simulink model "new_model"  (R2023a)
(part 2 of 4)

  RadarSensor:2.OBJ_S_Range_51 : Outport  Port=1335
  RadarSensor:2.OBJ_S_Range_52 : Outport  Port=1336
  RadarSensor:2.OBJ_S_Range_53 : Outport  Port=1337
  RadarSensor:2.OBJ_S_Range_54 : Outport  Port=1338
  RadarSensor:2.OBJ_S_Range_55 : Outport  Port=1339
  RadarSensor:2.OBJ_S_Range_56 : Outport  Port=1340
  RadarSensor:2.OBJ_S_Range_57 : Outport  Port=1341
  RadarSensor:2.OBJ_S_Range_58 : Outport  Port=1342
  RadarSensor:2.OBJ_S_Range_59 : Outport  Port=1343
  RadarSensor:2.OBJ_S_Range_60 : Outport  Port=1344
  RadarSensor:2.OBJ_S_Range_61 : Outport  Port=1345
  RadarSensor:2.OBJ_S_Range_62 : Outport  Port=1346
  RadarSensor:2.OBJ_S_Range_63 : Outport  Port=1347
  RadarSensor:2.OBJ_S_Range_64 : Outport  Port=1348
  RadarSensor:2.OBJ_RCS : Outport  Port=1349
  RadarSensor:2.OBJ_RCS_1 : Outport  Port=1350
  RadarSensor:2.OBJ_RCS_2 : Outport  Port=1351
  RadarSensor:2.OBJ_RCS_3 : Outport  Port=1352
  RadarSensor:2.OBJ_RCS_4 : Outport  Port=1353
  RadarSensor:2.OBJ_RCS_5 : Outport  Port=1354
  RadarSensor:2.OBJ_RCS_6 : Outport  Port=1355
  RadarSensor:2.OBJ_RCS_7 : Outport  Port=1356
  RadarSensor:2.OBJ_RCS_8 : Outport  Port=1357
  RadarSensor:2.OBJ_RCS_9 : Outport  Port=1358
  RadarSensor:2.OBJ_RCS_10 : Outport  Port=1359
  RadarSensor:2.OBJ_RCS_11 : Outport  Port=1360
  RadarSensor:2.OBJ_RCS_12 : Outport  Port=1361
  RadarSensor:2.OBJ_RCS_13 : Outport  Port=1362
  RadarSensor:2.OBJ_RCS_14 : Outport  Port=1363
  RadarSensor:2.OBJ_RCS_15 : Outport  Port=1364
  RadarSensor:2.OBJ_RCS_16 : Outport  Port=1365
  RadarSensor:2.OBJ_RCS_17 : Outport  Port=1366
  RadarSensor:2.OBJ_RCS_18 : Outport  Port=1367
  RadarSensor:2.OBJ_RCS_19 : Outport  Port=1368
  RadarSensor:2.OBJ_RCS_20 : Outport  Port=1369
  RadarSensor:2.OBJ_RCS_21 : Outport  Port=1370
  RadarSensor:2.OBJ_RCS_22 : Outport  Port=1371
  RadarSensor:2.OBJ_RCS_23 : Outport  Port=1372
  RadarSensor:2.OBJ_RCS_24 : Outport  Port=1373
  RadarSensor:2.OBJ_RCS_25 : Outport  Port=1374
  RadarSensor:2.OBJ_RCS_26 : Outport  Port=1375
  RadarSensor:2.OBJ_RCS_27 : Outport  Port=1376
  RadarSensor:2.OBJ_RCS_28 : Outport  Port=1377
  RadarSensor:2.OBJ_RCS_29 : Outport  Port=1378
  RadarSensor:2.OBJ_RCS_30 : Outport  Port=1379
  RadarSensor:2.OBJ_RCS_31 : Outport  Port=1380
  RadarSensor:2.OBJ_RCS_32 : Outport  Port=1381
  RadarSensor:2.OBJ_RCS_33 : Outport  Port=1382
  RadarSensor:2.OBJ_RCS_34 : Outport  Port=1383
  RadarSensor:2.OBJ_RCS_35 : Outport  Port=1384
  RadarSensor:2.OBJ_RCS_36 : Outport  Port=1385
  RadarSensor:2.OBJ_RCS_37 : Outport  Port=1386
  RadarSensor:2.OBJ_RCS_38 : Outport  Port=1387
  RadarSensor:2.OBJ_RCS_39 : Outport  Port=1388
  RadarSensor:2.OBJ_RCS_40 : Outport  Port=1389
  RadarSensor:2.OBJ_RCS_41 : Outport  Port=1390
  RadarSensor:2.OBJ_RCS_42 : Outport  Port=1391
  RadarSensor:2.OBJ_RCS_43 : Outport  Port=1392
  RadarSensor:2.OBJ_RCS_44 : Outport  Port=1393
  RadarSensor:2.OBJ_RCS_45 : Outport  Port=1394
  RadarSensor:2.OBJ_RCS_46 : Outport  Port=1395
  RadarSensor:2.OBJ_RCS_47 : Outport  Port=1396
  RadarSensor:2.OBJ_RCS_48 : Outport  Port=1397
  RadarSensor:2.OBJ_RCS_49 : Outport  Port=1398
  RadarSensor:2.OBJ_RCS_50 : Outport  Port=1399
  RadarSensor:2.OBJ_RCS_51 : Outport  Port=1400
  RadarSensor:2.OBJ_RCS_52 : Outport  Port=1401
  RadarSensor:2.OBJ_RCS_53 : Outport  Port=1402
  RadarSensor:2.OBJ_RCS_54 : Outport  Port=1403
  RadarSensor:2.OBJ_RCS_55 : Outport  Port=1404
  RadarSensor:2.OBJ_RCS_56 : Outport  Port=1405
  RadarSensor:2.OBJ_RCS_57 : Outport  Port=1406
  RadarSensor:2.OBJ_RCS_58 : Outport  Port=1407
  RadarSensor:2.OBJ_RCS_59 : Outport  Port=1408
  RadarSensor:2.OBJ_RCS_60 : Outport  Port=1409
  RadarSensor:2.OBJ_RCS_61 : Outport  Port=1410
  RadarSensor:2.OBJ_RCS_62 : Outport  Port=1411
  RadarSensor:2.OBJ_RCS_63 : Outport  Port=1412
  RadarSensor:2.OBJ_RCS_64 : Outport  Port=1413
  RadarSensor:3.time : Outport  Port=1414
  RadarSensor:3.width : Outport  Port=1415
  RadarSensor:3.OBJ_ID : Outport  Port=1416
  RadarSensor:3.OBJ_ID_1 : Outport  Port=1417
  RadarSensor:3.OBJ_ID_2 : Outport  Port=1418
  RadarSensor:3.OBJ_ID_3 : Outport  Port=1419
  RadarSensor:3.OBJ_ID_4 : Outport  Port=1420
  RadarSensor:3.OBJ_ID_5 : Outport  Port=1421
  RadarSensor:3.OBJ_ID_6 : Outport  Port=1422
  RadarSensor:3.OBJ_ID_7 : Outport  Port=1423
  RadarSensor:3.OBJ_ID_8 : Outport  Port=1424
  RadarSensor:3.OBJ_ID_9 : Outport  Port=1425
  RadarSensor:3.OBJ_ID_10 : Outport  Port=1426
  RadarSensor:3.OBJ_ID_11 : Outport  Port=1427
  RadarSensor:3.OBJ_ID_12 : Outport  Port=1428
  RadarSensor:3.OBJ_ID_13 : Outport  Port=1429
  RadarSensor:3.OBJ_ID_14 : Outport  Port=1430
  RadarSensor:3.OBJ_ID_15 : Outport  Port=1431
  RadarSensor:3.OBJ_ID_16 : Outport  Port=1432
  RadarSensor:3.OBJ_ID_17 : Outport  Port=1433
  RadarSensor:3.OBJ_ID_18 : Outport  Port=1434
  RadarSensor:3.OBJ_ID_19 : Outport  Port=1435
  RadarSensor:3.OBJ_ID_20 : Outport  Port=1436
  RadarSensor:3.OBJ_ID_21 : Outport  Port=1437
  RadarSensor:3.OBJ_ID_22 : Outport  Port=1438
  RadarSensor:3.OBJ_ID_23 : Outport  Port=1439
  RadarSensor:3.OBJ_ID_24 : Outport  Port=1440
  RadarSensor:3.OBJ_ID_25 : Outport  Port=1441
  RadarSensor:3.OBJ_ID_26 : Outport  Port=1442
  RadarSensor:3.OBJ_ID_27 : Outport  Port=1443
  RadarSensor:3.OBJ_ID_28 : Outport  Port=1444
  RadarSensor:3.OBJ_ID_29 : Outport  Port=1445
  RadarSensor:3.OBJ_ID_30 : Outport  Port=1446
  RadarSensor:3.OBJ_ID_31 : Outport  Port=1447
  RadarSensor:3.OBJ_ID_32 : Outport  Port=1448
  RadarSensor:3.OBJ_ID_33 : Outport  Port=1449
  RadarSensor:3.OBJ_ID_34 : Outport  Port=1450
  RadarSensor:3.OBJ_ID_35 : Outport  Port=1451
  RadarSensor:3.OBJ_ID_36 : Outport  Port=1452
  RadarSensor:3.OBJ_ID_37 : Outport  Port=1453
  RadarSensor:3.OBJ_ID_38 : Outport  Port=1454
  RadarSensor:3.OBJ_ID_39 : Outport  Port=1455
  RadarSensor:3.OBJ_ID_40 : Outport  Port=1456
  RadarSensor:3.OBJ_ID_41 : Outport  Port=1457
  RadarSensor:3.OBJ_ID_42 : Outport  Port=1458
  RadarSensor:3.OBJ_ID_43 : Outport  Port=1459
  RadarSensor:3.OBJ_ID_44 : Outport  Port=1460
  RadarSensor:3.OBJ_ID_45 : Outport  Port=1461
  RadarSensor:3.OBJ_ID_46 : Outport  Port=1462
  RadarSensor:3.OBJ_ID_47 : Outport  Port=1463
  RadarSensor:3.OBJ_ID_48 : Outport  Port=1464
  RadarSensor:3.OBJ_ID_49 : Outport  Port=1465
  RadarSensor:3.OBJ_ID_50 : Outport  Port=1466
  RadarSensor:3.OBJ_ID_51 : Outport  Port=1467
  RadarSensor:3.OBJ_ID_52 : Outport  Port=1468
  RadarSensor:3.OBJ_ID_53 : Outport  Port=1469
  RadarSensor:3.OBJ_ID_54 : Outport  Port=1470
  RadarSensor:3.OBJ_ID_55 : Outport  Port=1471
  RadarSensor:3.OBJ_ID_56 : Outport  Port=1472
  RadarSensor:3.OBJ_ID_57 : Outport  Port=1473
  RadarSensor:3.OBJ_ID_58 : Outport  Port=1474
  RadarSensor:3.OBJ_ID_59 : Outport  Port=1475
  RadarSensor:3.OBJ_ID_60 : Outport  Port=1476
  RadarSensor:3.OBJ_ID_61 : Outport  Port=1477
  RadarSensor:3.OBJ_ID_62 : Outport  Port=1478
  RadarSensor:3.OBJ_ID_63 : Outport  Port=1479
  RadarSensor:3.OBJ_ID_64 : Outport  Port=1480
  RadarSensor:3.OBJ_Class : Outport  Port=1481
  RadarSensor:3.OBJ_Class_1 : Outport  Port=1482
  RadarSensor:3.OBJ_Class_2 : Outport  Port=1483
  RadarSensor:3.OBJ_Class_3 : Outport  Port=1484
  RadarSensor:3.OBJ_Class_4 : Outport  Port=1485
  RadarSensor:3.OBJ_Class_5 : Outport  Port=1486
  RadarSensor:3.OBJ_Class_6 : Outport  Port=1487
  RadarSensor:3.OBJ_Class_7 : Outport  Port=1488
  RadarSensor:3.OBJ_Class_8 : Outport  Port=1489
  RadarSensor:3.OBJ_Class_9 : Outport  Port=1490
  RadarSensor:3.OBJ_Class_10 : Outport  Port=1491
  RadarSensor:3.OBJ_Class_11 : Outport  Port=1492
  RadarSensor:3.OBJ_Class_12 : Outport  Port=1493
  RadarSensor:3.OBJ_Class_13 : Outport  Port=1494
  RadarSensor:3.OBJ_Class_14 : Outport  Port=1495
  RadarSensor:3.OBJ_Class_15 : Outport  Port=1496
  RadarSensor:3.OBJ_Class_16 : Outport  Port=1497
  RadarSensor:3.OBJ_Class_17 : Outport  Port=1498
  RadarSensor:3.OBJ_Class_18 : Outport  Port=1499
  RadarSensor:3.OBJ_Class_19 : Outport  Port=1500
  RadarSensor:3.OBJ_Class_20 : Outport  Port=1501
  RadarSensor:3.OBJ_Class_21 : Outport  Port=1502
  RadarSensor:3.OBJ_Class_22 : Outport  Port=1503
  RadarSensor:3.OBJ_Class_23 : Outport  Port=1504
  RadarSensor:3.OBJ_Class_24 : Outport  Port=1505
  RadarSensor:3.OBJ_Class_25 : Outport  Port=1506
  RadarSensor:3.OBJ_Class_26 : Outport  Port=1507
  RadarSensor:3.OBJ_Class_27 : Outport  Port=1508
  RadarSensor:3.OBJ_Class_28 : Outport  Port=1509
  RadarSensor:3.OBJ_Class_29 : Outport  Port=1510
  RadarSensor:3.OBJ_Class_30 : Outport  Port=1511
  RadarSensor:3.OBJ_Class_31 : Outport  Port=1512
  RadarSensor:3.OBJ_Class_32 : Outport  Port=1513
  RadarSensor:3.OBJ_Class_33 : Outport  Port=1514
  RadarSensor:3.OBJ_Class_34 : Outport  Port=1515
  RadarSensor:3.OBJ_Class_35 : Outport  Port=1516
  RadarSensor:3.OBJ_Class_36 : Outport  Port=1517
  RadarSensor:3.OBJ_Class_37 : Outport  Port=1518
  RadarSensor:3.OBJ_Class_38 : Outport  Port=1519
  RadarSensor:3.OBJ_Class_39 : Outport  Port=1520
  RadarSensor:3.OBJ_Class_40 : Outport  Port=1521
  RadarSensor:3.OBJ_Class_41 : Outport  Port=1522
  RadarSensor:3.OBJ_Class_42 : Outport  Port=1523
  RadarSensor:3.OBJ_Class_43 : Outport  Port=1524
  RadarSensor:3.OBJ_Class_44 : Outport  Port=1525
  RadarSensor:3.OBJ_Class_45 : Outport  Port=1526
  RadarSensor:3.OBJ_Class_46 : Outport  Port=1527
  RadarSensor:3.OBJ_Class_47 : Outport  Port=1528
  RadarSensor:3.OBJ_Class_48 : Outport  Port=1529
  RadarSensor:3.OBJ_Class_49 : Outport  Port=1530
  RadarSensor:3.OBJ_Class_50 : Outport  Port=1531
  RadarSensor:3.OBJ_Class_51 : Outport  Port=1532
  RadarSensor:3.OBJ_Class_52 : Outport  Port=1533
  RadarSensor:3.OBJ_Class_53 : Outport  Port=1534
  RadarSensor:3.OBJ_Class_54 : Outport  Port=1535
  RadarSensor:3.OBJ_Class_55 : Outport  Port=1536
  RadarSensor:3.OBJ_Class_56 : Outport  Port=1537
  RadarSensor:3.OBJ_Class_57 : Outport  Port=1538
  RadarSensor:3.OBJ_Class_58 : Outport  Port=1539
  RadarSensor:3.OBJ_Class_59 : Outport  Port=1540
  RadarSensor:3.OBJ_Class_60 : Outport  Port=1541
  RadarSensor:3.OBJ_Class_61 : Outport  Port=1542
  RadarSensor:3.OBJ_Class_62 : Outport  Port=1543
  RadarSensor:3.OBJ_Class_63 : Outport  Port=1544
  RadarSensor:3.OBJ_Class_64 : Outport  Port=1545
  RadarSensor:3.OBJ_S_Azimuth : Outport  Port=1546
  RadarSensor:3.OBJ_S_Azimuth_1 : Outport  Port=1547
  RadarSensor:3.OBJ_S_Azimuth_2 : Outport  Port=1548
  RadarSensor:3.OBJ_S_Azimuth_3 : Outport  Port=1549
  RadarSensor:3.OBJ_S_Azimuth_4 : Outport  Port=1550
  RadarSensor:3.OBJ_S_Azimuth_5 : Outport  Port=1551
  RadarSensor:3.OBJ_S_Azimuth_6 : Outport  Port=1552
  RadarSensor:3.OBJ_S_Azimuth_7 : Outport  Port=1553
  RadarSensor:3.OBJ_S_Azimuth_8 : Outport  Port=1554
  RadarSensor:3.OBJ_S_Azimuth_9 : Outport  Port=1555
  RadarSensor:3.OBJ_S_Azimuth_10 : Outport  Port=1556
  RadarSensor:3.OBJ_S_Azimuth_11 : Outport  Port=1557
  RadarSensor:3.OBJ_S_Azimuth_12 : Outport  Port=1558
  RadarSensor:3.OBJ_S_Azimuth_13 : Outport  Port=1559
  RadarSensor:3.OBJ_S_Azimuth_14 : Outport  Port=1560
  RadarSensor:3.OBJ_S_Azimuth_15 : Outport  Port=1561
  RadarSensor:3.OBJ_S_Azimuth_16 : Outport  Port=1562
  RadarSensor:3.OBJ_S_Azimuth_17 : Outport  Port=1563
  RadarSensor:3.OBJ_S_Azimuth_18 : Outport  Port=1564
  RadarSensor:3.OBJ_S_Azimuth_19 : Outport  Port=1565
  RadarSensor:3.OBJ_S_Azimuth_20 : Outport  Port=1566
  RadarSensor:3.OBJ_S_Azimuth_21 : Outport  Port=1567
  RadarSensor:3.OBJ_S_Azimuth_22 : Outport  Port=1568
  RadarSensor:3.OBJ_S_Azimuth_23 : Outport  Port=1569
  RadarSensor:3.OBJ_S_Azimuth_24 : Outport  Port=1570
  RadarSensor:3.OBJ_S_Azimuth_25 : Outport  Port=1571
  RadarSensor:3.OBJ_S_Azimuth_26 : Outport  Port=1572
  RadarSensor:3.OBJ_S_Azimuth_27 : Outport  Port=1573
  RadarSensor:3.OBJ_S_Azimuth_28 : Outport  Port=1574
  RadarSensor:3.OBJ_S_Azimuth_29 : Outport  Port=1575
  RadarSensor:3.OBJ_S_Azimuth_30 : Outport  Port=1576
  RadarSensor:3.OBJ_S_Azimuth_31 : Outport  Port=1577
  RadarSensor:3.OBJ_S_Azimuth_32 : Outport  Port=1578
  RadarSensor:3.OBJ_S_Azimuth_33 : Outport  Port=1579
  RadarSensor:3.OBJ_S_Azimuth_34 : Outport  Port=1580
  RadarSensor:3.OBJ_S_Azimuth_35 : Outport  Port=1581
  RadarSensor:3.OBJ_S_Azimuth_36 : Outport  Port=1582
  RadarSensor:3.OBJ_S_Azimuth_37 : Outport  Port=1583
  RadarSensor:3.OBJ_S_Azimuth_38 : Outport  Port=1584
  RadarSensor:3.OBJ_S_Azimuth_39 : Outport  Port=1585
  RadarSensor:3.OBJ_S_Azimuth_40 : Outport  Port=1586
  RadarSensor:3.OBJ_S_Azimuth_41 : Outport  Port=1587
  RadarSensor:3.OBJ_S_Azimuth_42 : Outport  Port=1588
  RadarSensor:3.OBJ_S_Azimuth_43 : Outport  Port=1589
  RadarSensor:3.OBJ_S_Azimuth_44 : Outport  Port=1590
  RadarSensor:3.OBJ_S_Azimuth_45 : Outport  Port=1591
  RadarSensor:3.OBJ_S_Azimuth_46 : Outport  Port=1592
  RadarSensor:3.OBJ_S_Azimuth_47 : Outport  Port=1593
  RadarSensor:3.OBJ_S_Azimuth_48 : Outport  Port=1594
  RadarSensor:3.OBJ_S_Azimuth_49 : Outport  Port=1595
  RadarSensor:3.OBJ_S_Azimuth_50 : Outport  Port=1596
  RadarSensor:3.OBJ_S_Azimuth_51 : Outport  Port=1597
  RadarSensor:3.OBJ_S_Azimuth_52 : Outport  Port=1598
  RadarSensor:3.OBJ_S_Azimuth_53 : Outport  Port=1599
  RadarSensor:3.OBJ_S_Azimuth_54 : Outport  Port=1600
  RadarSensor:3.OBJ_S_Azimuth_55 : Outport  Port=1601
  RadarSensor:3.OBJ_S_Azimuth_56 : Outport  Port=1602
  RadarSensor:3.OBJ_S_Azimuth_57 : Outport  Port=1603
  RadarSensor:3.OBJ_S_Azimuth_58 : Outport  Port=1604
  RadarSensor:3.OBJ_S_Azimuth_59 : Outport  Port=1605
  RadarSensor:3.OBJ_S_Azimuth_60 : Outport  Port=1606
  RadarSensor:3.OBJ_S_Azimuth_61 : Outport  Port=1607
  RadarSensor:3.OBJ_S_Azimuth_62 : Outport  Port=1608
  RadarSensor:3.OBJ_S_Azimuth_63 : Outport  Port=1609
  RadarSensor:3.OBJ_S_Azimuth_64 : Outport  Port=1610
  RadarSensor:3.OBJ_S_Elevation : Outport  Port=1611
  RadarSensor:3.OBJ_S_Elevation_1 : Outport  Port=1612
  RadarSensor:3.OBJ_S_Elevation_2 : Outport  Port=1613
  RadarSensor:3.OBJ_S_Elevation_3 : Outport  Port=1614
  RadarSensor:3.OBJ_S_Elevation_4 : Outport  Port=1615
  RadarSensor:3.OBJ_S_Elevation_5 : Outport  Port=1616
  RadarSensor:3.OBJ_S_Elevation_6 : Outport  Port=1617
  RadarSensor:3.OBJ_S_Elevation_7 : Outport  Port=1618
  RadarSensor:3.OBJ_S_Elevation_8 : Outport  Port=1619
  RadarSensor:3.OBJ_S_Elevation_9 : Outport  Port=1620
  RadarSensor:3.OBJ_S_Elevation_10 : Outport  Port=1621
  RadarSensor:3.OBJ_S_Elevation_11 : Outport  Port=1622
  RadarSensor:3.OBJ_S_Elevation_12 : Outport  Port=1623
  RadarSensor:3.OBJ_S_Elevation_13 : Outport  Port=1624
  RadarSensor:3.OBJ_S_Elevation_14 : Outport  Port=1625
  RadarSensor:3.OBJ_S_Elevation_15 : Outport  Port=1626
  RadarSensor:3.OBJ_S_Elevation_16 : Outport  Port=1627
  RadarSensor:3.OBJ_S_Elevation_17 : Outport  Port=1628
  RadarSensor:3.OBJ_S_Elevation_18 : Outport  Port=1629
  RadarSensor:3.OBJ_S_Elevation_19 : Outport  Port=1630
  RadarSensor:3.OBJ_S_Elevation_20 : Outport  Port=1631
  RadarSensor:3.OBJ_S_Elevation_21 : Outport  Port=1632
  RadarSensor:3.OBJ_S_Elevation_22 : Outport  Port=1633
  RadarSensor:3.OBJ_S_Elevation_23 : Outport  Port=1634
  RadarSensor:3.OBJ_S_Elevation_24 : Outport  Port=1635
  RadarSensor:3.OBJ_S_Elevation_25 : Outport  Port=1636
  RadarSensor:3.OBJ_S_Elevation_26 : Outport  Port=1637
  RadarSensor:3.OBJ_S_Elevation_27 : Outport  Port=1638
  RadarSensor:3.OBJ_S_Elevation_28 : Outport  Port=1639
  RadarSensor:3.OBJ_S_Elevation_29 : Outport  Port=1640
  RadarSensor:3.OBJ_S_Elevation_30 : Outport  Port=1641
  RadarSensor:3.OBJ_S_Elevation_31 : Outport  Port=1642
  RadarSensor:3.OBJ_S_Elevation_32 : Outport  Port=1643
  RadarSensor:3.OBJ_S_Elevation_33 : Outport  Port=1644
  RadarSensor:3.OBJ_S_Elevation_34 : Outport  Port=1645
  RadarSensor:3.OBJ_S_Elevation_35 : Outport  Port=1646
  RadarSensor:3.OBJ_S_Elevation_36 : Outport  Port=1647
  RadarSensor:3.OBJ_S_Elevation_37 : Outport  Port=1648
  RadarSensor:3.OBJ_S_Elevation_38 : Outport  Port=1649
  RadarSensor:3.OBJ_S_Elevation_39 : Outport  Port=1650
  RadarSensor:3.OBJ_S_Elevation_40 : Outport  Port=1651
  RadarSensor:3.OBJ_S_Elevation_41 : Outport  Port=1652
  RadarSensor:3.OBJ_S_Elevation_42 : Outport  Port=1653
  RadarSensor:3.OBJ_S_Elevation_43 : Outport  Port=1654
  RadarSensor:3.OBJ_S_Elevation_44 : Outport  Port=1655
  RadarSensor:3.OBJ_S_Elevation_45 : Outport  Port=1656
  RadarSensor:3.OBJ_S_Elevation_46 : Outport  Port=1657
  RadarSensor:3.OBJ_S_Elevation_47 : Outport  Port=1658
  RadarSensor:3.OBJ_S_Elevation_48 : Outport  Port=1659
  RadarSensor:3.OBJ_S_Elevation_49 : Outport  Port=1660
  RadarSensor:3.OBJ_S_Elevation_50 : Outport  Port=1661
  RadarSensor:3.OBJ_S_Elevation_51 : Outport  Port=1662
  RadarSensor:3.OBJ_S_Elevation_52 : Outport  Port=1663
  RadarSensor:3.OBJ_S_Elevation_53 : Outport  Port=1664
  RadarSensor:3.OBJ_S_Elevation_54 : Outport  Port=1665
  RadarSensor:3.OBJ_S_Elevation_55 : Outport  Port=1666
  RadarSensor:3.OBJ_S_Elevation_56 : Outport  Port=1667
  RadarSensor:3.OBJ_S_Elevation_57 : Outport  Port=1668
  RadarSensor:3.OBJ_S_Elevation_58 : Outport  Port=1669
  RadarSensor:3.OBJ_S_Elevation_59 : Outport  Port=1670
  RadarSensor:3.OBJ_S_Elevation_60 : Outport  Port=1671
  RadarSensor:3.OBJ_S_Elevation_61 : Outport  Port=1672
  RadarSensor:3.OBJ_S_Elevation_62 : Outport  Port=1673
  RadarSensor:3.OBJ_S_Elevation_63 : Outport  Port=1674
  RadarSensor:3.OBJ_S_Elevation_64 : Outport  Port=1675
  RadarSensor:3.OBJ_S_Velocity : Outport  Port=1676
  RadarSensor:3.OBJ_S_Velocity_1 : Outport  Port=1677
  RadarSensor:3.OBJ_S_Velocity_2 : Outport  Port=1678
  RadarSensor:3.OBJ_S_Velocity_3 : Outport  Port=1679
  RadarSensor:3.OBJ_S_Velocity_4 : Outport  Port=1680
  RadarSensor:3.OBJ_S_Velocity_5 : Outport  Port=1681
  RadarSensor:3.OBJ_S_Velocity_6 : Outport  Port=1682
  RadarSensor:3.OBJ_S_Velocity_7 : Outport  Port=1683
  RadarSensor:3.OBJ_S_Velocity_8 : Outport  Port=1684
  RadarSensor:3.OBJ_S_Velocity_9 : Outport  Port=1685
  RadarSensor:3.OBJ_S_Velocity_10 : Outport  Port=1686
  RadarSensor:3.OBJ_S_Velocity_11 : Outport  Port=1687
  RadarSensor:3.OBJ_S_Velocity_12 : Outport  Port=1688
  RadarSensor:3.OBJ_S_Velocity_13 : Outport  Port=1689
  RadarSensor:3.OBJ_S_Velocity_14 : Outport  Port=1690
  RadarSensor:3.OBJ_S_Velocity_15 : Outport  Port=1691
  RadarSensor:3.OBJ_S_Velocity_16 : Outport  Port=1692
  RadarSensor:3.OBJ_S_Velocity_17 : Outport  Port=1693
  RadarSensor:3.OBJ_S_Velocity_18 : Outport  Port=1694
  RadarSensor:3.OBJ_S_Velocity_19 : Outport  Port=1695
  RadarSensor:3.OBJ_S_Velocity_20 : Outport  Port=1696
  RadarSensor:3.OBJ_S_Velocity_21 : Outport  Port=1697
  RadarSensor:3.OBJ_S_Velocity_22 : Outport  Port=1698
  RadarSensor:3.OBJ_S_Velocity_23 : Outport  Port=1699
  RadarSensor:3.OBJ_S_Velocity_24 : Outport  Port=1700
  RadarSensor:3.OBJ_S_Velocity_25 : Outport  Port=1701
  RadarSensor:3.OBJ_S_Velocity_26 : Outport  Port=1702
  RadarSensor:3.OBJ_S_Velocity_27 : Outport  Port=1703
  RadarSensor:3.OBJ_S_Velocity_28 : Outport  Port=1704
  RadarSensor:3.OBJ_S_Velocity_29 : Outport  Port=1705
  RadarSensor:3.OBJ_S_Velocity_30 : Outport  Port=1706
  RadarSensor:3.OBJ_S_Velocity_31 : Outport  Port=1707
  RadarSensor:3.OBJ_S_Velocity_32 : Outport  Port=1708
  RadarSensor:3.OBJ_S_Velocity_33 : Outport  Port=1709
  RadarSensor:3.OBJ_S_Velocity_34 : Outport  Port=1710
  RadarSensor:3.OBJ_S_Velocity_35 : Outport  Port=1711
  RadarSensor:3.OBJ_S_Velocity_36 : Outport  Port=1712
  RadarSensor:3.OBJ_S_Velocity_37 : Outport  Port=1713
  RadarSensor:3.OBJ_S_Velocity_38 : Outport  Port=1714
  RadarSensor:3.OBJ_S_Velocity_39 : Outport  Port=1715
  RadarSensor:3.OBJ_S_Velocity_40 : Outport  Port=1716
  RadarSensor:3.OBJ_S_Velocity_41 : Outport  Port=1717
  RadarSensor:3.OBJ_S_Velocity_42 : Outport  Port=1718
  RadarSensor:3.OBJ_S_Velocity_43 : Outport  Port=1719
  RadarSensor:3.OBJ_S_Velocity_44 : Outport  Port=1720
  RadarSensor:3.OBJ_S_Velocity_45 : Outport  Port=1721
  RadarSensor:3.OBJ_S_Velocity_46 : Outport  Port=1722
  RadarSensor:3.OBJ_S_Velocity_47 : Outport  Port=1723
  RadarSensor:3.OBJ_S_Velocity_48 : Outport  Port=1724
  RadarSensor:3.OBJ_S_Velocity_49 : Outport  Port=1725
  RadarSensor:3.OBJ_S_Velocity_50 : Outport  Port=1726
  RadarSensor:3.OBJ_S_Velocity_51 : Outport  Port=1727
  RadarSensor:3.OBJ_S_Velocity_52 : Outport  Port=1728
  RadarSensor:3.OBJ_S_Velocity_53 : Outport  Port=1729
  RadarSensor:3.OBJ_S_Velocity_54 : Outport  Port=1730
  RadarSensor:3.OBJ_S_Velocity_55 : Outport  Port=1731
  RadarSensor:3.OBJ_S_Velocity_56 : Outport  Port=1732
  RadarSensor:3.OBJ_S_Velocity_57 : Outport  Port=1733
  RadarSensor:3.OBJ_S_Velocity_58 : Outport  Port=1734
  RadarSensor:3.OBJ_S_Velocity_59 : Outport  Port=1735
  RadarSensor:3.OBJ_S_Velocity_60 : Outport  Port=1736
  RadarSensor:3.OBJ_S_Velocity_61 : Outport  Port=1737
  RadarSensor:3.OBJ_S_Velocity_62 : Outport  Port=1738
  RadarSensor:3.OBJ_S_Velocity_63 : Outport  Port=1739
  RadarSensor:3.OBJ_S_Velocity_64 : Outport  Port=1740
  RadarSensor:3.OBJ_S_Range : Outport  Port=1741
  RadarSensor:3.OBJ_S_Range_1 : Outport  Port=1742
  RadarSensor:3.OBJ_S_Range_2 : Outport  Port=1743
  RadarSensor:3.OBJ_S_Range_3 : Outport  Port=1744
  RadarSensor:3.OBJ_S_Range_4 : Outport  Port=1745
  RadarSensor:3.OBJ_S_Range_5 : Outport  Port=1746
  RadarSensor:3.OBJ_S_Range_6 : Outport  Port=1747
  RadarSensor:3.OBJ_S_Range_7 : Outport  Port=1748
  RadarSensor:3.OBJ_S_Range_8 : Outport  Port=1749
  RadarSensor:3.OBJ_S_Range_9 : Outport  Port=1750
  RadarSensor:3.OBJ_S_Range_10 : Outport  Port=1751
  RadarSensor:3.OBJ_S_Range_11 : Outport  Port=1752
  RadarSensor:3.OBJ_S_Range_12 : Outport  Port=1753
  RadarSensor:3.OBJ_S_Range_13 : Outport  Port=1754
  RadarSensor:3.OBJ_S_Range_14 : Outport  Port=1755
  RadarSensor:3.OBJ_S_Range_15 : Outport  Port=1756
  RadarSensor:3.OBJ_S_Range_16 : Outport  Port=1757
  RadarSensor:3.OBJ_S_Range_17 : Outport  Port=1758
  RadarSensor:3.OBJ_S_Range_18 : Outport  Port=1759
  RadarSensor:3.OBJ_S_Range_19 : Outport  Port=1760
  RadarSensor:3.OBJ_S_Range_20 : Outport  Port=1761
  RadarSensor:3.OBJ_S_Range_21 : Outport  Port=1762
  RadarSensor:3.OBJ_S_Range_22 : Outport  Port=1763
  RadarSensor:3.OBJ_S_Range_23 : Outport  Port=1764
  RadarSensor:3.OBJ_S_Range_24 : Outport  Port=1765
  RadarSensor:3.OBJ_S_Range_25 : Outport  Port=1766
  RadarSensor:3.OBJ_S_Range_26 : Outport  Port=1767
  RadarSensor:3.OBJ_S_Range_27 : Outport  Port=1768
  RadarSensor:3.OBJ_S_Range_28 : Outport  Port=1769
  RadarSensor:3.OBJ_S_Range_29 : Outport  Port=1770
  RadarSensor:3.OBJ_S_Range_30 : Outport  Port=1771
  RadarSensor:3.OBJ_S_Range_31 : Outport  Port=1772
  RadarSensor:3.OBJ_S_Range_32 : Outport  Port=1773
  RadarSensor:3.OBJ_S_Range_33 : Outport  Port=1774
  RadarSensor:3.OBJ_S_Range_34 : Outport  Port=1775
  RadarSensor:3.OBJ_S_Range_35 : Outport  Port=1776
  RadarSensor:3.OBJ_S_Range_36 : Outport  Port=1777
  RadarSensor:3.OBJ_S_Range_37 : Outport  Port=1778
  RadarSensor:3.OBJ_S_Range_38 : Outport  Port=1779
  RadarSensor:3.OBJ_S_Range_39 : Outport  Port=1780
  RadarSensor:3.OBJ_S_Range_40 : Outport  Port=1781
  RadarSensor:3.OBJ_S_Range_41 : Outport  Port=1782
  RadarSensor:3.OBJ_S_Range_42 : Outport  Port=1783
  RadarSensor:3.OBJ_S_Range_43 : Outport  Port=1784
  RadarSensor:3.OBJ_S_Range_44 : Outport  Port=1785
  RadarSensor:3.OBJ_S_Range_45 : Outport  Port=1786
  RadarSensor:3.OBJ_S_Range_46 : Outport  Port=1787
  RadarSensor:3.OBJ_S_Range_47 : Outport  Port=1788
  RadarSensor:3.OBJ_S_Range_48 : Outport  Port=1789
  RadarSensor:3.OBJ_S_Range_49 : Outport  Port=1790
  RadarSensor:3.OBJ_S_Range_50 : Outport  Port=1791
  RadarSensor:3.OBJ_S_Range_51 : Outport  Port=1792
  RadarSensor:3.OBJ_S_Range_52 : Outport  Port=1793
  RadarSensor:3.OBJ_S_Range_53 : Outport  Port=1794
  RadarSensor:3.OBJ_S_Range_54 : Outport  Port=1795
  RadarSensor:3.OBJ_S_Range_55 : Outport  Port=1796
  RadarSensor:3.OBJ_S_Range_56 : Outport  Port=1797
  RadarSensor:3.OBJ_S_Range_57 : Outport  Port=1798
  RadarSensor:3.OBJ_S_Range_58 : Outport  Port=1799
  RadarSensor:3.OBJ_S_Range_59 : Outport  Port=1800
  RadarSensor:3.OBJ_S_Range_60 : Outport  Port=1801
  RadarSensor:3.OBJ_S_Range_61 : Outport  Port=1802
  RadarSensor:3.OBJ_S_Range_62 : Outport  Port=1803
  RadarSensor:3.OBJ_S_Range_63 : Outport  Port=1804
  RadarSensor:3.OBJ_S_Range_64 : Outport  Port=1805
  RadarSensor:3.OBJ_RCS : Outport  Port=1806
  RadarSensor:3.OBJ_RCS_1 : Outport  Port=1807
  RadarSensor:3.OBJ_RCS_2 : Outport  Port=1808
  RadarSensor:3.OBJ_RCS_3 : Outport  Port=1809
  RadarSensor:3.OBJ_RCS_4 : Outport  Port=1810
  RadarSensor:3.OBJ_RCS_5 : Outport  Port=1811
  RadarSensor:3.OBJ_RCS_6 : Outport  Port=1812
  RadarSensor:3.OBJ_RCS_7 : Outport  Port=1813
  RadarSensor:3.OBJ_RCS_8 : Outport  Port=1814
  RadarSensor:3.OBJ_RCS_9 : Outport  Port=1815
  RadarSensor:3.OBJ_RCS_10 : Outport  Port=1816
  RadarSensor:3.OBJ_RCS_11 : Outport  Port=1817
  RadarSensor:3.OBJ_RCS_12 : Outport  Port=1818
  RadarSensor:3.OBJ_RCS_13 : Outport  Port=1819
  RadarSensor:3.OBJ_RCS_14 : Outport  Port=1820
  RadarSensor:3.OBJ_RCS_15 : Outport  Port=1821
  RadarSensor:3.OBJ_RCS_16 : Outport  Port=1822
  RadarSensor:3.OBJ_RCS_17 : Outport  Port=1823
  RadarSensor:3.OBJ_RCS_18 : Outport  Port=1824
  RadarSensor:3.OBJ_RCS_19 : Outport  Port=1825
  RadarSensor:3.OBJ_RCS_20 : Outport  Port=1826
  RadarSensor:3.OBJ_RCS_21 : Outport  Port=1827
  RadarSensor:3.OBJ_RCS_22 : Outport  Port=1828
  RadarSensor:3.OBJ_RCS_23 : Outport  Port=1829
  RadarSensor:3.OBJ_RCS_24 : Outport  Port=1830
  RadarSensor:3.OBJ_RCS_25 : Outport  Port=1831
  RadarSensor:3.OBJ_RCS_26 : Outport  Port=1832
  RadarSensor:3.OBJ_RCS_27 : Outport  Port=1833
  RadarSensor:3.OBJ_RCS_28 : Outport  Port=1834
  RadarSensor:3.OBJ_RCS_29 : Outport  Port=1835
  RadarSensor:3.OBJ_RCS_30 : Outport  Port=1836
  RadarSensor:3.OBJ_RCS_31 : Outport  Port=1837
  RadarSensor:3.OBJ_RCS_32 : Outport  Port=1838
  RadarSensor:3.OBJ_RCS_33 : Outport  Port=1839
  RadarSensor:3.OBJ_RCS_34 : Outport  Port=1840
  RadarSensor:3.OBJ_RCS_35 : Outport  Port=1841
  RadarSensor:3.OBJ_RCS_36 : Outport  Port=1842
  RadarSensor:3.OBJ_RCS_37 : Outport  Port=1843
  RadarSensor:3.OBJ_RCS_38 : Outport  Port=1844
  RadarSensor:3.OBJ_RCS_39 : Outport  Port=1845
  RadarSensor:3.OBJ_RCS_40 : Outport  Port=1846
  RadarSensor:3.OBJ_RCS_41 : Outport  Port=1847
  RadarSensor:3.OBJ_RCS_42 : Outport  Port=1848
  RadarSensor:3.OBJ_RCS_43 : Outport  Port=1849
  RadarSensor:3.OBJ_RCS_44 : Outport  Port=1850
  RadarSensor:3.OBJ_RCS_45 : Outport  Port=1851
  RadarSensor:3.OBJ_RCS_46 : Outport  Port=1852
  RadarSensor:3.OBJ_RCS_47 : Outport  Port=1853
  RadarSensor:3.OBJ_RCS_48 : Outport  Port=1854
  RadarSensor:3.OBJ_RCS_49 : Outport  Port=1855
  RadarSensor:3.OBJ_RCS_50 : Outport  Port=1856
  RadarSensor:3.OBJ_RCS_51 : Outport  Port=1857
  RadarSensor:3.OBJ_RCS_52 : Outport  Port=1858
  RadarSensor:3.OBJ_RCS_53 : Outport  Port=1859
  RadarSensor:3.OBJ_RCS_54 : Outport  Port=1860
  RadarSensor:3.OBJ_RCS_55 : Outport  Port=1861
  RadarSensor:3.OBJ_RCS_56 : Outport  Port=1862
  RadarSensor:3.OBJ_RCS_57 : Outport  Port=1863
  RadarSensor:3.OBJ_RCS_58 : Outport  Port=1864
  RadarSensor:3.OBJ_RCS_59 : Outport  Port=1865
  RadarSensor:3.OBJ_RCS_60 : Outport  Port=1866
  RadarSensor:3.OBJ_RCS_61 : Outport  Port=1867
  RadarSensor:3.OBJ_RCS_62 : Outport  Port=1868
  RadarSensor:3.OBJ_RCS_63 : Outport  Port=1869
  RadarSensor:3.OBJ_RCS_64 : Outport  Port=1870
  RadarSensor:4.time : Outport  Port=1871
  RadarSensor:4.width : Outport  Port=1872
  RadarSensor:4.OBJ_ID : Outport  Port=1873
  RadarSensor:4.OBJ_ID_1 : Outport  Port=1874
  RadarSensor:4.OBJ_ID_2 : Outport  Port=1875
  RadarSensor:4.OBJ_ID_3 : Outport  Port=1876
  RadarSensor:4.OBJ_ID_4 : Outport  Port=1877
  RadarSensor:4.OBJ_ID_5 : Outport  Port=1878
  RadarSensor:4.OBJ_ID_6 : Outport  Port=1879
  RadarSensor:4.OBJ_ID_7 : Outport  Port=1880
  RadarSensor:4.OBJ_ID_8 : Outport  Port=1881
  RadarSensor:4.OBJ_ID_9 : Outport  Port=1882
  RadarSensor:4.OBJ_ID_10 : Outport  Port=1883
  RadarSensor:4.OBJ_ID_11 : Outport  Port=1884
  RadarSensor:4.OBJ_ID_12 : Outport  Port=1885
  RadarSensor:4.OBJ_ID_13 : Outport  Port=1886
  RadarSensor:4.OBJ_ID_14 : Outport  Port=1887
  RadarSensor:4.OBJ_ID_15 : Outport  Port=1888
  RadarSensor:4.OBJ_ID_16 : Outport  Port=1889
  RadarSensor:4.OBJ_ID_17 : Outport  Port=1890
  RadarSensor:4.OBJ_ID_18 : Outport  Port=1891
  RadarSensor:4.OBJ_ID_19 : Outport  Port=1892
  RadarSensor:4.OBJ_ID_20 : Outport  Port=1893
  RadarSensor:4.OBJ_ID_21 : Outport  Port=1894
  RadarSensor:4.OBJ_ID_22 : Outport  Port=1895
  RadarSensor:4.OBJ_ID_23 : Outport  Port=1896
  RadarSensor:4.OBJ_ID_24 : Outport  Port=1897
  RadarSensor:4.OBJ_ID_25 : Outport  Port=1898
  RadarSensor:4.OBJ_ID_26 : Outport  Port=1899
  RadarSensor:4.OBJ_ID_27 : Outport  Port=1900
  RadarSensor:4.OBJ_ID_28 : Outport  Port=1901
  RadarSensor:4.OBJ_ID_29 : Outport  Port=1902
  RadarSensor:4.OBJ_ID_30 : Outport  Port=1903
  RadarSensor:4.OBJ_ID_31 : Outport  Port=1904
  RadarSensor:4.OBJ_ID_32 : Outport  Port=1905
  RadarSensor:4.OBJ_ID_33 : Outport  Port=1906
  RadarSensor:4.OBJ_ID_34 : Outport  Port=1907
  RadarSensor:4.OBJ_ID_35 : Outport  Port=1908
  RadarSensor:4.OBJ_ID_36 : Outport  Port=1909
  RadarSensor:4.OBJ_ID_37 : Outport  Port=1910
  RadarSensor:4.OBJ_ID_38 : Outport  Port=1911
  RadarSensor:4.OBJ_ID_39 : Outport  Port=1912
  RadarSensor:4.OBJ_ID_40 : Outport  Port=1913
  RadarSensor:4.OBJ_ID_41 : Outport  Port=1914
  RadarSensor:4.OBJ_ID_42 : Outport  Port=1915
  RadarSensor:4.OBJ_ID_43 : Outport  Port=1916
  RadarSensor:4.OBJ_ID_44 : Outport  Port=1917
  RadarSensor:4.OBJ_ID_45 : Outport  Port=1918
  RadarSensor:4.OBJ_ID_46 : Outport  Port=1919
  RadarSensor:4.OBJ_ID_47 : Outport  Port=1920
  RadarSensor:4.OBJ_ID_48 : Outport  Port=1921
  RadarSensor:4.OBJ_ID_49 : Outport  Port=1922
  RadarSensor:4.OBJ_ID_50 : Outport  Port=1923
  RadarSensor:4.OBJ_ID_51 : Outport  Port=1924
  RadarSensor:4.OBJ_ID_52 : Outport  Port=1925
  RadarSensor:4.OBJ_ID_53 : Outport  Port=1926
  RadarSensor:4.OBJ_ID_54 : Outport  Port=1927
  RadarSensor:4.OBJ_ID_55 : Outport  Port=1928
  RadarSensor:4.OBJ_ID_56 : Outport  Port=1929
  RadarSensor:4.OBJ_ID_57 : Outport  Port=1930
  RadarSensor:4.OBJ_ID_58 : Outport  Port=1931
  RadarSensor:4.OBJ_ID_59 : Outport  Port=1932
  RadarSensor:4.OBJ_ID_60 : Outport  Port=1933
  RadarSensor:4.OBJ_ID_61 : Outport  Port=1934
  RadarSensor:4.OBJ_ID_62 : Outport  Port=1935
  RadarSensor:4.OBJ_ID_63 : Outport  Port=1936
  RadarSensor:4.OBJ_ID_64 : Outport  Port=1937
  RadarSensor:4.OBJ_Class : Outport  Port=1938
  RadarSensor:4.OBJ_Class_1 : Outport  Port=1939
  RadarSensor:4.OBJ_Class_2 : Outport  Port=1940
  RadarSensor:4.OBJ_Class_3 : Outport  Port=1941
  RadarSensor:4.OBJ_Class_4 : Outport  Port=1942
  RadarSensor:4.OBJ_Class_5 : Outport  Port=1943
  RadarSensor:4.OBJ_Class_6 : Outport  Port=1944
  RadarSensor:4.OBJ_Class_7 : Outport  Port=1945
  RadarSensor:4.OBJ_Class_8 : Outport  Port=1946
  RadarSensor:4.OBJ_Class_9 : Outport  Port=1947
  RadarSensor:4.OBJ_Class_10 : Outport  Port=1948
  RadarSensor:4.OBJ_Class_11 : Outport  Port=1949
  RadarSensor:4.OBJ_Class_12 : Outport  Port=1950
  RadarSensor:4.OBJ_Class_13 : Outport  Port=1951
  RadarSensor:4.OBJ_Class_14 : Outport  Port=1952
  RadarSensor:4.OBJ_Class_15 : Outport  Port=1953
  RadarSensor:4.OBJ_Class_16 : Outport  Port=1954
  RadarSensor:4.OBJ_Class_17 : Outport  Port=1955
  RadarSensor:4.OBJ_Class_18 : Outport  Port=1956
  RadarSensor:4.OBJ_Class_19 : Outport  Port=1957
  RadarSensor:4.OBJ_Class_20 : Outport  Port=1958
  RadarSensor:4.OBJ_Class_21 : Outport  Port=1959
  RadarSensor:4.OBJ_Class_22 : Outport  Port=1960
  RadarSensor:4.OBJ_Class_23 : Outport  Port=1961
  RadarSensor:4.OBJ_Class_24 : Outport  Port=1962
  RadarSensor:4.OBJ_Class_25 : Outport  Port=1963
  RadarSensor:4.OBJ_Class_26 : Outport  Port=1964
  RadarSensor:4.OBJ_Class_27 : Outport  Port=1965
  RadarSensor:4.OBJ_Class_28 : Outport  Port=1966
  RadarSensor:4.OBJ_Class_29 : Outport  Port=1967
  RadarSensor:4.OBJ_Class_30 : Outport  Port=1968
  RadarSensor:4.OBJ_Class_31 : Outport  Port=1969
  RadarSensor:4.OBJ_Class_32 : Outport  Port=1970
  RadarSensor:4.OBJ_Class_33 : Outport  Port=1971
  RadarSensor:4.OBJ_Class_34 : Outport  Port=1972
  RadarSensor:4.OBJ_Class_35 : Outport  Port=1973
  RadarSensor:4.OBJ_Class_36 : Outport  Port=1974
  RadarSensor:4.OBJ_Class_37 : Outport  Port=1975
  RadarSensor:4.OBJ_Class_38 : Outport  Port=1976
  RadarSensor:4.OBJ_Class_39 : Outport  Port=1977
  RadarSensor:4.OBJ_Class_40 : Outport  Port=1978
  RadarSensor:4.OBJ_Class_41 : Outport  Port=1979
  RadarSensor:4.OBJ_Class_42 : Outport  Port=1980
  RadarSensor:4.OBJ_Class_43 : Outport  Port=1981
  RadarSensor:4.OBJ_Class_44 : Outport  Port=1982
  RadarSensor:4.OBJ_Class_45 : Outport  Port=1983
  RadarSensor:4.OBJ_Class_46 : Outport  Port=1984
  RadarSensor:4.OBJ_Class_47 : Outport  Port=1985
  RadarSensor:4.OBJ_Class_48 : Outport  Port=1986
  RadarSensor:4.OBJ_Class_49 : Outport  Port=1987
  RadarSensor:4.OBJ_Class_50 : Outport  Port=1988
  RadarSensor:4.OBJ_Class_51 : Outport  Port=1989
  RadarSensor:4.OBJ_Class_52 : Outport  Port=1990
  RadarSensor:4.OBJ_Class_53 : Outport  Port=1991
  RadarSensor:4.OBJ_Class_54 : Outport  Port=1992
  RadarSensor:4.OBJ_Class_55 : Outport  Port=1993
  RadarSensor:4.OBJ_Class_56 : Outport  Port=1994
  RadarSensor:4.OBJ_Class_57 : Outport  Port=1995
  RadarSensor:4.OBJ_Class_58 : Outport  Port=1996
  RadarSensor:4.OBJ_Class_59 : Outport  Port=1997
  RadarSensor:4.OBJ_Class_60 : Outport  Port=1998
  RadarSensor:4.OBJ_Class_61 : Outport  Port=1999
  RadarSensor:4.OBJ_Class_62 : Outport  Port=2000
  RadarSensor:4.OBJ_Class_63 : Outport  Port=2001
  RadarSensor:4.OBJ_Class_64 : Outport  Port=2002
  RadarSensor:4.OBJ_S_Azimuth : Outport  Port=2003
  RadarSensor:4.OBJ_S_Azimuth_1 : Outport  Port=2004
  RadarSensor:4.OBJ_S_Azimuth_2 : Outport  Port=2005
  RadarSensor:4.OBJ_S_Azimuth_3 : Outport  Port=2006
  RadarSensor:4.OBJ_S_Azimuth_4 : Outport  Port=2007
  RadarSensor:4.OBJ_S_Azimuth_5 : Outport  Port=2008
  RadarSensor:4.OBJ_S_Azimuth_6 : Outport  Port=2009
  RadarSensor:4.OBJ_S_Azimuth_7 : Outport  Port=2010
  RadarSensor:4.OBJ_S_Azimuth_8 : Outport  Port=2011
  RadarSensor:4.OBJ_S_Azimuth_9 : Outport  Port=2012
  RadarSensor:4.OBJ_S_Azimuth_10 : Outport  Port=2013
  RadarSensor:4.OBJ_S_Azimuth_11 : Outport  Port=2014
  RadarSensor:4.OBJ_S_Azimuth_12 : Outport  Port=2015
  RadarSensor:4.OBJ_S_Azimuth_13 : Outport  Port=2016
  RadarSensor:4.OBJ_S_Azimuth_14 : Outport  Port=2017
  RadarSensor:4.OBJ_S_Azimuth_15 : Outport  Port=2018
  RadarSensor:4.OBJ_S_Azimuth_16 : Outport  Port=2019
  RadarSensor:4.OBJ_S_Azimuth_17 : Outport  Port=2020
  RadarSensor:4.OBJ_S_Azimuth_18 : Outport  Port=2021
  RadarSensor:4.OBJ_S_Azimuth_19 : Outport  Port=2022
  RadarSensor:4.OBJ_S_Azimuth_20 : Outport  Port=2023
  RadarSensor:4.OBJ_S_Azimuth_21 : Outport  Port=2024
  RadarSensor:4.OBJ_S_Azimuth_22 : Outport  Port=2025
  RadarSensor:4.OBJ_S_Azimuth_23 : Outport  Port=2026
  RadarSensor:4.OBJ_S_Azimuth_24 : Outport  Port=2027
  RadarSensor:4.OBJ_S_Azimuth_25 : Outport  Port=2028
  RadarSensor:4.OBJ_S_Azimuth_26 : Outport  Port=2029
  RadarSensor:4.OBJ_S_Azimuth_27 : Outport  Port=2030
  RadarSensor:4.OBJ_S_Azimuth_28 : Outport  Port=2031
  RadarSensor:4.OBJ_S_Azimuth_29 : Outport  Port=2032
  RadarSensor:4.OBJ_S_Azimuth_30 : Outport  Port=2033
  RadarSensor:4.OBJ_S_Azimuth_31 : Outport  Port=2034
  RadarSensor:4.OBJ_S_Azimuth_32 : Outport  Port=2035
  RadarSensor:4.OBJ_S_Azimuth_33 : Outport  Port=2036
  RadarSensor:4.OBJ_S_Azimuth_34 : Outport  Port=2037
  RadarSensor:4.OBJ_S_Azimuth_35 : Outport  Port=2038
  RadarSensor:4.OBJ_S_Azimuth_36 : Outport  Port=2039
  RadarSensor:4.OBJ_S_Azimuth_37 : Outport  Port=2040
  RadarSensor:4.OBJ_S_Azimuth_38 : Outport  Port=2041
  RadarSensor:4.OBJ_S_Azimuth_39 : Outport  Port=2042
  RadarSensor:4.OBJ_S_Azimuth_40 : Outport  Port=2043
  RadarSensor:4.OBJ_S_Azimuth_41 : Outport  Port=2044
  RadarSensor:4.OBJ_S_Azimuth_42 : Outport  Port=2045
  RadarSensor:4.OBJ_S_Azimuth_43 : Outport  Port=2046
  RadarSensor:4.OBJ_S_Azimuth_44 : Outport  Port=2047
  RadarSensor:4.OBJ_S_Azimuth_45 : Outport  Port=2048
  RadarSensor:4.OBJ_S_Azimuth_46 : Outport  Port=2049
  RadarSensor:4.OBJ_S_Azimuth_47 : Outport  Port=2050
  RadarSensor:4.OBJ_S_Azimuth_48 : Outport  Port=2051
  RadarSensor:4.OBJ_S_Azimuth_49 : Outport  Port=2052
  RadarSensor:4.OBJ_S_Azimuth_50 : Outport  Port=2053
  RadarSensor:4.OBJ_S_Azimuth_51 : Outport  Port=2054
  RadarSensor:4.OBJ_S_Azimuth_52 : Outport  Port=2055
  RadarSensor:4.OBJ_S_Azimuth_53 : Outport  Port=2056
  RadarSensor:4.OBJ_S_Azimuth_54 : Outport  Port=2057
  RadarSensor:4.OBJ_S_Azimuth_55 : Outport  Port=2058
  RadarSensor:4.OBJ_S_Azimuth_56 : Outport  Port=2059
  RadarSensor:4.OBJ_S_Azimuth_57 : Outport  Port=2060
  RadarSensor:4.OBJ_S_Azimuth_58 : Outport  Port=2061
  RadarSensor:4.OBJ_S_Azimuth_59 : Outport  Port=2062
  RadarSensor:4.OBJ_S_Azimuth_60 : Outport  Port=2063
  RadarSensor:4.OBJ_S_Azimuth_61 : Outport  Port=2064
  RadarSensor:4.OBJ_S_Azimuth_62 : Outport  Port=2065
  RadarSensor:4.OBJ_S_Azimuth_63 : Outport  Port=2066
  RadarSensor:4.OBJ_S_Azimuth_64 : Outport  Port=2067
  RadarSensor:4.OBJ_S_Elevation : Outport  Port=2068
  RadarSensor:4.OBJ_S_Elevation_1 : Outport  Port=2069
  RadarSensor:4.OBJ_S_Elevation_2 : Outport  Port=2070
  RadarSensor:4.OBJ_S_Elevation_3 : Outport  Port=2071
  RadarSensor:4.OBJ_S_Elevation_4 : Outport  Port=2072
  RadarSensor:4.OBJ_S_Elevation_5 : Outport  Port=2073
  RadarSensor:4.OBJ_S_Elevation_6 : Outport  Port=2074
  RadarSensor:4.OBJ_S_Elevation_7 : Outport  Port=2075
  RadarSensor:4.OBJ_S_Elevation_8 : Outport  Port=2076
  RadarSensor:4.OBJ_S_Elevation_9 : Outport  Port=2077
  RadarSensor:4.OBJ_S_Elevation_10 : Outport  Port=2078
  RadarSensor:4.OBJ_S_Elevation_11 : Outport  Port=2079
  RadarSensor:4.OBJ_S_Elevation_12 : Outport  Port=2080
  RadarSensor:4.OBJ_S_Elevation_13 : Outport  Port=2081
  RadarSensor:4.OBJ_S_Elevation_14 : Outport  Port=2082
  RadarSensor:4.OBJ_S_Elevation_15 : Outport  Port=2083
  RadarSensor:4.OBJ_S_Elevation_16 : Outport  Port=2084
  RadarSensor:4.OBJ_S_Elevation_17 : Outport  Port=2085
  RadarSensor:4.OBJ_S_Elevation_18 : Outport  Port=2086
  RadarSensor:4.OBJ_S_Elevation_19 : Outport  Port=2087
  RadarSensor:4.OBJ_S_Elevation_20 : Outport  Port=2088
  RadarSensor:4.OBJ_S_Elevation_21 : Outport  Port=2089
  RadarSensor:4.OBJ_S_Elevation_22 : Outport  Port=2090
  RadarSensor:4.OBJ_S_Elevation_23 : Outport  Port=2091
  RadarSensor:4.OBJ_S_Elevation_24 : Outport  Port=2092
  RadarSensor:4.OBJ_S_Elevation_25 : Outport  Port=2093
  RadarSensor:4.OBJ_S_Elevation_26 : Outport  Port=2094
  RadarSensor:4.OBJ_S_Elevation_27 : Outport  Port=2095
  RadarSensor:4.OBJ_S_Elevation_28 : Outport  Port=2096
  RadarSensor:4.OBJ_S_Elevation_29 : Outport  Port=2097
  RadarSensor:4.OBJ_S_Elevation_30 : Outport  Port=2098
  RadarSensor:4.OBJ_S_Elevation_31 : Outport  Port=2099
  RadarSensor:4.OBJ_S_Elevation_32 : Outport  Port=2100
  RadarSensor:4.OBJ_S_Elevation_33 : Outport  Port=2101
  RadarSensor:4.OBJ_S_Elevation_34 : Outport  Port=2102
  RadarSensor:4.OBJ_S_Elevation_35 : Outport  Port=2103
  RadarSensor:4.OBJ_S_Elevation_36 : Outport  Port=2104
  RadarSensor:4.OBJ_S_Elevation_37 : Outport  Port=2105
  RadarSensor:4.OBJ_S_Elevation_38 : Outport  Port=2106
  RadarSensor:4.OBJ_S_Elevation_39 : Outport  Port=2107
  RadarSensor:4.OBJ_S_Elevation_40 : Outport  Port=2108
  RadarSensor:4.OBJ_S_Elevation_41 : Outport  Port=2109
  RadarSensor:4.OBJ_S_Elevation_42 : Outport  Port=2110
  RadarSensor:4.OBJ_S_Elevation_43 : Outport  Port=2111
  RadarSensor:4.OBJ_S_Elevation_44 : Outport  Port=2112
  RadarSensor:4.OBJ_S_Elevation_45 : Outport  Port=2113
  RadarSensor:4.OBJ_S_Elevation_46 : Outport  Port=2114
  RadarSensor:4.OBJ_S_Elevation_47 : Outport  Port=2115
  RadarSensor:4.OBJ_S_Elevation_48 : Outport  Port=2116
  RadarSensor:4.OBJ_S_Elevation_49 : Outport  Port=2117
  RadarSensor:4.OBJ_S_Elevation_50 : Outport  Port=2118
  RadarSensor:4.OBJ_S_Elevation_51 : Outport  Port=2119
  RadarSensor:4.OBJ_S_Elevation_52 : Outport  Port=2120
  RadarSensor:4.OBJ_S_Elevation_53 : Outport  Port=2121
  RadarSensor:4.OBJ_S_Elevation_54 : Outport  Port=2122
  RadarSensor:4.OBJ_S_Elevation_55 : Outport  Port=2123
  RadarSensor:4.OBJ_S_Elevation_56 : Outport  Port=2124
  RadarSensor:4.OBJ_S_Elevation_57 : Outport  Port=2125
  RadarSensor:4.OBJ_S_Elevation_58 : Outport  Port=2126
  RadarSensor:4.OBJ_S_Elevation_59 : Outport  Port=2127
  RadarSensor:4.OBJ_S_Elevation_60 : Outport  Port=2128
  RadarSensor:4.OBJ_S_Elevation_61 : Outport  Port=2129
  RadarSensor:4.OBJ_S_Elevation_62 : Outport  Port=2130
  RadarSensor:4.OBJ_S_Elevation_63 : Outport  Port=2131
  RadarSensor:4.OBJ_S_Elevation_64 : Outport  Port=2132
  RadarSensor:4.OBJ_S_Velocity : Outport  Port=2133
  RadarSensor:4.OBJ_S_Velocity_1 : Outport  Port=2134
  RadarSensor:4.OBJ_S_Velocity_2 : Outport  Port=2135
  RadarSensor:4.OBJ_S_Velocity_3 : Outport  Port=2136
  RadarSensor:4.OBJ_S_Velocity_4 : Outport  Port=2137
  RadarSensor:4.OBJ_S_Velocity_5 : Outport  Port=2138
  RadarSensor:4.OBJ_S_Velocity_6 : Outport  Port=2139
  RadarSensor:4.OBJ_S_Velocity_7 : Outport  Port=2140
  RadarSensor:4.OBJ_S_Velocity_8 : Outport  Port=2141
  RadarSensor:4.OBJ_S_Velocity_9 : Outport  Port=2142
  RadarSensor:4.OBJ_S_Velocity_10 : Outport  Port=2143
  RadarSensor:4.OBJ_S_Velocity_11 : Outport  Port=2144
  RadarSensor:4.OBJ_S_Velocity_12 : Outport  Port=2145
  RadarSensor:4.OBJ_S_Velocity_13 : Outport  Port=2146
  RadarSensor:4.OBJ_S_Velocity_14 : Outport  Port=2147
  RadarSensor:4.OBJ_S_Velocity_15 : Outport  Port=2148
  RadarSensor:4.OBJ_S_Velocity_16 : Outport  Port=2149
  RadarSensor:4.OBJ_S_Velocity_17 : Outport  Port=2150
  RadarSensor:4.OBJ_S_Velocity_18 : Outport  Port=2151
  RadarSensor:4.OBJ_S_Velocity_19 : Outport  Port=2152
  RadarSensor:4.OBJ_S_Velocity_20 : Outport  Port=2153
  RadarSensor:4.OBJ_S_Velocity_21 : Outport  Port=2154
  RadarSensor:4.OBJ_S_Velocity_22 : Outport  Port=2155
  RadarSensor:4.OBJ_S_Velocity_23 : Outport  Port=2156
  RadarSensor:4.OBJ_S_Velocity_24 : Outport  Port=2157
  RadarSensor:4.OBJ_S_Velocity_25 : Outport  Port=2158
  RadarSensor:4.OBJ_S_Velocity_26 : Outport  Port=2159
  RadarSensor:4.OBJ_S_Velocity_27 : Outport  Port=2160
  RadarSensor:4.OBJ_S_Velocity_28 : Outport  Port=2161
  RadarSensor:4.OBJ_S_Velocity_29 : Outport  Port=2162
  RadarSensor:4.OBJ_S_Velocity_30 : Outport  Port=2163
  RadarSensor:4.OBJ_S_Velocity_31 : Outport  Port=2164
  RadarSensor:4.OBJ_S_Velocity_32 : Outport  Port=2165
  RadarSensor:4.OBJ_S_Velocity_33 : Outport  Port=2166
  RadarSensor:4.OBJ_S_Velocity_34 : Outport  Port=2167
  RadarSensor:4.OBJ_S_Velocity_35 : Outport  Port=2168
  RadarSensor:4.OBJ_S_Velocity_36 : Outport  Port=2169
  RadarSensor:4.OBJ_S_Velocity_37 : Outport  Port=2170
  RadarSensor:4.OBJ_S_Velocity_38 : Outport  Port=2171
  RadarSensor:4.OBJ_S_Velocity_39 : Outport  Port=2172
  RadarSensor:4.OBJ_S_Velocity_40 : Outport  Port=2173
  RadarSensor:4.OBJ_S_Velocity_41 : Outport  Port=2174
  RadarSensor:4.OBJ_S_Velocity_42 : Outport  Port=2175
  RadarSensor:4.OBJ_S_Velocity_43 : Outport  Port=2176
  RadarSensor:4.OBJ_S_Velocity_44 : Outport  Port=2177
  RadarSensor:4.OBJ_S_Velocity_45 : Outport  Port=2178
  RadarSensor:4.OBJ_S_Velocity_46 : Outport  Port=2179
  RadarSensor:4.OBJ_S_Velocity_47 : Outport  Port=2180
  RadarSensor:4.OBJ_S_Velocity_48 : Outport  Port=2181
  RadarSensor:4.OBJ_S_Velocity_49 : Outport  Port=2182
  RadarSensor:4.OBJ_S_Velocity_50 : Outport  Port=2183
  RadarSensor:4.OBJ_S_Velocity_51 : Outport  Port=2184
  RadarSensor:4.OBJ_S_Velocity_52 : Outport  Port=2185
  RadarSensor:4.OBJ_S_Velocity_53 : Outport  Port=2186
  RadarSensor:4.OBJ_S_Velocity_54 : Outport  Port=2187
  RadarSensor:4.OBJ_S_Velocity_55 : Outport  Port=2188
  RadarSensor:4.OBJ_S_Velocity_56 : Outport  Port=2189
  RadarSensor:4.OBJ_S_Velocity_57 : Outport  Port=2190
  RadarSensor:4.OBJ_S_Velocity_58 : Outport  Port=2191
  RadarSensor:4.OBJ_S_Velocity_59 : Outport  Port=2192
  RadarSensor:4.OBJ_S_Velocity_60 : Outport  Port=2193
  RadarSensor:4.OBJ_S_Velocity_61 : Outport  Port=2194
  RadarSensor:4.OBJ_S_Velocity_62 : Outport  Port=2195
  RadarSensor:4.OBJ_S_Velocity_63 : Outport  Port=2196
  RadarSensor:4.OBJ_S_Velocity_64 : Outport  Port=2197
  RadarSensor:4.OBJ_S_Range : Outport  Port=2198
  RadarSensor:4.OBJ_S_Range_1 : Outport  Port=2199
  RadarSensor:4.OBJ_S_Range_2 : Outport  Port=2200
  RadarSensor:4.OBJ_S_Range_3 : Outport  Port=2201
  RadarSensor:4.OBJ_S_Range_4 : Outport  Port=2202
  RadarSensor:4.OBJ_S_Range_5 : Outport  Port=2203
  RadarSensor:4.OBJ_S_Range_6 : Outport  Port=2204
  RadarSensor:4.OBJ_S_Range_7 : Outport  Port=2205
  RadarSensor:4.OBJ_S_Range_8 : Outport  Port=2206
  RadarSensor:4.OBJ_S_Range_9 : Outport  Port=2207
  RadarSensor:4.OBJ_S_Range_10 : Outport  Port=2208
  RadarSensor:4.OBJ_S_Range_11 : Outport  Port=2209
  RadarSensor:4.OBJ_S_Range_12 : Outport  Port=2210
  RadarSensor:4.OBJ_S_Range_13 : Outport  Port=2211
  RadarSensor:4.OBJ_S_Range_14 : Outport  Port=2212
  RadarSensor:4.OBJ_S_Range_15 : Outport  Port=2213
  RadarSensor:4.OBJ_S_Range_16 : Outport  Port=2214
  RadarSensor:4.OBJ_S_Range_17 : Outport  Port=2215
  RadarSensor:4.OBJ_S_Range_18 : Outport  Port=2216
  RadarSensor:4.OBJ_S_Range_19 : Outport  Port=2217
  RadarSensor:4.OBJ_S_Range_20 : Outport  Port=2218
  RadarSensor:4.OBJ_S_Range_21 : Outport  Port=2219
  RadarSensor:4.OBJ_S_Range_22 : Outport  Port=2220
  RadarSensor:4.OBJ_S_Range_23 : Outport  Port=2221
  RadarSensor:4.OBJ_S_Range_24 : Outport  Port=2222
  RadarSensor:4.OBJ_S_Range_25 : Outport  Port=2223
  RadarSensor:4.OBJ_S_Range_26 : Outport  Port=2224
  RadarSensor:4.OBJ_S_Range_27 : Outport  Port=2225
  RadarSensor:4.OBJ_S_Range_28 : Outport  Port=2226
  RadarSensor:4.OBJ_S_Range_29 : Outport  Port=2227
  RadarSensor:4.OBJ_S_Range_30 : Outport  Port=2228
  RadarSensor:4.OBJ_S_Range_31 : Outport  Port=2229
  RadarSensor:4.OBJ_S_Range_32 : Outport  Port=2230
  RadarSensor:4.OBJ_S_Range_33 : Outport  Port=2231
  RadarSensor:4.OBJ_S_Range_34 : Outport  Port=2232
  RadarSensor:4.OBJ_S_Range_35 : Outport  Port=2233
  RadarSensor:4.OBJ_S_Range_36 : Outport  Port=2234
  RadarSensor:4.OBJ_S_Range_37 : Outport  Port=2235
  RadarSensor:4.OBJ_S_Range_38 : Outport  Port=2236
  RadarSensor:4.OBJ_S_Range_39 : Outport  Port=2237
  RadarSensor:4.OBJ_S_Range_40 : Outport  Port=2238
  RadarSensor:4.OBJ_S_Range_41 : Outport  Port=2239
  RadarSensor:4.OBJ_S_Range_42 : Outport  Port=2240
  RadarSensor:4.OBJ_S_Range_43 : Outport  Port=2241
  RadarSensor:4.OBJ_S_Range_44 : Outport  Port=2242
  RadarSensor:4.OBJ_S_Range_45 : Outport  Port=2243
  RadarSensor:4.OBJ_S_Range_46 : Outport  Port=2244
  RadarSensor:4.OBJ_S_Range_47 : Outport  Port=2245
  RadarSensor:4.OBJ_S_Range_48 : Outport  Port=2246
  RadarSensor:4.OBJ_S_Range_49 : Outport  Port=2247
  RadarSensor:4.OBJ_S_Range_50 : Outport  Port=2248
  RadarSensor:4.OBJ_S_Range_51 : Outport  Port=2249
  RadarSensor:4.OBJ_S_Range_52 : Outport  Port=2250
  RadarSensor:4.OBJ_S_Range_53 : Outport  Port=2251
  RadarSensor:4.OBJ_S_Range_54 : Outport  Port=2252
  RadarSensor:4.OBJ_S_Range_55 : Outport  Port=2253
  RadarSensor:4.OBJ_S_Range_56 : Outport  Port=2254
  RadarSensor:4.OBJ_S_Range_57 : Outport  Port=2255
  RadarSensor:4.OBJ_S_Range_58 : Outport  Port=2256
  RadarSensor:4.OBJ_S_Range_59 : Outport  Port=2257
  RadarSensor:4.OBJ_S_Range_60 : Outport  Port=2258
  RadarSensor:4.OBJ_S_Range_61 : Outport  Port=2259
  RadarSensor:4.OBJ_S_Range_62 : Outport  Port=2260
  RadarSensor:4.OBJ_S_Range_63 : Outport  Port=2261
  RadarSensor:4.OBJ_S_Range_64 : Outport  Port=2262
  RadarSensor:4.OBJ_RCS : Outport  Port=2263
  RadarSensor:4.OBJ_RCS_1 : Outport  Port=2264
  RadarSensor:4.OBJ_RCS_2 : Outport  Port=2265
  RadarSensor:4.OBJ_RCS_3 : Outport  Port=2266
  RadarSensor:4.OBJ_RCS_4 : Outport  Port=2267
  RadarSensor:4.OBJ_RCS_5 : Outport  Port=2268
  RadarSensor:4.OBJ_RCS_6 : Outport  Port=2269
  RadarSensor:4.OBJ_RCS_7 : Outport  Port=2270
  RadarSensor:4.OBJ_RCS_8 : Outport  Port=2271
  RadarSensor:4.OBJ_RCS_9 : Outport  Port=2272
  RadarSensor:4.OBJ_RCS_10 : Outport  Port=2273
  RadarSensor:4.OBJ_RCS_11 : Outport  Port=2274
  RadarSensor:4.OBJ_RCS_12 : Outport  Port=2275
  RadarSensor:4.OBJ_RCS_13 : Outport  Port=2276
  RadarSensor:4.OBJ_RCS_14 : Outport  Port=2277
  RadarSensor:4.OBJ_RCS_15 : Outport  Port=2278
  RadarSensor:4.OBJ_RCS_16 : Outport  Port=2279
  RadarSensor:4.OBJ_RCS_17 : Outport  Port=2280
  RadarSensor:4.OBJ_RCS_18 : Outport  Port=2281
  RadarSensor:4.OBJ_RCS_19 : Outport  Port=2282
  RadarSensor:4.OBJ_RCS_20 : Outport  Port=2283
  RadarSensor:4.OBJ_RCS_21 : Outport  Port=2284
  RadarSensor:4.OBJ_RCS_22 : Outport  Port=2285
  RadarSensor:4.OBJ_RCS_23 : Outport  Port=2286
  RadarSensor:4.OBJ_RCS_24 : Outport  Port=2287
  RadarSensor:4.OBJ_RCS_25 : Outport  Port=2288
  RadarSensor:4.OBJ_RCS_26 : Outport  Port=2289
  RadarSensor:4.OBJ_RCS_27 : Outport  Port=2290
  RadarSensor:4.OBJ_RCS_28 : Outport  Port=2291
  RadarSensor:4.OBJ_RCS_29 : Outport  Port=2292
  RadarSensor:4.OBJ_RCS_30 : Outport  Port=2293
  RadarSensor:4.OBJ_RCS_31 : Outport  Port=2294
  RadarSensor:4.OBJ_RCS_32 : Outport  Port=2295
  RadarSensor:4.OBJ_RCS_33 : Outport  Port=2296
  RadarSensor:4.OBJ_RCS_34 : Outport  Port=2297
  RadarSensor:4.OBJ_RCS_35 : Outport  Port=2298
  RadarSensor:4.OBJ_RCS_36 : Outport  Port=2299
  RadarSensor:4.OBJ_RCS_37 : Outport  Port=2300
  RadarSensor:4.OBJ_RCS_38 : Outport  Port=2301
  RadarSensor:4.OBJ_RCS_39 : Outport  Port=2302
  RadarSensor:4.OBJ_RCS_40 : Outport  Port=2303
  RadarSensor:4.OBJ_RCS_41 : Outport  Port=2304
  RadarSensor:4.OBJ_RCS_42 : Outport  Port=2305
  RadarSensor:4.OBJ_RCS_43 : Outport  Port=2306
  RadarSensor:4.OBJ_RCS_44 : Outport  Port=2307
  RadarSensor:4.OBJ_RCS_45 : Outport  Port=2308
  RadarSensor:4.OBJ_RCS_46 : Outport  Port=2309
  RadarSensor:4.OBJ_RCS_47 : Outport  Port=2310
  RadarSensor:4.OBJ_RCS_48 : Outport  Port=2311
  RadarSensor:4.OBJ_RCS_49 : Outport  Port=2312
  RadarSensor:4.OBJ_RCS_50 : Outport  Port=2313
  RadarSensor:4.OBJ_RCS_51 : Outport  Port=2314
  RadarSensor:4.OBJ_RCS_52 : Outport  Port=2315
  RadarSensor:4.OBJ_RCS_53 : Outport  Port=2316
  RadarSensor:4.OBJ_RCS_54 : Outport  Port=2317
  RadarSensor:4.OBJ_RCS_55 : Outport  Port=2318
  RadarSensor:4.OBJ_RCS_56 : Outport  Port=2319
  RadarSensor:4.OBJ_RCS_57 : Outport  Port=2320
  RadarSensor:4.OBJ_RCS_58 : Outport  Port=2321
  RadarSensor:4.OBJ_RCS_59 : Outport  Port=2322
  RadarSensor:4.OBJ_RCS_60 : Outport  Port=2323
  RadarSensor:4.OBJ_RCS_61 : Outport  Port=2324
  RadarSensor:4.OBJ_RCS_62 : Outport  Port=2325
  RadarSensor:4.OBJ_RCS_63 : Outport  Port=2326
  RadarSensor:4.OBJ_RCS_64 : Outport  Port=2327
  UltrasonicSensor:0.time : Outport  Port=2328
  UltrasonicSensor:0.width : Outport  Port=2329
  UltrasonicSensor:0.distance : Outport  Port=2330
  UltrasonicSensor:1.time : Outport  Port=2331
  UltrasonicSensor:1.width : Outport  Port=2332
  UltrasonicSensor:1.distance : Outport  Port=2333
  UltrasonicSensor:2.time : Outport  Port=2334
  UltrasonicSensor:2.width : Outport  Port=2335
  UltrasonicSensor:2.distance : Outport  Port=2336
  UltrasonicSensor:3.time : Outport  Port=2337
  UltrasonicSensor:3.width : Outport  Port=2338
  UltrasonicSensor:3.distance : Outport  Port=2339
  UltrasonicSensor:4.time : Outport  Port=2340
  UltrasonicSensor:4.width : Outport  Port=2341
  UltrasonicSensor:4.distance : Outport  Port=2342
  UltrasonicSensor:5.time : Outport  Port=2343
  UltrasonicSensor:5.width : Outport  Port=2344
  UltrasonicSensor:5.distance : Outport  Port=2345
  UltrasonicSensor:6.time : Outport  Port=2346
  UltrasonicSensor:6.width : Outport  Port=2347
  UltrasonicSensor:6.distance : Outport  Port=2348
  UltrasonicSensor:7.time : Outport  Port=2349
  UltrasonicSensor:7.width : Outport  Port=2350
  UltrasonicSensor:7.distance : Outport  Port=2351
  UltrasonicSensor:8.time : Outport  Port=2352
  UltrasonicSensor:8.width : Outport  Port=2353
  UltrasonicSensor:8.distance : Outport  Port=2354
  UltrasonicSensor:9.time : Outport  Port=2355
  UltrasonicSensor:9.width : Outport  Port=2356
  UltrasonicSensor:9.distance : Outport  Port=2357
  UltrasonicSensor:10.time : Outport  Port=2358
  UltrasonicSensor:10.width : Outport  Port=2359
  UltrasonicSensor:10.distance : Outport  Port=2360
  UltrasonicSensor:11.time : Outport  Port=2361
  UltrasonicSensor:11.width : Outport  Port=2362
  UltrasonicSensor:11.distance : Outport  Port=2363
  GNSS:0.Timestamp : Outport  Port=2364
  GNSS:0.Longitude : Outport  Port=2365
  GNSS:0.Latitude : Outport  Port=2366
  GNSS:0.Altitude : Outport  Port=2367
  GNSS:0.Heading : Outport  Port=2368
  GNSS:0.Velocity : Outport  Port=2369
  IMU:0.Timestamp : Outport  Port=2370
  IMU:0.ACC_X : Outport  Port=2371
  IMU:0.ACC_Y : Outport  Port=2372
  IMU:0.ACC_Z : Outport  Port=2373
  IMU:0.Gyro_X : Outport  Port=2374
  IMU:0.Gyro_Y : Outport  Port=2375
  IMU:0.Gyro_Z : Outport  Port=2376
  IMU:0.Yaw : Outport  Port=2377
  IMU:0.Pitch : Outport  Port=2378
  IMU:0.Roll : Outport  Port=2379
  wires:
  SensorsInput/1 -> Bus Selector:FreeSpacePerception:0/1, Bus Selector:GNSS:0/1, Bus Selector:LaneInfoPerception:0/1, Bus Selector:ObjectPerception:0/1, Bus Selector:ParkingLotsPerception:0/1, Bus Selector:TrafficLightPerception:0/1, Bus Selector:RadarSensor:0/1, Bus Selector:RadarSensor:1/1, Bus Selector:RadarSensor:2/1, Bus Selector:RadarSensor:3/1, Bus Selector:RadarSensor:4/1, Bus Selector:UltrasonicSensor:0/1, Bus Selector:UltrasonicSensor:1/1, Bus Selector:UltrasonicSensor:2/1, Bus Selector:UltrasonicSensor:3/1, Bus Selector:UltrasonicSensor:4/1, Bus Selector:UltrasonicSensor:5/1, Bus Selector:UltrasonicSensor:6/1, Bus Selector:UltrasonicSensor:7/1, Bus Selector:UltrasonicSensor:8/1, Bus Selector:UltrasonicSensor:9/1, Bus Selector:UltrasonicSensor:10/1, Bus Selector:UltrasonicSensor:11/1, Bus Selector:IMU:0/1
  Bus Selector:FreeSpacePerception:0/1 -> FreeSpacePerception:0.time/1  "<time>"
  Bus Selector:FreeSpacePerception:0/2 -> FreeSpacePerception:0.width/1  "<width>"
  Bus Selector:FreeSpacePerception:0/3 -> FreeSpacePerception:0.x/1  "<x>"
  Bus Selector:FreeSpacePerception:0/4 -> FreeSpacePerception:0.y/1  "<y>"
  Bus Selector:LaneInfoPerception:0/1 -> LaneInfoPerception:0.Timestamp/1  "<Timestamp>"
  Bus Selector:LaneInfoPerception:0/2 -> LaneInfoPerception:0.width/1  "<width>"
  Bus Selector:LaneInfoPerception:0/3 -> LaneInfoPerception:0.Lane_ID/1  "<Lane_ID>"
  Bus Selector:LaneInfoPerception:0/4 -> LaneInfoPerception:0.Lane_Distance/1  "<Lane_Distance>"
  Bus Selector:LaneInfoPerception:0/5 -> LaneInfoPerception:0.Lane_Car_Distance_Left/1  "<Lane_Car_Distance_Left>"
  Bus Selector:LaneInfoPerception:0/6 -> LaneInfoPerception:0.Lane_Car_Distance_Right/1  "<Lane_Car_Distance_Right>"
  Bus Selector:LaneInfoPerception:0/7 -> LaneInfoPerception:0.Lane_Curvature/1  "<Lane_Curvature>"
  Bus Selector:LaneInfoPerception:0/8 -> LaneInfoPerception:0.Lane_Coefficient_C0/1  "<Lane_Coefficient_C0>"
  Bus Selector:LaneInfoPerception:0/9 -> LaneInfoPerception:0.Lane_Coefficient_C1/1  "<Lane_Coefficient_C1>"
  Bus Selector:LaneInfoPerception:0/10 -> LaneInfoPerception:0.Lane_Coefficient_C2/1  "<Lane_Coefficient_C2>"
  Bus Selector:LaneInfoPerception:0/11 -> LaneInfoPerception:0.Lane_Coefficient_C3/1  "<Lane_Coefficient_C3>"
  Bus Selector:LaneInfoPerception:0/12 -> LaneInfoPerception:0.Lane_Class/1  "<Lane_Class>"
  Bus Selector:ObjectPerception:0/1 -> ObjectPerception:0.Timestamp/1  "<Timestamp>"
  Bus Selector:ObjectPerception:0/2 -> ObjectPerception:0.width/1  "<width>"
  Bus Selector:ObjectPerception:0/3 -> ObjectPerception:0.OBJ_ID/1  "<OBJ_ID>"
  Bus Selector:ObjectPerception:0/4 -> ObjectPerception:0.OBJ_Class/1  "<OBJ_Class>"
  Bus Selector:ObjectPerception:0/5 -> ObjectPerception:0.OBJ_X/1  "<OBJ_X>"
  Bus Selector:ObjectPerception:0/6 -> ObjectPerception:0.OBJ_Y/1  "<OBJ_Y>"
  Bus Selector:ObjectPerception:0/7 -> ObjectPerception:0.OBJ_Z/1  "<OBJ_Z>"
  Bus Selector:ObjectPerception:0/8 -> ObjectPerception:0.OBJ_Velocity/1  "<OBJ_Velocity>"
  Bus Selector:ObjectPerception:0/9 -> ObjectPerception:0.OBJ_Length/1  "<OBJ_Length>"
  Bus Selector:ObjectPerception:0/10 -> ObjectPerception:0.OBJ_Width/1  "<OBJ_Width>"
  Bus Selector:ObjectPerception:0/11 -> ObjectPerception:0.OBJ_Height/1  "<OBJ_Height>"
  Bus Selector:ParkingLotsPerception:0/1 -> ParkingLotsPerception:0.time/1  "<time>"
  Bus Selector:ParkingLotsPerception:0/2 -> ParkingLotsPerception:0.width/1  "<width>"
  Bus Selector:ParkingLotsPerception:0/3 -> ParkingLotsPerception:0.x1/1  "<x1>"
  Bus Selector:ParkingLotsPerception:0/4 -> ParkingLotsPerception:0.y1/1  "<y1>"
  Bus Selector:ParkingLotsPerception:0/5 -> ParkingLotsPerception:0.x2/1  "<x2>"
  Bus Selector:ParkingLotsPerception:0/6 -> ParkingLotsPerception:0.y2/1  "<y2>"
  Bus Selector:ParkingLotsPerception:0/7 -> ParkingLotsPerception:0.x3/1  "<x3>"
  Bus Selector:ParkingLotsPerception:0/8 -> ParkingLotsPerception:0.y3/1  "<y3>"
  Bus Selector:ParkingLotsPerception:0/9 -> ParkingLotsPerception:0.x4/1  "<x4>"
  Bus Selector:ParkingLotsPerception:0/10 -> ParkingLotsPerception:0.y4/1  "<y4>"
  Bus Selector:TrafficLightPerception:0/1 -> TrafficLightPerception:0.Timestamp/1  "<Timestamp>"
  Bus Selector:TrafficLightPerception:0/2 -> TrafficLightPerception:0.width/1  "<width>"
  Bus Selector:TrafficLightPerception:0/3 -> TrafficLightPerception:0.TrafficLight_Direction/1  "<TrafficLight_Direction>"
  Bus Selector:TrafficLightPerception:0/4 -> TrafficLightPerception:0.TrafficLight_State/1  "<TrafficLight_State>"
  Bus Selector:TrafficLightPerception:0/5 -> TrafficLightPerception:0.TrafficLight_Timer/1  "<TrafficLight_Timer>"
  Bus Selector:RadarSensor:0_OBJ_ID_BS/1 -> RadarSensor:0.OBJ_ID_1/1  "<OBJ_ID_1>"
  Bus Selector:RadarSensor:0_OBJ_ID_BS/2 -> RadarSensor:0.OBJ_ID_2/1  "<OBJ_ID_2>"
  Bus Selector:RadarSensor:0_OBJ_ID_BS/3 -> RadarSensor:0.OBJ_ID_3/1  "<OBJ_ID_3>"
  Bus Selector:RadarSensor:0_OBJ_ID_BS/4 -> RadarSensor:0.OBJ_ID_4/1  "<OBJ_ID_4>"
  Bus Selector:RadarSensor:0_OBJ_ID_BS/5 -> RadarSensor:0.OBJ_ID_5/1  "<OBJ_ID_5>"
  Bus Selector:RadarSensor:0_OBJ_ID_BS/6 -> RadarSensor:0.OBJ_ID_6/1  "<OBJ_ID_6>"
  Bus Selector:RadarSensor:0_OBJ_ID_BS/7 -> RadarSensor:0.OBJ_ID_7/1  "<OBJ_ID_7>"
  Bus Selector:RadarSensor:0_OBJ_ID_BS/8 -> RadarSensor:0.OBJ_ID_8/1  "<OBJ_ID_8>"
  Bus Selector:RadarSensor:0_OBJ_ID_BS/9 -> RadarSensor:0.OBJ_ID_9/1  "<OBJ_ID_9>"
  Bus Selector:RadarSensor:0_OBJ_ID_BS/10 -> RadarSensor:0.OBJ_ID_10/1  "<OBJ_ID_10>"
  Bus Selector:RadarSensor:0_OBJ_ID_BS/11 -> RadarSensor:0.OBJ_ID_11/1  "<OBJ_ID_11>"
  Bus Selector:RadarSensor:0_OBJ_ID_BS/12 -> RadarSensor:0.OBJ_ID_12/1  "<OBJ_ID_12>"
  Bus Selector:RadarSensor:0_OBJ_ID_BS/13 -> RadarSensor:0.OBJ_ID_13/1  "<OBJ_ID_13>"
  Bus Selector:RadarSensor:0_OBJ_ID_BS/14 -> RadarSensor:0.OBJ_ID_14/1  "<OBJ_ID_14>"
  Bus Selector:RadarSensor:0_OBJ_ID_BS/15 -> RadarSensor:0.OBJ_ID_15/1  "<OBJ_ID_15>"
  Bus Selector:RadarSensor:0_OBJ_ID_BS/16 -> RadarSensor:0.OBJ_ID_16/1  "<OBJ_ID_16>"
  Bus Selector:RadarSensor:0_OBJ_ID_BS/17 -> RadarSensor:0.OBJ_ID_17/1  "<OBJ_ID_17>"
  Bus Selector:RadarSensor:0_OBJ_ID_BS/18 -> RadarSensor:0.OBJ_ID_18/1  "<OBJ_ID_18>"
  Bus Selector:RadarSensor:0_OBJ_ID_BS/19 -> RadarSensor:0.OBJ_ID_19/1  "<OBJ_ID_19>"
  Bus Selector:RadarSensor:0_OBJ_ID_BS/20 -> RadarSensor:0.OBJ_ID_20/1  "<OBJ_ID_20>"
  Bus Selector:RadarSensor:0_OBJ_ID_BS/21 -> RadarSensor:0.OBJ_ID_21/1  "<OBJ_ID_21>"
  Bus Selector:RadarSensor:0_OBJ_ID_BS/22 -> RadarSensor:0.OBJ_ID_22/1  "<OBJ_ID_22>"
  Bus Selector:RadarSensor:0_OBJ_ID_BS/23 -> RadarSensor:0.OBJ_ID_23/1  "<OBJ_ID_23>"
  Bus Selector:RadarSensor:0_OBJ_ID_BS/24 -> RadarSensor:0.OBJ_ID_24/1  "<OBJ_ID_24>"
  Bus Selector:RadarSensor:0_OBJ_ID_BS/25 -> RadarSensor:0.OBJ_ID_25/1  "<OBJ_ID_25>"
  Bus Selector:RadarSensor:0_OBJ_ID_BS/26 -> RadarSensor:0.OBJ_ID_26/1  "<OBJ_ID_26>"
  Bus Selector:RadarSensor:0_OBJ_ID_BS/27 -> RadarSensor:0.OBJ_ID_27/1  "<OBJ_ID_27>"
  Bus Selector:RadarSensor:0_OBJ_ID_BS/28 -> RadarSensor:0.OBJ_ID_28/1  "<OBJ_ID_28>"
  Bus Selector:RadarSensor:0_OBJ_ID_BS/29 -> RadarSensor:0.OBJ_ID_29/1  "<OBJ_ID_29>"
  Bus Selector:RadarSensor:0_OBJ_ID_BS/30 -> RadarSensor:0.OBJ_ID_30/1  "<OBJ_ID_30>"
  Bus Selector:RadarSensor:0_OBJ_ID_BS/31 -> RadarSensor:0.OBJ_ID_31/1  "<OBJ_ID_31>"
  Bus Selector:RadarSensor:0_OBJ_ID_BS/32 -> RadarSensor:0.OBJ_ID_32/1  "<OBJ_ID_32>"
  Bus Selector:RadarSensor:0_OBJ_ID_BS/33 -> RadarSensor:0.OBJ_ID_33/1  "<OBJ_ID_33>"
  Bus Selector:RadarSensor:0_OBJ_ID_BS/34 -> RadarSensor:0.OBJ_ID_34/1  "<OBJ_ID_34>"
  Bus Selector:RadarSensor:0_OBJ_ID_BS/35 -> RadarSensor:0.OBJ_ID_35/1  "<OBJ_ID_35>"
  Bus Selector:RadarSensor:0_OBJ_ID_BS/36 -> RadarSensor:0.OBJ_ID_36/1  "<OBJ_ID_36>"
  Bus Selector:RadarSensor:0_OBJ_ID_BS/37 -> RadarSensor:0.OBJ_ID_37/1  "<OBJ_ID_37>"
  Bus Selector:RadarSensor:0_OBJ_ID_BS/38 -> RadarSensor:0.OBJ_ID_38/1  "<OBJ_ID_38>"
  Bus Selector:RadarSensor:0_OBJ_ID_BS/39 -> RadarSensor:0.OBJ_ID_39/1  "<OBJ_ID_39>"
  Bus Selector:RadarSensor:0_OBJ_ID_BS/40 -> RadarSensor:0.OBJ_ID_40/1  "<OBJ_ID_40>"
  Bus Selector:RadarSensor:0_OBJ_ID_BS/41 -> RadarSensor:0.OBJ_ID_41/1  "<OBJ_ID_41>"
  Bus Selector:RadarSensor:0_OBJ_ID_BS/42 -> RadarSensor:0.OBJ_ID_42/1  "<OBJ_ID_42>"
  Bus Selector:RadarSensor:0_OBJ_ID_BS/43 -> RadarSensor:0.OBJ_ID_43/1  "<OBJ_ID_43>"
  Bus Selector:RadarSensor:0_OBJ_ID_BS/44 -> RadarSensor:0.OBJ_ID_44/1  "<OBJ_ID_44>"
  Bus Selector:RadarSensor:0_OBJ_ID_BS/45 -> RadarSensor:0.OBJ_ID_45/1  "<OBJ_ID_45>"
  Bus Selector:RadarSensor:0_OBJ_ID_BS/46 -> RadarSensor:0.OBJ_ID_46/1  "<OBJ_ID_46>"
  Bus Selector:RadarSensor:0_OBJ_ID_BS/47 -> RadarSensor:0.OBJ_ID_47/1  "<OBJ_ID_47>"
  Bus Selector:RadarSensor:0_OBJ_ID_BS/48 -> RadarSensor:0.OBJ_ID_48/1  "<OBJ_ID_48>"
  Bus Selector:RadarSensor:0_OBJ_ID_BS/49 -> RadarSensor:0.OBJ_ID_49/1  "<OBJ_ID_49>"
  Bus Selector:RadarSensor:0_OBJ_ID_BS/50 -> RadarSensor:0.OBJ_ID_50/1  "<OBJ_ID_50>"
  Bus Selector:RadarSensor:0_OBJ_ID_BS/51 -> RadarSensor:0.OBJ_ID_51/1  "<OBJ_ID_51>"
  Bus Selector:RadarSensor:0_OBJ_ID_BS/52 -> RadarSensor:0.OBJ_ID_52/1  "<OBJ_ID_52>"
  Bus Selector:RadarSensor:0_OBJ_ID_BS/53 -> RadarSensor:0.OBJ_ID_53/1  "<OBJ_ID_53>"
  Bus Selector:RadarSensor:0_OBJ_ID_BS/54 -> RadarSensor:0.OBJ_ID_54/1  "<OBJ_ID_54>"
  Bus Selector:RadarSensor:0_OBJ_ID_BS/55 -> RadarSensor:0.OBJ_ID_55/1  "<OBJ_ID_55>"
  Bus Selector:RadarSensor:0_OBJ_ID_BS/56 -> RadarSensor:0.OBJ_ID_56/1  "<OBJ_ID_56>"
  Bus Selector:RadarSensor:0_OBJ_ID_BS/57 -> RadarSensor:0.OBJ_ID_57/1  "<OBJ_ID_57>"
  Bus Selector:RadarSensor:0_OBJ_ID_BS/58 -> RadarSensor:0.OBJ_ID_58/1  "<OBJ_ID_58>"
  Bus Selector:RadarSensor:0_OBJ_ID_BS/59 -> RadarSensor:0.OBJ_ID_59/1  "<OBJ_ID_59>"
  Bus Selector:RadarSensor:0_OBJ_ID_BS/60 -> RadarSensor:0.OBJ_ID_60/1  "<OBJ_ID_60>"
  Bus Selector:RadarSensor:0_OBJ_ID_BS/61 -> RadarSensor:0.OBJ_ID_61/1  "<OBJ_ID_61>"
  Bus Selector:RadarSensor:0_OBJ_ID_BS/62 -> RadarSensor:0.OBJ_ID_62/1  "<OBJ_ID_62>"
  Bus Selector:RadarSensor:0_OBJ_ID_BS/63 -> RadarSensor:0.OBJ_ID_63/1  "<OBJ_ID_63>"
  Bus Selector:RadarSensor:0_OBJ_ID_BS/64 -> RadarSensor:0.OBJ_ID_64/1  "<OBJ_ID_64>"
  Bus Selector:RadarSensor:0_OBJ_Class_BS/1 -> RadarSensor:0.OBJ_Class_1/1  "<OBJ_Class_1>"
  Bus Selector:RadarSensor:0_OBJ_Class_BS/2 -> RadarSensor:0.OBJ_Class_2/1  "<OBJ_Class_2>"
  Bus Selector:RadarSensor:0_OBJ_Class_BS/3 -> RadarSensor:0.OBJ_Class_3/1  "<OBJ_Class_3>"
  Bus Selector:RadarSensor:0_OBJ_Class_BS/4 -> RadarSensor:0.OBJ_Class_4/1  "<OBJ_Class_4>"
  Bus Selector:RadarSensor:0_OBJ_Class_BS/5 -> RadarSensor:0.OBJ_Class_5/1  "<OBJ_Class_5>"
  Bus Selector:RadarSensor:0_OBJ_Class_BS/6 -> RadarSensor:0.OBJ_Class_6/1  "<OBJ_Class_6>"
  Bus Selector:RadarSensor:0_OBJ_Class_BS/7 -> RadarSensor:0.OBJ_Class_7/1  "<OBJ_Class_7>"
  Bus Selector:RadarSensor:0_OBJ_Class_BS/8 -> RadarSensor:0.OBJ_Class_8/1  "<OBJ_Class_8>"
  Bus Selector:RadarSensor:0_OBJ_Class_BS/9 -> RadarSensor:0.OBJ_Class_9/1  "<OBJ_Class_9>"
  Bus Selector:RadarSensor:0_OBJ_Class_BS/10 -> RadarSensor:0.OBJ_Class_10/1  "<OBJ_Class_10>"
  Bus Selector:RadarSensor:0_OBJ_Class_BS/11 -> RadarSensor:0.OBJ_Class_11/1  "<OBJ_Class_11>"
  Bus Selector:RadarSensor:0_OBJ_Class_BS/12 -> RadarSensor:0.OBJ_Class_12/1  "<OBJ_Class_12>"
  Bus Selector:RadarSensor:0_OBJ_Class_BS/13 -> RadarSensor:0.OBJ_Class_13/1  "<OBJ_Class_13>"
  Bus Selector:RadarSensor:0_OBJ_Class_BS/14 -> RadarSensor:0.OBJ_Class_14/1  "<OBJ_Class_14>"
  Bus Selector:RadarSensor:0_OBJ_Class_BS/15 -> RadarSensor:0.OBJ_Class_15/1  "<OBJ_Class_15>"
  Bus Selector:RadarSensor:0_OBJ_Class_BS/16 -> RadarSensor:0.OBJ_Class_16/1  "<OBJ_Class_16>"
  Bus Selector:RadarSensor:0_OBJ_Class_BS/17 -> RadarSensor:0.OBJ_Class_17/1  "<OBJ_Class_17>"
  Bus Selector:RadarSensor:0_OBJ_Class_BS/18 -> RadarSensor:0.OBJ_Class_18/1  "<OBJ_Class_18>"
  Bus Selector:RadarSensor:0_OBJ_Class_BS/19 -> RadarSensor:0.OBJ_Class_19/1  "<OBJ_Class_19>"
  Bus Selector:RadarSensor:0_OBJ_Class_BS/20 -> RadarSensor:0.OBJ_Class_20/1  "<OBJ_Class_20>"
  Bus Selector:RadarSensor:0_OBJ_Class_BS/21 -> RadarSensor:0.OBJ_Class_21/1  "<OBJ_Class_21>"
  Bus Selector:RadarSensor:0_OBJ_Class_BS/22 -> RadarSensor:0.OBJ_Class_22/1  "<OBJ_Class_22>"
  Bus Selector:RadarSensor:0_OBJ_Class_BS/23 -> RadarSensor:0.OBJ_Class_23/1  "<OBJ_Class_23>"
  Bus Selector:RadarSensor:0_OBJ_Class_BS/24 -> RadarSensor:0.OBJ_Class_24/1  "<OBJ_Class_24>"
  Bus Selector:RadarSensor:0_OBJ_Class_BS/25 -> RadarSensor:0.OBJ_Class_25/1  "<OBJ_Class_25>"
  Bus Selector:RadarSensor:0_OBJ_Class_BS/26 -> RadarSensor:0.OBJ_Class_26/1  "<OBJ_Class_26>"
  Bus Selector:RadarSensor:0_OBJ_Class_BS/27 -> RadarSensor:0.OBJ_Class_27/1  "<OBJ_Class_27>"
  Bus Selector:RadarSensor:0_OBJ_Class_BS/28 -> RadarSensor:0.OBJ_Class_28/1  "<OBJ_Class_28>"
  Bus Selector:RadarSensor:0_OBJ_Class_BS/29 -> RadarSensor:0.OBJ_Class_29/1  "<OBJ_Class_29>"
  Bus Selector:RadarSensor:0_OBJ_Class_BS/30 -> RadarSensor:0.OBJ_Class_30/1  "<OBJ_Class_30>"
  Bus Selector:RadarSensor:0_OBJ_Class_BS/31 -> RadarSensor:0.OBJ_Class_31/1  "<OBJ_Class_31>"
  Bus Selector:RadarSensor:0_OBJ_Class_BS/32 -> RadarSensor:0.OBJ_Class_32/1  "<OBJ_Class_32>"
  Bus Selector:RadarSensor:0_OBJ_Class_BS/33 -> RadarSensor:0.OBJ_Class_33/1  "<OBJ_Class_33>"
  Bus Selector:RadarSensor:0_OBJ_Class_BS/34 -> RadarSensor:0.OBJ_Class_34/1  "<OBJ_Class_34>"
  Bus Selector:RadarSensor:0_OBJ_Class_BS/35 -> RadarSensor:0.OBJ_Class_35/1  "<OBJ_Class_35>"
  Bus Selector:RadarSensor:0_OBJ_Class_BS/36 -> RadarSensor:0.OBJ_Class_36/1  "<OBJ_Class_36>"
  Bus Selector:RadarSensor:0_OBJ_Class_BS/37 -> RadarSensor:0.OBJ_Class_37/1  "<OBJ_Class_37>"
  Bus Selector:RadarSensor:0_OBJ_Class_BS/38 -> RadarSensor:0.OBJ_Class_38/1  "<OBJ_Class_38>"
  Bus Selector:RadarSensor:0_OBJ_Class_BS/39 -> RadarSensor:0.OBJ_Class_39/1  "<OBJ_Class_39>"
  Bus Selector:RadarSensor:0_OBJ_Class_BS/40 -> RadarSensor:0.OBJ_Class_40/1  "<OBJ_Class_40>"
  Bus Selector:RadarSensor:0_OBJ_Class_BS/41 -> RadarSensor:0.OBJ_Class_41/1  "<OBJ_Class_41>"
  Bus Selector:RadarSensor:0_OBJ_Class_BS/42 -> RadarSensor:0.OBJ_Class_42/1  "<OBJ_Class_42>"
  Bus Selector:RadarSensor:0_OBJ_Class_BS/43 -> RadarSensor:0.OBJ_Class_43/1  "<OBJ_Class_43>"
  Bus Selector:RadarSensor:0_OBJ_Class_BS/44 -> RadarSensor:0.OBJ_Class_44/1  "<OBJ_Class_44>"
  Bus Selector:RadarSensor:0_OBJ_Class_BS/45 -> RadarSensor:0.OBJ_Class_45/1  "<OBJ_Class_45>"
  Bus Selector:RadarSensor:0_OBJ_Class_BS/46 -> RadarSensor:0.OBJ_Class_46/1  "<OBJ_Class_46>"
  Bus Selector:RadarSensor:0_OBJ_Class_BS/47 -> RadarSensor:0.OBJ_Class_47/1  "<OBJ_Class_47>"
  Bus Selector:RadarSensor:0_OBJ_Class_BS/48 -> RadarSensor:0.OBJ_Class_48/1  "<OBJ_Class_48>"
  Bus Selector:RadarSensor:0_OBJ_Class_BS/49 -> RadarSensor:0.OBJ_Class_49/1  "<OBJ_Class_49>"
  Bus Selector:RadarSensor:0_OBJ_Class_BS/50 -> RadarSensor:0.OBJ_Class_50/1  "<OBJ_Class_50>"
  Bus Selector:RadarSensor:0_OBJ_Class_BS/51 -> RadarSensor:0.OBJ_Class_51/1  "<OBJ_Class_51>"
  Bus Selector:RadarSensor:0_OBJ_Class_BS/52 -> RadarSensor:0.OBJ_Class_52/1  "<OBJ_Class_52>"
  Bus Selector:RadarSensor:0_OBJ_Class_BS/53 -> RadarSensor:0.OBJ_Class_53/1  "<OBJ_Class_53>"
  Bus Selector:RadarSensor:0_OBJ_Class_BS/54 -> RadarSensor:0.OBJ_Class_54/1  "<OBJ_Class_54>"
  Bus Selector:RadarSensor:0_OBJ_Class_BS/55 -> RadarSensor:0.OBJ_Class_55/1  "<OBJ_Class_55>"
  Bus Selector:RadarSensor:0_OBJ_Class_BS/56 -> RadarSensor:0.OBJ_Class_56/1  "<OBJ_Class_56>"
  Bus Selector:RadarSensor:0_OBJ_Class_BS/57 -> RadarSensor:0.OBJ_Class_57/1  "<OBJ_Class_57>"
  Bus Selector:RadarSensor:0_OBJ_Class_BS/58 -> RadarSensor:0.OBJ_Class_58/1  "<OBJ_Class_58>"
  Bus Selector:RadarSensor:0_OBJ_Class_BS/59 -> RadarSensor:0.OBJ_Class_59/1  "<OBJ_Class_59>"
  Bus Selector:RadarSensor:0_OBJ_Class_BS/60 -> RadarSensor:0.OBJ_Class_60/1  "<OBJ_Class_60>"
  Bus Selector:RadarSensor:0_OBJ_Class_BS/61 -> RadarSensor:0.OBJ_Class_61/1  "<OBJ_Class_61>"
  Bus Selector:RadarSensor:0_OBJ_Class_BS/62 -> RadarSensor:0.OBJ_Class_62/1  "<OBJ_Class_62>"
  Bus Selector:RadarSensor:0_OBJ_Class_BS/63 -> RadarSensor:0.OBJ_Class_63/1  "<OBJ_Class_63>"
  Bus Selector:RadarSensor:0_OBJ_Class_BS/64 -> RadarSensor:0.OBJ_Class_64/1  "<OBJ_Class_64>"
  Bus Selector:RadarSensor:0_OBJ_S_Azimuth_BS/1 -> RadarSensor:0.OBJ_S_Azimuth_1/1  "<OBJ_S_Azimuth_1>"
  Bus Selector:RadarSensor:0_OBJ_S_Azimuth_BS/2 -> RadarSensor:0.OBJ_S_Azimuth_2/1  "<OBJ_S_Azimuth_2>"
  Bus Selector:RadarSensor:0_OBJ_S_Azimuth_BS/3 -> RadarSensor:0.OBJ_S_Azimuth_3/1  "<OBJ_S_Azimuth_3>"
  Bus Selector:RadarSensor:0_OBJ_S_Azimuth_BS/4 -> RadarSensor:0.OBJ_S_Azimuth_4/1  "<OBJ_S_Azimuth_4>"
  Bus Selector:RadarSensor:0_OBJ_S_Azimuth_BS/5 -> RadarSensor:0.OBJ_S_Azimuth_5/1  "<OBJ_S_Azimuth_5>"
  Bus Selector:RadarSensor:0_OBJ_S_Azimuth_BS/6 -> RadarSensor:0.OBJ_S_Azimuth_6/1  "<OBJ_S_Azimuth_6>"
  Bus Selector:RadarSensor:0_OBJ_S_Azimuth_BS/7 -> RadarSensor:0.OBJ_S_Azimuth_7/1  "<OBJ_S_Azimuth_7>"
  Bus Selector:RadarSensor:0_OBJ_S_Azimuth_BS/8 -> RadarSensor:0.OBJ_S_Azimuth_8/1  "<OBJ_S_Azimuth_8>"
  Bus Selector:RadarSensor:0_OBJ_S_Azimuth_BS/9 -> RadarSensor:0.OBJ_S_Azimuth_9/1  "<OBJ_S_Azimuth_9>"
  Bus Selector:RadarSensor:0_OBJ_S_Azimuth_BS/10 -> RadarSensor:0.OBJ_S_Azimuth_10/1  "<OBJ_S_Azimuth_10>"
  Bus Selector:RadarSensor:0_OBJ_S_Azimuth_BS/11 -> RadarSensor:0.OBJ_S_Azimuth_11/1  "<OBJ_S_Azimuth_11>"
  Bus Selector:RadarSensor:0_OBJ_S_Azimuth_BS/12 -> RadarSensor:0.OBJ_S_Azimuth_12/1  "<OBJ_S_Azimuth_12>"
  Bus Selector:RadarSensor:0_OBJ_S_Azimuth_BS/13 -> RadarSensor:0.OBJ_S_Azimuth_13/1  "<OBJ_S_Azimuth_13>"
  Bus Selector:RadarSensor:0_OBJ_S_Azimuth_BS/14 -> RadarSensor:0.OBJ_S_Azimuth_14/1  "<OBJ_S_Azimuth_14>"
  Bus Selector:RadarSensor:0_OBJ_S_Azimuth_BS/15 -> RadarSensor:0.OBJ_S_Azimuth_15/1  "<OBJ_S_Azimuth_15>"
  Bus Selector:RadarSensor:0_OBJ_S_Azimuth_BS/16 -> RadarSensor:0.OBJ_S_Azimuth_16/1  "<OBJ_S_Azimuth_16>"
  Bus Selector:RadarSensor:0_OBJ_S_Azimuth_BS/17 -> RadarSensor:0.OBJ_S_Azimuth_17/1  "<OBJ_S_Azimuth_17>"
  Bus Selector:RadarSensor:0_OBJ_S_Azimuth_BS/18 -> RadarSensor:0.OBJ_S_Azimuth_18/1  "<OBJ_S_Azimuth_18>"
  Bus Selector:RadarSensor:0_OBJ_S_Azimuth_BS/19 -> RadarSensor:0.OBJ_S_Azimuth_19/1  "<OBJ_S_Azimuth_19>"
  Bus Selector:RadarSensor:0_OBJ_S_Azimuth_BS/20 -> RadarSensor:0.OBJ_S_Azimuth_20/1  "<OBJ_S_Azimuth_20>"
  Bus Selector:RadarSensor:0_OBJ_S_Azimuth_BS/21 -> RadarSensor:0.OBJ_S_Azimuth_21/1  "<OBJ_S_Azimuth_21>"
  Bus Selector:RadarSensor:0_OBJ_S_Azimuth_BS/22 -> RadarSensor:0.OBJ_S_Azimuth_22/1  "<OBJ_S_Azimuth_22>"
  Bus Selector:RadarSensor:0_OBJ_S_Azimuth_BS/23 -> RadarSensor:0.OBJ_S_Azimuth_23/1  "<OBJ_S_Azimuth_23>"
  Bus Selector:RadarSensor:0_OBJ_S_Azimuth_BS/24 -> RadarSensor:0.OBJ_S_Azimuth_24/1  "<OBJ_S_Azimuth_24>"
  Bus Selector:RadarSensor:0_OBJ_S_Azimuth_BS/25 -> RadarSensor:0.OBJ_S_Azimuth_25/1  "<OBJ_S_Azimuth_25>"
  Bus Selector:RadarSensor:0_OBJ_S_Azimuth_BS/26 -> RadarSensor:0.OBJ_S_Azimuth_26/1  "<OBJ_S_Azimuth_26>"
  Bus Selector:RadarSensor:0_OBJ_S_Azimuth_BS/27 -> RadarSensor:0.OBJ_S_Azimuth_27/1  "<OBJ_S_Azimuth_27>"
  Bus Selector:RadarSensor:0_OBJ_S_Azimuth_BS/28 -> RadarSensor:0.OBJ_S_Azimuth_28/1  "<OBJ_S_Azimuth_28>"
  Bus Selector:RadarSensor:0_OBJ_S_Azimuth_BS/29 -> RadarSensor:0.OBJ_S_Azimuth_29/1  "<OBJ_S_Azimuth_29>"
  Bus Selector:RadarSensor:0_OBJ_S_Azimuth_BS/30 -> RadarSensor:0.OBJ_S_Azimuth_30/1  "<OBJ_S_Azimuth_30>"
  Bus Selector:RadarSensor:0_OBJ_S_Azimuth_BS/31 -> RadarSensor:0.OBJ_S_Azimuth_31/1  "<OBJ_S_Azimuth_31>"
  Bus Selector:RadarSensor:0_OBJ_S_Azimuth_BS/32 -> RadarSensor:0.OBJ_S_Azimuth_32/1  "<OBJ_S_Azimuth_32>"
  Bus Selector:RadarSensor:0_OBJ_S_Azimuth_BS/33 -> RadarSensor:0.OBJ_S_Azimuth_33/1  "<OBJ_S_Azimuth_33>"
  Bus Selector:RadarSensor:0_OBJ_S_Azimuth_BS/34 -> RadarSensor:0.OBJ_S_Azimuth_34/1  "<OBJ_S_Azimuth_34>"
  Bus Selector:RadarSensor:0_OBJ_S_Azimuth_BS/35 -> RadarSensor:0.OBJ_S_Azimuth_35/1  "<OBJ_S_Azimuth_35>"
  Bus Selector:RadarSensor:0_OBJ_S_Azimuth_BS/36 -> RadarSensor:0.OBJ_S_Azimuth_36/1  "<OBJ_S_Azimuth_36>"
  Bus Selector:RadarSensor:0_OBJ_S_Azimuth_BS/37 -> RadarSensor:0.OBJ_S_Azimuth_37/1  "<OBJ_S_Azimuth_37>"
  Bus Selector:RadarSensor:0_OBJ_S_Azimuth_BS/38 -> RadarSensor:0.OBJ_S_Azimuth_38/1  "<OBJ_S_Azimuth_38>"
  Bus Selector:RadarSensor:0_OBJ_S_Azimuth_BS/39 -> RadarSensor:0.OBJ_S_Azimuth_39/1  "<OBJ_S_Azimuth_39>"
  Bus Selector:RadarSensor:0_OBJ_S_Azimuth_BS/40 -> RadarSensor:0.OBJ_S_Azimuth_40/1  "<OBJ_S_Azimuth_40>"
  Bus Selector:RadarSensor:0_OBJ_S_Azimuth_BS/41 -> RadarSensor:0.OBJ_S_Azimuth_41/1  "<OBJ_S_Azimuth_41>"
  Bus Selector:RadarSensor:0_OBJ_S_Azimuth_BS/42 -> RadarSensor:0.OBJ_S_Azimuth_42/1  "<OBJ_S_Azimuth_42>"
  Bus Selector:RadarSensor:0_OBJ_S_Azimuth_BS/43 -> RadarSensor:0.OBJ_S_Azimuth_43/1  "<OBJ_S_Azimuth_43>"
  Bus Selector:RadarSensor:0_OBJ_S_Azimuth_BS/44 -> RadarSensor:0.OBJ_S_Azimuth_44/1  "<OBJ_S_Azimuth_44>"
  Bus Selector:RadarSensor:0_OBJ_S_Azimuth_BS/45 -> RadarSensor:0.OBJ_S_Azimuth_45/1  "<OBJ_S_Azimuth_45>"
  Bus Selector:RadarSensor:0_OBJ_S_Azimuth_BS/46 -> RadarSensor:0.OBJ_S_Azimuth_46/1  "<OBJ_S_Azimuth_46>"
  Bus Selector:RadarSensor:0_OBJ_S_Azimuth_BS/47 -> RadarSensor:0.OBJ_S_Azimuth_47/1  "<OBJ_S_Azimuth_47>"
  Bus Selector:RadarSensor:0_OBJ_S_Azimuth_BS/48 -> RadarSensor:0.OBJ_S_Azimuth_48/1  "<OBJ_S_Azimuth_48>"
  Bus Selector:RadarSensor:0_OBJ_S_Azimuth_BS/49 -> RadarSensor:0.OBJ_S_Azimuth_49/1  "<OBJ_S_Azimuth_49>"
  Bus Selector:RadarSensor:0_OBJ_S_Azimuth_BS/50 -> RadarSensor:0.OBJ_S_Azimuth_50/1  "<OBJ_S_Azimuth_50>"
  Bus Selector:RadarSensor:0_OBJ_S_Azimuth_BS/51 -> RadarSensor:0.OBJ_S_Azimuth_51/1  "<OBJ_S_Azimuth_51>"
  Bus Selector:RadarSensor:0_OBJ_S_Azimuth_BS/52 -> RadarSensor:0.OBJ_S_Azimuth_52/1  "<OBJ_S_Azimuth_52>"
  Bus Selector:RadarSensor:0_OBJ_S_Azimuth_BS/53 -> RadarSensor:0.OBJ_S_Azimuth_53/1  "<OBJ_S_Azimuth_53>"
  Bus Selector:RadarSensor:0_OBJ_S_Azimuth_BS/54 -> RadarSensor:0.OBJ_S_Azimuth_54/1  "<OBJ_S_Azimuth_54>"
  Bus Selector:RadarSensor:0_OBJ_S_Azimuth_BS/55 -> RadarSensor:0.OBJ_S_Azimuth_55/1  "<OBJ_S_Azimuth_55>"
  Bus Selector:RadarSensor:0_OBJ_S_Azimuth_BS/56 -> RadarSensor:0.OBJ_S_Azimuth_56/1  "<OBJ_S_Azimuth_56>"
  Bus Selector:RadarSensor:0_OBJ_S_Azimuth_BS/57 -> RadarSensor:0.OBJ_S_Azimuth_57/1  "<OBJ_S_Azimuth_57>"
  Bus Selector:RadarSensor:0_OBJ_S_Azimuth_BS/58 -> RadarSensor:0.OBJ_S_Azimuth_58/1  "<OBJ_S_Azimuth_58>"
  Bus Selector:RadarSensor:0_OBJ_S_Azimuth_BS/59 -> RadarSensor:0.OBJ_S_Azimuth_59/1  "<OBJ_S_Azimuth_59>"
  Bus Selector:RadarSensor:0_OBJ_S_Azimuth_BS/60 -> RadarSensor:0.OBJ_S_Azimuth_60/1  "<OBJ_S_Azimuth_60>"
  Bus Selector:RadarSensor:0_OBJ_S_Azimuth_BS/61 -> RadarSensor:0.OBJ_S_Azimuth_61/1  "<OBJ_S_Azimuth_61>"
  Bus Selector:RadarSensor:0_OBJ_S_Azimuth_BS/62 -> RadarSensor:0.OBJ_S_Azimuth_62/1  "<OBJ_S_Azimuth_62>"
  Bus Selector:RadarSensor:0_OBJ_S_Azimuth_BS/63 -> RadarSensor:0.OBJ_S_Azimuth_63/1  "<OBJ_S_Azimuth_63>"
  Bus Selector:RadarSensor:0_OBJ_S_Azimuth_BS/64 -> RadarSensor:0.OBJ_S_Azimuth_64/1  "<OBJ_S_Azimuth_64>"
  Bus Selector:RadarSensor:0_OBJ_S_Elevation_BS/1 -> RadarSensor:0.OBJ_S_Elevation_1/1  "<OBJ_S_Elevation_1>"
  Bus Selector:RadarSensor:0_OBJ_S_Elevation_BS/2 -> RadarSensor:0.OBJ_S_Elevation_2/1  "<OBJ_S_Elevation_2>"
  Bus Selector:RadarSensor:0_OBJ_S_Elevation_BS/3 -> RadarSensor:0.OBJ_S_Elevation_3/1  "<OBJ_S_Elevation_3>"
  Bus Selector:RadarSensor:0_OBJ_S_Elevation_BS/4 -> RadarSensor:0.OBJ_S_Elevation_4/1  "<OBJ_S_Elevation_4>"
  Bus Selector:RadarSensor:0_OBJ_S_Elevation_BS/5 -> RadarSensor:0.OBJ_S_Elevation_5/1  "<OBJ_S_Elevation_5>"
  Bus Selector:RadarSensor:0_OBJ_S_Elevation_BS/6 -> RadarSensor:0.OBJ_S_Elevation_6/1  "<OBJ_S_Elevation_6>"
  Bus Selector:RadarSensor:0_OBJ_S_Elevation_BS/7 -> RadarSensor:0.OBJ_S_Elevation_7/1  "<OBJ_S_Elevation_7>"
  Bus Selector:RadarSensor:0_OBJ_S_Elevation_BS/8 -> RadarSensor:0.OBJ_S_Elevation_8/1  "<OBJ_S_Elevation_8>"
  Bus Selector:RadarSensor:0_OBJ_S_Elevation_BS/9 -> RadarSensor:0.OBJ_S_Elevation_9/1  "<OBJ_S_Elevation_9>"
  Bus Selector:RadarSensor:0_OBJ_S_Elevation_BS/10 -> RadarSensor:0.OBJ_S_Elevation_10/1  "<OBJ_S_Elevation_10>"
  Bus Selector:RadarSensor:0_OBJ_S_Elevation_BS/11 -> RadarSensor:0.OBJ_S_Elevation_11/1  "<OBJ_S_Elevation_11>"
  Bus Selector:RadarSensor:0_OBJ_S_Elevation_BS/12 -> RadarSensor:0.OBJ_S_Elevation_12/1  "<OBJ_S_Elevation_12>"
  Bus Selector:RadarSensor:0_OBJ_S_Elevation_BS/13 -> RadarSensor:0.OBJ_S_Elevation_13/1  "<OBJ_S_Elevation_13>"
  Bus Selector:RadarSensor:0_OBJ_S_Elevation_BS/14 -> RadarSensor:0.OBJ_S_Elevation_14/1  "<OBJ_S_Elevation_14>"
  Bus Selector:RadarSensor:0_OBJ_S_Elevation_BS/15 -> RadarSensor:0.OBJ_S_Elevation_15/1  "<OBJ_S_Elevation_15>"
  Bus Selector:RadarSensor:0_OBJ_S_Elevation_BS/16 -> RadarSensor:0.OBJ_S_Elevation_16/1  "<OBJ_S_Elevation_16>"
  Bus Selector:RadarSensor:0_OBJ_S_Elevation_BS/17 -> RadarSensor:0.OBJ_S_Elevation_17/1  "<OBJ_S_Elevation_17>"
  Bus Selector:RadarSensor:0_OBJ_S_Elevation_BS/18 -> RadarSensor:0.OBJ_S_Elevation_18/1  "<OBJ_S_Elevation_18>"
  Bus Selector:RadarSensor:0_OBJ_S_Elevation_BS/19 -> RadarSensor:0.OBJ_S_Elevation_19/1  "<OBJ_S_Elevation_19>"
  Bus Selector:RadarSensor:0_OBJ_S_Elevation_BS/20 -> RadarSensor:0.OBJ_S_Elevation_20/1  "<OBJ_S_Elevation_20>"
  Bus Selector:RadarSensor:0_OBJ_S_Elevation_BS/21 -> RadarSensor:0.OBJ_S_Elevation_21/1  "<OBJ_S_Elevation_21>"
  Bus Selector:RadarSensor:0_OBJ_S_Elevation_BS/22 -> RadarSensor:0.OBJ_S_Elevation_22/1  "<OBJ_S_Elevation_22>"
  Bus Selector:RadarSensor:0_OBJ_S_Elevation_BS/23 -> RadarSensor:0.OBJ_S_Elevation_23/1  "<OBJ_S_Elevation_23>"
  Bus Selector:RadarSensor:0_OBJ_S_Elevation_BS/24 -> RadarSensor:0.OBJ_S_Elevation_24/1  "<OBJ_S_Elevation_24>"
  Bus Selector:RadarSensor:0_OBJ_S_Elevation_BS/25 -> RadarSensor:0.OBJ_S_Elevation_25/1  "<OBJ_S_Elevation_25>"
  Bus Selector:RadarSensor:0_OBJ_S_Elevation_BS/26 -> RadarSensor:0.OBJ_S_Elevation_26/1  "<OBJ_S_Elevation_26>"
  Bus Selector:RadarSensor:0_OBJ_S_Elevation_BS/27 -> RadarSensor:0.OBJ_S_Elevation_27/1  "<OBJ_S_Elevation_27>"
  Bus Selector:RadarSensor:0_OBJ_S_Elevation_BS/28 -> RadarSensor:0.OBJ_S_Elevation_28/1  "<OBJ_S_Elevation_28>"
  Bus Selector:RadarSensor:0_OBJ_S_Elevation_BS/29 -> RadarSensor:0.OBJ_S_Elevation_29/1  "<OBJ_S_Elevation_29>"
  Bus Selector:RadarSensor:0_OBJ_S_Elevation_BS/30 -> RadarSensor:0.OBJ_S_Elevation_30/1  "<OBJ_S_Elevation_30>"
  Bus Selector:RadarSensor:0_OBJ_S_Elevation_BS/31 -> RadarSensor:0.OBJ_S_Elevation_31/1  "<OBJ_S_Elevation_31>"
  Bus Selector:RadarSensor:0_OBJ_S_Elevation_BS/32 -> RadarSensor:0.OBJ_S_Elevation_32/1  "<OBJ_S_Elevation_32>"
  Bus Selector:RadarSensor:0_OBJ_S_Elevation_BS/33 -> RadarSensor:0.OBJ_S_Elevation_33/1  "<OBJ_S_Elevation_33>"
  Bus Selector:RadarSensor:0_OBJ_S_Elevation_BS/34 -> RadarSensor:0.OBJ_S_Elevation_34/1  "<OBJ_S_Elevation_34>"
  Bus Selector:RadarSensor:0_OBJ_S_Elevation_BS/35 -> RadarSensor:0.OBJ_S_Elevation_35/1  "<OBJ_S_Elevation_35>"
  Bus Selector:RadarSensor:0_OBJ_S_Elevation_BS/36 -> RadarSensor:0.OBJ_S_Elevation_36/1  "<OBJ_S_Elevation_36>"
  Bus Selector:RadarSensor:0_OBJ_S_Elevation_BS/37 -> RadarSensor:0.OBJ_S_Elevation_37/1  "<OBJ_S_Elevation_37>"
  Bus Selector:RadarSensor:0_OBJ_S_Elevation_BS/38 -> RadarSensor:0.OBJ_S_Elevation_38/1  "<OBJ_S_Elevation_38>"
  Bus Selector:RadarSensor:0_OBJ_S_Elevation_BS/39 -> RadarSensor:0.OBJ_S_Elevation_39/1  "<OBJ_S_Elevation_39>"
  Bus Selector:RadarSensor:0_OBJ_S_Elevation_BS/40 -> RadarSensor:0.OBJ_S_Elevation_40/1  "<OBJ_S_Elevation_40>"
  Bus Selector:RadarSensor:0_OBJ_S_Elevation_BS/41 -> RadarSensor:0.OBJ_S_Elevation_41/1  "<OBJ_S_Elevation_41>"
  Bus Selector:RadarSensor:0_OBJ_S_Elevation_BS/42 -> RadarSensor:0.OBJ_S_Elevation_42/1  "<OBJ_S_Elevation_42>"
  Bus Selector:RadarSensor:0_OBJ_S_Elevation_BS/43 -> RadarSensor:0.OBJ_S_Elevation_43/1  "<OBJ_S_Elevation_43>"
  Bus Selector:RadarSensor:0_OBJ_S_Elevation_BS/44 -> RadarSensor:0.OBJ_S_Elevation_44/1  "<OBJ_S_Elevation_44>"
  Bus Selector:RadarSensor:0_OBJ_S_Elevation_BS/45 -> RadarSensor:0.OBJ_S_Elevation_45/1  "<OBJ_S_Elevation_45>"
  Bus Selector:RadarSensor:0_OBJ_S_Elevation_BS/46 -> RadarSensor:0.OBJ_S_Elevation_46/1  "<OBJ_S_Elevation_46>"
  Bus Selector:RadarSensor:0_OBJ_S_Elevation_BS/47 -> RadarSensor:0.OBJ_S_Elevation_47/1  "<OBJ_S_Elevation_47>"
  Bus Selector:RadarSensor:0_OBJ_S_Elevation_BS/48 -> RadarSensor:0.OBJ_S_Elevation_48/1  "<OBJ_S_Elevation_48>"
  Bus Selector:RadarSensor:0_OBJ_S_Elevation_BS/49 -> RadarSensor:0.OBJ_S_Elevation_49/1  "<OBJ_S_Elevation_49>"
  Bus Selector:RadarSensor:0_OBJ_S_Elevation_BS/50 -> RadarSensor:0.OBJ_S_Elevation_50/1  "<OBJ_S_Elevation_50>"
  Bus Selector:RadarSensor:0_OBJ_S_Elevation_BS/51 -> RadarSensor:0.OBJ_S_Elevation_51/1  "<OBJ_S_Elevation_51>"
  Bus Selector:RadarSensor:0_OBJ_S_Elevation_BS/52 -> RadarSensor:0.OBJ_S_Elevation_52/1  "<OBJ_S_Elevation_52>"
  Bus Selector:RadarSensor:0_OBJ_S_Elevation_BS/53 -> RadarSensor:0.OBJ_S_Elevation_53/1  "<OBJ_S_Elevation_53>"
  Bus Selector:RadarSensor:0_OBJ_S_Elevation_BS/54 -> RadarSensor:0.OBJ_S_Elevation_54/1  "<OBJ_S_Elevation_54>"
  Bus Selector:RadarSensor:0_OBJ_S_Elevation_BS/55 -> RadarSensor:0.OBJ_S_Elevation_55/1  "<OBJ_S_Elevation_55>"
  Bus Selector:RadarSensor:0_OBJ_S_Elevation_BS/56 -> RadarSensor:0.OBJ_S_Elevation_56/1  "<OBJ_S_Elevation_56>"
  Bus Selector:RadarSensor:0_OBJ_S_Elevation_BS/57 -> RadarSensor:0.OBJ_S_Elevation_57/1  "<OBJ_S_Elevation_57>"
  Bus Selector:RadarSensor:0_OBJ_S_Elevation_BS/58 -> RadarSensor:0.OBJ_S_Elevation_58/1  "<OBJ_S_Elevation_58>"
  Bus Selector:RadarSensor:0_OBJ_S_Elevation_BS/59 -> RadarSensor:0.OBJ_S_Elevation_59/1  "<OBJ_S_Elevation_59>"
  Bus Selector:RadarSensor:0_OBJ_S_Elevation_BS/60 -> RadarSensor:0.OBJ_S_Elevation_60/1  "<OBJ_S_Elevation_60>"
  Bus Selector:RadarSensor:0_OBJ_S_Elevation_BS/61 -> RadarSensor:0.OBJ_S_Elevation_61/1  "<OBJ_S_Elevation_61>"
  Bus Selector:RadarSensor:0_OBJ_S_Elevation_BS/62 -> RadarSensor:0.OBJ_S_Elevation_62/1  "<OBJ_S_Elevation_62>"
  Bus Selector:RadarSensor:0_OBJ_S_Elevation_BS/63 -> RadarSensor:0.OBJ_S_Elevation_63/1  "<OBJ_S_Elevation_63>"
  Bus Selector:RadarSensor:0_OBJ_S_Elevation_BS/64 -> RadarSensor:0.OBJ_S_Elevation_64/1  "<OBJ_S_Elevation_64>"
  Bus Selector:RadarSensor:0_OBJ_S_Velocity_BS/1 -> RadarSensor:0.OBJ_S_Velocity_1/1  "<OBJ_S_Velocity_1>"
  Bus Selector:RadarSensor:0_OBJ_S_Velocity_BS/2 -> RadarSensor:0.OBJ_S_Velocity_2/1  "<OBJ_S_Velocity_2>"
  Bus Selector:RadarSensor:0_OBJ_S_Velocity_BS/3 -> RadarSensor:0.OBJ_S_Velocity_3/1  "<OBJ_S_Velocity_3>"
  Bus Selector:RadarSensor:0_OBJ_S_Velocity_BS/4 -> RadarSensor:0.OBJ_S_Velocity_4/1  "<OBJ_S_Velocity_4>"
  Bus Selector:RadarSensor:0_OBJ_S_Velocity_BS/5 -> RadarSensor:0.OBJ_S_Velocity_5/1  "<OBJ_S_Velocity_5>"
  Bus Selector:RadarSensor:0_OBJ_S_Velocity_BS/6 -> RadarSensor:0.OBJ_S_Velocity_6/1  "<OBJ_S_Velocity_6>"
  Bus Selector:RadarSensor:0_OBJ_S_Velocity_BS/7 -> RadarSensor:0.OBJ_S_Velocity_7/1  "<OBJ_S_Velocity_7>"
  Bus Selector:RadarSensor:0_OBJ_S_Velocity_BS/8 -> RadarSensor:0.OBJ_S_Velocity_8/1  "<OBJ_S_Velocity_8>"
  Bus Selector:RadarSensor:0_OBJ_S_Velocity_BS/9 -> RadarSensor:0.OBJ_S_Velocity_9/1  "<OBJ_S_Velocity_9>"
  Bus Selector:RadarSensor:0_OBJ_S_Velocity_BS/10 -> RadarSensor:0.OBJ_S_Velocity_10/1  "<OBJ_S_Velocity_10>"
  Bus Selector:RadarSensor:0_OBJ_S_Velocity_BS/11 -> RadarSensor:0.OBJ_S_Velocity_11/1  "<OBJ_S_Velocity_11>"
  Bus Selector:RadarSensor:0_OBJ_S_Velocity_BS/12 -> RadarSensor:0.OBJ_S_Velocity_12/1  "<OBJ_S_Velocity_12>"
  Bus Selector:RadarSensor:0_OBJ_S_Velocity_BS/13 -> RadarSensor:0.OBJ_S_Velocity_13/1  "<OBJ_S_Velocity_13>"
  Bus Selector:RadarSensor:0_OBJ_S_Velocity_BS/14 -> RadarSensor:0.OBJ_S_Velocity_14/1  "<OBJ_S_Velocity_14>"
  Bus Selector:RadarSensor:0_OBJ_S_Velocity_BS/15 -> RadarSensor:0.OBJ_S_Velocity_15/1  "<OBJ_S_Velocity_15>"
  Bus Selector:RadarSensor:0_OBJ_S_Velocity_BS/16 -> RadarSensor:0.OBJ_S_Velocity_16/1  "<OBJ_S_Velocity_16>"
  Bus Selector:RadarSensor:0_OBJ_S_Velocity_BS/17 -> RadarSensor:0.OBJ_S_Velocity_17/1  "<OBJ_S_Velocity_17>"
  Bus Selector:RadarSensor:0_OBJ_S_Velocity_BS/18 -> RadarSensor:0.OBJ_S_Velocity_18/1  "<OBJ_S_Velocity_18>"
  Bus Selector:RadarSensor:0_OBJ_S_Velocity_BS/19 -> RadarSensor:0.OBJ_S_Velocity_19/1  "<OBJ_S_Velocity_19>"
  Bus Selector:RadarSensor:0_OBJ_S_Velocity_BS/20 -> RadarSensor:0.OBJ_S_Velocity_20/1  "<OBJ_S_Velocity_20>"
  Bus Selector:RadarSensor:0_OBJ_S_Velocity_BS/21 -> RadarSensor:0.OBJ_S_Velocity_21/1  "<OBJ_S_Velocity_21>"
  Bus Selector:RadarSensor:0_OBJ_S_Velocity_BS/22 -> RadarSensor:0.OBJ_S_Velocity_22/1  "<OBJ_S_Velocity_22>"
  Bus Selector:RadarSensor:0_OBJ_S_Velocity_BS/23 -> RadarSensor:0.OBJ_S_Velocity_23/1  "<OBJ_S_Velocity_23>"
  Bus Selector:RadarSensor:0_OBJ_S_Velocity_BS/24 -> RadarSensor:0.OBJ_S_Velocity_24/1  "<OBJ_S_Velocity_24>"
  Bus Selector:RadarSensor:0_OBJ_S_Velocity_BS/25 -> RadarSensor:0.OBJ_S_Velocity_25/1  "<OBJ_S_Velocity_25>"
  Bus Selector:RadarSensor:0_OBJ_S_Velocity_BS/26 -> RadarSensor:0.OBJ_S_Velocity_26/1  "<OBJ_S_Velocity_26>"
  Bus Selector:RadarSensor:0_OBJ_S_Velocity_BS/27 -> RadarSensor:0.OBJ_S_Velocity_27/1  "<OBJ_S_Velocity_27>"
  Bus Selector:RadarSensor:0_OBJ_S_Velocity_BS/28 -> RadarSensor:0.OBJ_S_Velocity_28/1  "<OBJ_S_Velocity_28>"
  Bus Selector:RadarSensor:0_OBJ_S_Velocity_BS/29 -> RadarSensor:0.OBJ_S_Velocity_29/1  "<OBJ_S_Velocity_29>"
  Bus Selector:RadarSensor:0_OBJ_S_Velocity_BS/30 -> RadarSensor:0.OBJ_S_Velocity_30/1  "<OBJ_S_Velocity_30>"
  Bus Selector:RadarSensor:0_OBJ_S_Velocity_BS/31 -> RadarSensor:0.OBJ_S_Velocity_31/1  "<OBJ_S_Velocity_31>"
  Bus Selector:RadarSensor:0_OBJ_S_Velocity_BS/32 -> RadarSensor:0.OBJ_S_Velocity_32/1  "<OBJ_S_Velocity_32>"
  Bus Selector:RadarSensor:0_OBJ_S_Velocity_BS/33 -> RadarSensor:0.OBJ_S_Velocity_33/1  "<OBJ_S_Velocity_33>"
  Bus Selector:RadarSensor:0_OBJ_S_Velocity_BS/34 -> RadarSensor:0.OBJ_S_Velocity_34/1  "<OBJ_S_Velocity_34>"
  Bus Selector:RadarSensor:0_OBJ_S_Velocity_BS/35 -> RadarSensor:0.OBJ_S_Velocity_35/1  "<OBJ_S_Velocity_35>"
  Bus Selector:RadarSensor:0_OBJ_S_Velocity_BS/36 -> RadarSensor:0.OBJ_S_Velocity_36/1  "<OBJ_S_Velocity_36>"
  Bus Selector:RadarSensor:0_OBJ_S_Velocity_BS/37 -> RadarSensor:0.OBJ_S_Velocity_37/1  "<OBJ_S_Velocity_37>"
  Bus Selector:RadarSensor:0_OBJ_S_Velocity_BS/38 -> RadarSensor:0.OBJ_S_Velocity_38/1  "<OBJ_S_Velocity_38>"
  Bus Selector:RadarSensor:0_OBJ_S_Velocity_BS/39 -> RadarSensor:0.OBJ_S_Velocity_39/1  "<OBJ_S_Velocity_39>"
  Bus Selector:RadarSensor:0_OBJ_S_Velocity_BS/40 -> RadarSensor:0.OBJ_S_Velocity_40/1  "<OBJ_S_Velocity_40>"
  Bus Selector:RadarSensor:0_OBJ_S_Velocity_BS/41 -> RadarSensor:0.OBJ_S_Velocity_41/1  "<OBJ_S_Velocity_41>"
  Bus Selector:RadarSensor:0_OBJ_S_Velocity_BS/42 -> RadarSensor:0.OBJ_S_Velocity_42/1  "<OBJ_S_Velocity_42>"
  Bus Selector:RadarSensor:0_OBJ_S_Velocity_BS/43 -> RadarSensor:0.OBJ_S_Velocity_43/1  "<OBJ_S_Velocity_43>"
  Bus Selector:RadarSensor:0_OBJ_S_Velocity_BS/44 -> RadarSensor:0.OBJ_S_Velocity_44/1  "<OBJ_S_Velocity_44>"
  Bus Selector:RadarSensor:0_OBJ_S_Velocity_BS/45 -> RadarSensor:0.OBJ_S_Velocity_45/1  "<OBJ_S_Velocity_45>"
  Bus Selector:RadarSensor:0_OBJ_S_Velocity_BS/46 -> RadarSensor:0.OBJ_S_Velocity_46/1  "<OBJ_S_Velocity_46>"
  Bus Selector:RadarSensor:0_OBJ_S_Velocity_BS/47 -> RadarSensor:0.OBJ_S_Velocity_47/1  "<OBJ_S_Velocity_47>"
  Bus Selector:RadarSensor:0_OBJ_S_Velocity_BS/48 -> RadarSensor:0.OBJ_S_Velocity_48/1  "<OBJ_S_Velocity_48>"
  Bus Selector:RadarSensor:0_OBJ_S_Velocity_BS/49 -> RadarSensor:0.OBJ_S_Velocity_49/1  "<OBJ_S_Velocity_49>"
  Bus Selector:RadarSensor:0_OBJ_S_Velocity_BS/50 -> RadarSensor:0.OBJ_S_Velocity_50/1  "<OBJ_S_Velocity_50>"
  Bus Selector:RadarSensor:0_OBJ_S_Velocity_BS/51 -> RadarSensor:0.OBJ_S_Velocity_51/1  "<OBJ_S_Velocity_51>"
  Bus Selector:RadarSensor:0_OBJ_S_Velocity_BS/52 -> RadarSensor:0.OBJ_S_Velocity_52/1  "<OBJ_S_Velocity_52>"
  Bus Selector:RadarSensor:0_OBJ_S_Velocity_BS/53 -> RadarSensor:0.OBJ_S_Velocity_53/1  "<OBJ_S_Velocity_53>"
  Bus Selector:RadarSensor:0_OBJ_S_Velocity_BS/54 -> RadarSensor:0.OBJ_S_Velocity_54/1  "<OBJ_S_Velocity_54>"
  Bus Selector:RadarSensor:0_OBJ_S_Velocity_BS/55 -> RadarSensor:0.OBJ_S_Velocity_55/1  "<OBJ_S_Velocity_55>"
  Bus Selector:RadarSensor:0_OBJ_S_Velocity_BS/56 -> RadarSensor:0.OBJ_S_Velocity_56/1  "<OBJ_S_Velocity_56>"
  Bus Selector:RadarSensor:0_OBJ_S_Velocity_BS/57 -> RadarSensor:0.OBJ_S_Velocity_57/1  "<OBJ_S_Velocity_57>"
  Bus Selector:RadarSensor:0_OBJ_S_Velocity_BS/58 -> RadarSensor:0.OBJ_S_Velocity_58/1  "<OBJ_S_Velocity_58>"
  Bus Selector:RadarSensor:0_OBJ_S_Velocity_BS/59 -> RadarSensor:0.OBJ_S_Velocity_59/1  "<OBJ_S_Velocity_59>"
  Bus Selector:RadarSensor:0_OBJ_S_Velocity_BS/60 -> RadarSensor:0.OBJ_S_Velocity_60/1  "<OBJ_S_Velocity_60>"
  Bus Selector:RadarSensor:0_OBJ_S_Velocity_BS/61 -> RadarSensor:0.OBJ_S_Velocity_61/1  "<OBJ_S_Velocity_61>"
  Bus Selector:RadarSensor:0_OBJ_S_Velocity_BS/62 -> RadarSensor:0.OBJ_S_Velocity_62/1  "<OBJ_S_Velocity_62>"
  Bus Selector:RadarSensor:0_OBJ_S_Velocity_BS/63 -> RadarSensor:0.OBJ_S_Velocity_63/1  "<OBJ_S_Velocity_63>"
  Bus Selector:RadarSensor:0_OBJ_S_Velocity_BS/64 -> RadarSensor:0.OBJ_S_Velocity_64/1  "<OBJ_S_Velocity_64>"
  Bus Selector:RadarSensor:0_OBJ_S_Range_BS/1 -> RadarSensor:0.OBJ_S_Range_1/1  "<OBJ_S_Range_1>"
  Bus Selector:RadarSensor:0_OBJ_S_Range_BS/2 -> RadarSensor:0.OBJ_S_Range_2/1  "<OBJ_S_Range_2>"
  Bus Selector:RadarSensor:0_OBJ_S_Range_BS/3 -> RadarSensor:0.OBJ_S_Range_3/1  "<OBJ_S_Range_3>"
  Bus Selector:RadarSensor:0_OBJ_S_Range_BS/4 -> RadarSensor:0.OBJ_S_Range_4/1  "<OBJ_S_Range_4>"
  Bus Selector:RadarSensor:0_OBJ_S_Range_BS/5 -> RadarSensor:0.OBJ_S_Range_5/1  "<OBJ_S_Range_5>"
  Bus Selector:RadarSensor:0_OBJ_S_Range_BS/6 -> RadarSensor:0.OBJ_S_Range_6/1  "<OBJ_S_Range_6>"
  Bus Selector:RadarSensor:0_OBJ_S_Range_BS/7 -> RadarSensor:0.OBJ_S_Range_7/1  "<OBJ_S_Range_7>"
  Bus Selector:RadarSensor:0_OBJ_S_Range_BS/8 -> RadarSensor:0.OBJ_S_Range_8/1  "<OBJ_S_Range_8>"
  Bus Selector:RadarSensor:0_OBJ_S_Range_BS/9 -> RadarSensor:0.OBJ_S_Range_9/1  "<OBJ_S_Range_9>"
  Bus Selector:RadarSensor:0_OBJ_S_Range_BS/10 -> RadarSensor:0.OBJ_S_Range_10/1  "<OBJ_S_Range_10>"
  Bus Selector:RadarSensor:0_OBJ_S_Range_BS/11 -> RadarSensor:0.OBJ_S_Range_11/1  "<OBJ_S_Range_11>"
  Bus Selector:RadarSensor:0_OBJ_S_Range_BS/12 -> RadarSensor:0.OBJ_S_Range_12/1  "<OBJ_S_Range_12>"
  Bus Selector:RadarSensor:0_OBJ_S_Range_BS/13 -> RadarSensor:0.OBJ_S_Range_13/1  "<OBJ_S_Range_13>"
  Bus Selector:RadarSensor:0_OBJ_S_Range_BS/14 -> RadarSensor:0.OBJ_S_Range_14/1  "<OBJ_S_Range_14>"
  Bus Selector:RadarSensor:0_OBJ_S_Range_BS/15 -> RadarSensor:0.OBJ_S_Range_15/1  "<OBJ_S_Range_15>"
  Bus Selector:RadarSensor:0_OBJ_S_Range_BS/16 -> RadarSensor:0.OBJ_S_Range_16/1  "<OBJ_S_Range_16>"
  Bus Selector:RadarSensor:0_OBJ_S_Range_BS/17 -> RadarSensor:0.OBJ_S_Range_17/1  "<OBJ_S_Range_17>"
  Bus Selector:RadarSensor:0_OBJ_S_Range_BS/18 -> RadarSensor:0.OBJ_S_Range_18/1  "<OBJ_S_Range_18>"
  Bus Selector:RadarSensor:0_OBJ_S_Range_BS/19 -> RadarSensor:0.OBJ_S_Range_19/1  "<OBJ_S_Range_19>"
  Bus Selector:RadarSensor:0_OBJ_S_Range_BS/20 -> RadarSensor:0.OBJ_S_Range_20/1  "<OBJ_S_Range_20>"
  Bus Selector:RadarSensor:0_OBJ_S_Range_BS/21 -> RadarSensor:0.OBJ_S_Range_21/1  "<OBJ_S_Range_21>"
  Bus Selector:RadarSensor:0_OBJ_S_Range_BS/22 -> RadarSensor:0.OBJ_S_Range_22/1  "<OBJ_S_Range_22>"
  Bus Selector:RadarSensor:0_OBJ_S_Range_BS/23 -> RadarSensor:0.OBJ_S_Range_23/1  "<OBJ_S_Range_23>"
  Bus Selector:RadarSensor:0_OBJ_S_Range_BS/24 -> RadarSensor:0.OBJ_S_Range_24/1  "<OBJ_S_Range_24>"
  Bus Selector:RadarSensor:0_OBJ_S_Range_BS/25 -> RadarSensor:0.OBJ_S_Range_25/1  "<OBJ_S_Range_25>"
  Bus Selector:RadarSensor:0_OBJ_S_Range_BS/26 -> RadarSensor:0.OBJ_S_Range_26/1  "<OBJ_S_Range_26>"
  Bus Selector:RadarSensor:0_OBJ_S_Range_BS/27 -> RadarSensor:0.OBJ_S_Range_27/1  "<OBJ_S_Range_27>"
  Bus Selector:RadarSensor:0_OBJ_S_Range_BS/28 -> RadarSensor:0.OBJ_S_Range_28/1  "<OBJ_S_Range_28>"
  Bus Selector:RadarSensor:0_OBJ_S_Range_BS/29 -> RadarSensor:0.OBJ_S_Range_29/1  "<OBJ_S_Range_29>"
  Bus Selector:RadarSensor:0_OBJ_S_Range_BS/30 -> RadarSensor:0.OBJ_S_Range_30/1  "<OBJ_S_Range_30>"
  Bus Selector:RadarSensor:0_OBJ_S_Range_BS/31 -> RadarSensor:0.OBJ_S_Range_31/1  "<OBJ_S_Range_31>"
  Bus Selector:RadarSensor:0_OBJ_S_Range_BS/32 -> RadarSensor:0.OBJ_S_Range_32/1  "<OBJ_S_Range_32>"
  Bus Selector:RadarSensor:0_OBJ_S_Range_BS/33 -> RadarSensor:0.OBJ_S_Range_33/1  "<OBJ_S_Range_33>"
  Bus Selector:RadarSensor:0_OBJ_S_Range_BS/34 -> RadarSensor:0.OBJ_S_Range_34/1  "<OBJ_S_Range_34>"
  Bus Selector:RadarSensor:0_OBJ_S_Range_BS/35 -> RadarSensor:0.OBJ_S_Range_35/1  "<OBJ_S_Range_35>"
  Bus Selector:RadarSensor:0_OBJ_S_Range_BS/36 -> RadarSensor:0.OBJ_S_Range_36/1  "<OBJ_S_Range_36>"
  Bus Selector:RadarSensor:0_OBJ_S_Range_BS/37 -> RadarSensor:0.OBJ_S_Range_37/1  "<OBJ_S_Range_37>"
  Bus Selector:RadarSensor:0_OBJ_S_Range_BS/38 -> RadarSensor:0.OBJ_S_Range_38/1  "<OBJ_S_Range_38>"
  Bus Selector:RadarSensor:0_OBJ_S_Range_BS/39 -> RadarSensor:0.OBJ_S_Range_39/1  "<OBJ_S_Range_39>"
  Bus Selector:RadarSensor:0_OBJ_S_Range_BS/40 -> RadarSensor:0.OBJ_S_Range_40/1  "<OBJ_S_Range_40>"
  Bus Selector:RadarSensor:0_OBJ_S_Range_BS/41 -> RadarSensor:0.OBJ_S_Range_41/1  "<OBJ_S_Range_41>"
  Bus Selector:RadarSensor:0_OBJ_S_Range_BS/42 -> RadarSensor:0.OBJ_S_Range_42/1  "<OBJ_S_Range_42>"
  Bus Selector:RadarSensor:0_OBJ_S_Range_BS/43 -> RadarSensor:0.OBJ_S_Range_43/1  "<OBJ_S_Range_43>"
  Bus Selector:RadarSensor:0_OBJ_S_Range_BS/44 -> RadarSensor:0.OBJ_S_Range_44/1  "<OBJ_S_Range_44>"
  Bus Selector:RadarSensor:0_OBJ_S_Range_BS/45 -> RadarSensor:0.OBJ_S_Range_45/1  "<OBJ_S_Range_45>"
  Bus Selector:RadarSensor:0_OBJ_S_Range_BS/46 -> RadarSensor:0.OBJ_S_Range_46/1  "<OBJ_S_Range_46>"
  Bus Selector:RadarSensor:0_OBJ_S_Range_BS/47 -> RadarSensor:0.OBJ_S_Range_47/1  "<OBJ_S_Range_47>"
  Bus Selector:RadarSensor:0_OBJ_S_Range_BS/48 -> RadarSensor:0.OBJ_S_Range_48/1  "<OBJ_S_Range_48>"
  Bus Selector:RadarSensor:0_OBJ_S_Range_BS/49 -> RadarSensor:0.OBJ_S_Range_49/1  "<OBJ_S_Range_49>"
  Bus Selector:RadarSensor:0_OBJ_S_Range_BS/50 -> RadarSensor:0.OBJ_S_Range_50/1  "<OBJ_S_Range_50>"
  Bus Selector:RadarSensor:0_OBJ_S_Range_BS/51 -> RadarSensor:0.OBJ_S_Range_51/1  "<OBJ_S_Range_51>"
  Bus Selector:RadarSensor:0_OBJ_S_Range_BS/52 -> RadarSensor:0.OBJ_S_Range_52/1  "<OBJ_S_Range_52>"
  Bus Selector:RadarSensor:0_OBJ_S_Range_BS/53 -> RadarSensor:0.OBJ_S_Range_53/1  "<OBJ_S_Range_53>"
  Bus Selector:RadarSensor:0_OBJ_S_Range_BS/54 -> RadarSensor:0.OBJ_S_Range_54/1  "<OBJ_S_Range_54>"
  Bus Selector:RadarSensor:0_OBJ_S_Range_BS/55 -> RadarSensor:0.OBJ_S_Range_55/1  "<OBJ_S_Range_55>"
  Bus Selector:RadarSensor:0_OBJ_S_Range_BS/56 -> RadarSensor:0.OBJ_S_Range_56/1  "<OBJ_S_Range_56>"
  Bus Selector:RadarSensor:0_OBJ_S_Range_BS/57 -> RadarSensor:0.OBJ_S_Range_57/1  "<OBJ_S_Range_57>"
  Bus Selector:RadarSensor:0_OBJ_S_Range_BS/58 -> RadarSensor:0.OBJ_S_Range_58/1  "<OBJ_S_Range_58>"
  Bus Selector:RadarSensor:0_OBJ_S_Range_BS/59 -> RadarSensor:0.OBJ_S_Range_59/1  "<OBJ_S_Range_59>"
  Bus Selector:RadarSensor:0_OBJ_S_Range_BS/60 -> RadarSensor:0.OBJ_S_Range_60/1  "<OBJ_S_Range_60>"
  Bus Selector:RadarSensor:0_OBJ_S_Range_BS/61 -> RadarSensor:0.OBJ_S_Range_61/1  "<OBJ_S_Range_61>"
  Bus Selector:RadarSensor:0_OBJ_S_Range_BS/62 -> RadarSensor:0.OBJ_S_Range_62/1  "<OBJ_S_Range_62>"
  Bus Selector:RadarSensor:0_OBJ_S_Range_BS/63 -> RadarSensor:0.OBJ_S_Range_63/1  "<OBJ_S_Range_63>"
  Bus Selector:RadarSensor:0_OBJ_S_Range_BS/64 -> RadarSensor:0.OBJ_S_Range_64/1  "<OBJ_S_Range_64>"
  Bus Selector:RadarSensor:0_OBJ_RCS_BS/1 -> RadarSensor:0.OBJ_RCS_1/1  "<OBJ_RCS_1>"
  Bus Selector:RadarSensor:0_OBJ_RCS_BS/2 -> RadarSensor:0.OBJ_RCS_2/1  "<OBJ_RCS_2>"
  Bus Selector:RadarSensor:0_OBJ_RCS_BS/3 -> RadarSensor:0.OBJ_RCS_3/1  "<OBJ_RCS_3>"
  Bus Selector:RadarSensor:0_OBJ_RCS_BS/4 -> RadarSensor:0.OBJ_RCS_4/1  "<OBJ_RCS_4>"
  Bus Selector:RadarSensor:0_OBJ_RCS_BS/5 -> RadarSensor:0.OBJ_RCS_5/1  "<OBJ_RCS_5>"
  Bus Selector:RadarSensor:0_OBJ_RCS_BS/6 -> RadarSensor:0.OBJ_RCS_6/1  "<OBJ_RCS_6>"
  Bus Selector:RadarSensor:0_OBJ_RCS_BS/7 -> RadarSensor:0.OBJ_RCS_7/1  "<OBJ_RCS_7>"
  Bus Selector:RadarSensor:0_OBJ_RCS_BS/8 -> RadarSensor:0.OBJ_RCS_8/1  "<OBJ_RCS_8>"
  Bus Selector:RadarSensor:0_OBJ_RCS_BS/9 -> RadarSensor:0.OBJ_RCS_9/1  "<OBJ_RCS_9>"
  Bus Selector:RadarSensor:0_OBJ_RCS_BS/10 -> RadarSensor:0.OBJ_RCS_10/1  "<OBJ_RCS_10>"
  Bus Selector:RadarSensor:0_OBJ_RCS_BS/11 -> RadarSensor:0.OBJ_RCS_11/1  "<OBJ_RCS_11>"
  Bus Selector:RadarSensor:0_OBJ_RCS_BS/12 -> RadarSensor:0.OBJ_RCS_12/1  "<OBJ_RCS_12>"
  Bus Selector:RadarSensor:0_OBJ_RCS_BS/13 -> RadarSensor:0.OBJ_RCS_13/1  "<OBJ_RCS_13>"
  Bus Selector:RadarSensor:0_OBJ_RCS_BS/14 -> RadarSensor:0.OBJ_RCS_14/1  "<OBJ_RCS_14>"
  Bus Selector:RadarSensor:0_OBJ_RCS_BS/15 -> RadarSensor:0.OBJ_RCS_15/1  "<OBJ_RCS_15>"
  Bus Selector:RadarSensor:0_OBJ_RCS_BS/16 -> RadarSensor:0.OBJ_RCS_16/1  "<OBJ_RCS_16>"
  Bus Selector:RadarSensor:0_OBJ_RCS_BS/17 -> RadarSensor:0.OBJ_RCS_17/1  "<OBJ_RCS_17>"
  Bus Selector:RadarSensor:0_OBJ_RCS_BS/18 -> RadarSensor:0.OBJ_RCS_18/1  "<OBJ_RCS_18>"
  Bus Selector:RadarSensor:0_OBJ_RCS_BS/19 -> RadarSensor:0.OBJ_RCS_19/1  "<OBJ_RCS_19>"
  Bus Selector:RadarSensor:0_OBJ_RCS_BS/20 -> RadarSensor:0.OBJ_RCS_20/1  "<OBJ_RCS_20>"
  Bus Selector:RadarSensor:0_OBJ_RCS_BS/21 -> RadarSensor:0.OBJ_RCS_21/1  "<OBJ_RCS_21>"
  Bus Selector:RadarSensor:0_OBJ_RCS_BS/22 -> RadarSensor:0.OBJ_RCS_22/1  "<OBJ_RCS_22>"
  Bus Selector:RadarSensor:0_OBJ_RCS_BS/23 -> RadarSensor:0.OBJ_RCS_23/1  "<OBJ_RCS_23>"
  Bus Selector:RadarSensor:0_OBJ_RCS_BS/24 -> RadarSensor:0.OBJ_RCS_24/1  "<OBJ_RCS_24>"
  Bus Selector:RadarSensor:0_OBJ_RCS_BS/25 -> RadarSensor:0.OBJ_RCS_25/1  "<OBJ_RCS_25>"
  Bus Selector:RadarSensor:0_OBJ_RCS_BS/26 -> RadarSensor:0.OBJ_RCS_26/1  "<OBJ_RCS_26>"
  Bus Selector:RadarSensor:0_OBJ_RCS_BS/27 -> RadarSensor:0.OBJ_RCS_27/1  "<OBJ_RCS_27>"
  Bus Selector:RadarSensor:0_OBJ_RCS_BS/28 -> RadarSensor:0.OBJ_RCS_28/1  "<OBJ_RCS_28>"
  Bus Selector:RadarSensor:0_OBJ_RCS_BS/29 -> RadarSensor:0.OBJ_RCS_29/1  "<OBJ_RCS_29>"
  Bus Selector:RadarSensor:0_OBJ_RCS_BS/30 -> RadarSensor:0.OBJ_RCS_30/1  "<OBJ_RCS_30>"
  Bus Selector:RadarSensor:0_OBJ_RCS_BS/31 -> RadarSensor:0.OBJ_RCS_31/1  "<OBJ_RCS_31>"
  Bus Selector:RadarSensor:0_OBJ_RCS_BS/32 -> RadarSensor:0.OBJ_RCS_32/1  "<OBJ_RCS_32>"
  Bus Selector:RadarSensor:0_OBJ_RCS_BS/33 -> RadarSensor:0.OBJ_RCS_33/1  "<OBJ_RCS_33>"
  Bus Selector:RadarSensor:0_OBJ_RCS_BS/34 -> RadarSensor:0.OBJ_RCS_34/1  "<OBJ_RCS_34>"
  Bus Selector:RadarSensor:0_OBJ_RCS_BS/35 -> RadarSensor:0.OBJ_RCS_35/1  "<OBJ_RCS_35>"
  Bus Selector:RadarSensor:0_OBJ_RCS_BS/36 -> RadarSensor:0.OBJ_RCS_36/1  "<OBJ_RCS_36>"
  Bus Selector:RadarSensor:0_OBJ_RCS_BS/37 -> RadarSensor:0.OBJ_RCS_37/1  "<OBJ_RCS_37>"
  Bus Selector:RadarSensor:0_OBJ_RCS_BS/38 -> RadarSensor:0.OBJ_RCS_38/1  "<OBJ_RCS_38>"
  Bus Selector:RadarSensor:0_OBJ_RCS_BS/39 -> RadarSensor:0.OBJ_RCS_39/1  "<OBJ_RCS_39>"
  Bus Selector:RadarSensor:0_OBJ_RCS_BS/40 -> RadarSensor:0.OBJ_RCS_40/1  "<OBJ_RCS_40>"
  Bus Selector:RadarSensor:0_OBJ_RCS_BS/41 -> RadarSensor:0.OBJ_RCS_41/1  "<OBJ_RCS_41>"
  Bus Selector:RadarSensor:0_OBJ_RCS_BS/42 -> RadarSensor:0.OBJ_RCS_42/1  "<OBJ_RCS_42>"
  Bus Selector:RadarSensor:0_OBJ_RCS_BS/43 -> RadarSensor:0.OBJ_RCS_43/1  "<OBJ_RCS_43>"
  Bus Selector:RadarSensor:0_OBJ_RCS_BS/44 -> RadarSensor:0.OBJ_RCS_44/1  "<OBJ_RCS_44>"
  Bus Selector:RadarSensor:0_OBJ_RCS_BS/45 -> RadarSensor:0.OBJ_RCS_45/1  "<OBJ_RCS_45>"
  Bus Selector:RadarSensor:0_OBJ_RCS_BS/46 -> RadarSensor:0.OBJ_RCS_46/1  "<OBJ_RCS_46>"
  Bus Selector:RadarSensor:0_OBJ_RCS_BS/47 -> RadarSensor:0.OBJ_RCS_47/1  "<OBJ_RCS_47>"
  Bus Selector:RadarSensor:0_OBJ_RCS_BS/48 -> RadarSensor:0.OBJ_RCS_48/1  "<OBJ_RCS_48>"
  Bus Selector:RadarSensor:0_OBJ_RCS_BS/49 -> RadarSensor:0.OBJ_RCS_49/1  "<OBJ_RCS_49>"
  Bus Selector:RadarSensor:0_OBJ_RCS_BS/50 -> RadarSensor:0.OBJ_RCS_50/1  "<OBJ_RCS_50>"
  Bus Selector:RadarSensor:0_OBJ_RCS_BS/51 -> RadarSensor:0.OBJ_RCS_51/1  "<OBJ_RCS_51>"
  Bus Selector:RadarSensor:0_OBJ_RCS_BS/52 -> RadarSensor:0.OBJ_RCS_52/1  "<OBJ_RCS_52>"
  Bus Selector:RadarSensor:0_OBJ_RCS_BS/53 -> RadarSensor:0.OBJ_RCS_53/1  "<OBJ_RCS_53>"
  Bus Selector:RadarSensor:0_OBJ_RCS_BS/54 -> RadarSensor:0.OBJ_RCS_54/1  "<OBJ_RCS_54>"
  Bus Selector:RadarSensor:0_OBJ_RCS_BS/55 -> RadarSensor:0.OBJ_RCS_55/1  "<OBJ_RCS_55>"
  Bus Selector:RadarSensor:0_OBJ_RCS_BS/56 -> RadarSensor:0.OBJ_RCS_56/1  "<OBJ_RCS_56>"
  Bus Selector:RadarSensor:0_OBJ_RCS_BS/57 -> RadarSensor:0.OBJ_RCS_57/1  "<OBJ_RCS_57>"
  Bus Selector:RadarSensor:0_OBJ_RCS_BS/58 -> RadarSensor:0.OBJ_RCS_58/1  "<OBJ_RCS_58>"
  Bus Selector:RadarSensor:0_OBJ_RCS_BS/59 -> RadarSensor:0.OBJ_RCS_59/1  "<OBJ_RCS_59>"
  Bus Selector:RadarSensor:0_OBJ_RCS_BS/60 -> RadarSensor:0.OBJ_RCS_60/1  "<OBJ_RCS_60>"
  Bus Selector:RadarSensor:0_OBJ_RCS_BS/61 -> RadarSensor:0.OBJ_RCS_61/1  "<OBJ_RCS_61>"
  Bus Selector:RadarSensor:0_OBJ_RCS_BS/62 -> RadarSensor:0.OBJ_RCS_62/1  "<OBJ_RCS_62>"
  Bus Selector:RadarSensor:0_OBJ_RCS_BS/63 -> RadarSensor:0.OBJ_RCS_63/1  "<OBJ_RCS_63>"
  Bus Selector:RadarSensor:0_OBJ_RCS_BS/64 -> RadarSensor:0.OBJ_RCS_64/1  "<OBJ_RCS_64>"
  Bus Selector:RadarSensor:0/1 -> RadarSensor:0.time/1  "<time>"
  Bus Selector:RadarSensor:0/2 -> RadarSensor:0.width/1  "<width>"
  Bus Selector:RadarSensor:0/3 -> RadarSensor:0.OBJ_ID/1, Bus Selector:RadarSensor:0_OBJ_ID_BS/1  "<OBJ_ID>"
  Bus Selector:RadarSensor:0/4 -> RadarSensor:0.OBJ_Class/1, Bus Selector:RadarSensor:0_OBJ_Class_BS/1  "<OBJ_Class>"
  Bus Selector:RadarSensor:0/5 -> RadarSensor:0.OBJ_S_Azimuth/1, Bus Selector:RadarSensor:0_OBJ_S_Azimuth_BS/1  "<OBJ_S_Azimuth>"
  Bus Selector:RadarSensor:0/6 -> RadarSensor:0.OBJ_S_Elevation/1, Bus Selector:RadarSensor:0_OBJ_S_Elevation_BS/1  "<OBJ_S_Elevation>"
  Bus Selector:RadarSensor:0/7 -> RadarSensor:0.OBJ_S_Velocity/1, Bus Selector:RadarSensor:0_OBJ_S_Velocity_BS/1  "<OBJ_S_Velocity>"
  Bus Selector:RadarSensor:0/8 -> RadarSensor:0.OBJ_S_Range/1, Bus Selector:RadarSensor:0_OBJ_S_Range_BS/1  "<OBJ_S_Range>"
  Bus Selector:RadarSensor:0/9 -> RadarSensor:0.OBJ_RCS/1, Bus Selector:RadarSensor:0_OBJ_RCS_BS/1  "<OBJ_RCS>"
  Bus Selector:RadarSensor:1_OBJ_ID_BS/1 -> RadarSensor:1.OBJ_ID_1/1  "<OBJ_ID_1>"
  Bus Selector:RadarSensor:1_OBJ_ID_BS/2 -> RadarSensor:1.OBJ_ID_2/1  "<OBJ_ID_2>"
  Bus Selector:RadarSensor:1_OBJ_ID_BS/3 -> RadarSensor:1.OBJ_ID_3/1  "<OBJ_ID_3>"
  Bus Selector:RadarSensor:1_OBJ_ID_BS/4 -> RadarSensor:1.OBJ_ID_4/1  "<OBJ_ID_4>"
  Bus Selector:RadarSensor:1_OBJ_ID_BS/5 -> RadarSensor:1.OBJ_ID_5/1  "<OBJ_ID_5>"
  Bus Selector:RadarSensor:1_OBJ_ID_BS/6 -> RadarSensor:1.OBJ_ID_6/1  "<OBJ_ID_6>"
  Bus Selector:RadarSensor:1_OBJ_ID_BS/7 -> RadarSensor:1.OBJ_ID_7/1  "<OBJ_ID_7>"
  Bus Selector:RadarSensor:1_OBJ_ID_BS/8 -> RadarSensor:1.OBJ_ID_8/1  "<OBJ_ID_8>"
  Bus Selector:RadarSensor:1_OBJ_ID_BS/9 -> RadarSensor:1.OBJ_ID_9/1  "<OBJ_ID_9>"
  Bus Selector:RadarSensor:1_OBJ_ID_BS/10 -> RadarSensor:1.OBJ_ID_10/1  "<OBJ_ID_10>"
  Bus Selector:RadarSensor:1_OBJ_ID_BS/11 -> RadarSensor:1.OBJ_ID_11/1  "<OBJ_ID_11>"
  Bus Selector:RadarSensor:1_OBJ_ID_BS/12 -> RadarSensor:1.OBJ_ID_12/1  "<OBJ_ID_12>"
  Bus Selector:RadarSensor:1_OBJ_ID_BS/13 -> RadarSensor:1.OBJ_ID_13/1  "<OBJ_ID_13>"
  Bus Selector:RadarSensor:1_OBJ_ID_BS/14 -> RadarSensor:1.OBJ_ID_14/1  "<OBJ_ID_14>"
  Bus Selector:RadarSensor:1_OBJ_ID_BS/15 -> RadarSensor:1.OBJ_ID_15/1  "<OBJ_ID_15>"
  Bus Selector:RadarSensor:1_OBJ_ID_BS/16 -> RadarSensor:1.OBJ_ID_16/1  "<OBJ_ID_16>"
  Bus Selector:RadarSensor:1_OBJ_ID_BS/17 -> RadarSensor:1.OBJ_ID_17/1  "<OBJ_ID_17>"
  Bus Selector:RadarSensor:1_OBJ_ID_BS/18 -> RadarSensor:1.OBJ_ID_18/1  "<OBJ_ID_18>"
  Bus Selector:RadarSensor:1_OBJ_ID_BS/19 -> RadarSensor:1.OBJ_ID_19/1  "<OBJ_ID_19>"
  Bus Selector:RadarSensor:1_OBJ_ID_BS/20 -> RadarSensor:1.OBJ_ID_20/1  "<OBJ_ID_20>"
  Bus Selector:RadarSensor:1_OBJ_ID_BS/21 -> RadarSensor:1.OBJ_ID_21/1  "<OBJ_ID_21>"
  Bus Selector:RadarSensor:1_OBJ_ID_BS/22 -> RadarSensor:1.OBJ_ID_22/1  "<OBJ_ID_22>"
  Bus Selector:RadarSensor:1_OBJ_ID_BS/23 -> RadarSensor:1.OBJ_ID_23/1  "<OBJ_ID_23>"
  Bus Selector:RadarSensor:1_OBJ_ID_BS/24 -> RadarSensor:1.OBJ_ID_24/1  "<OBJ_ID_24>"
  Bus Selector:RadarSensor:1_OBJ_ID_BS/25 -> RadarSensor:1.OBJ_ID_25/1  "<OBJ_ID_25>"
  Bus Selector:RadarSensor:1_OBJ_ID_BS/26 -> RadarSensor:1.OBJ_ID_26/1  "<OBJ_ID_26>"
  Bus Selector:RadarSensor:1_OBJ_ID_BS/27 -> RadarSensor:1.OBJ_ID_27/1  "<OBJ_ID_27>"
  Bus Selector:RadarSensor:1_OBJ_ID_BS/28 -> RadarSensor:1.OBJ_ID_28/1  "<OBJ_ID_28>"
  Bus Selector:RadarSensor:1_OBJ_ID_BS/29 -> RadarSensor:1.OBJ_ID_29/1  "<OBJ_ID_29>"
  Bus Selector:RadarSensor:1_OBJ_ID_BS/30 -> RadarSensor:1.OBJ_ID_30/1  "<OBJ_ID_30>"
  Bus Selector:RadarSensor:1_OBJ_ID_BS/31 -> RadarSensor:1.OBJ_ID_31/1  "<OBJ_ID_31>"
  Bus Selector:RadarSensor:1_OBJ_ID_BS/32 -> RadarSensor:1.OBJ_ID_32/1  "<OBJ_ID_32>"
  Bus Selector:RadarSensor:1_OBJ_ID_BS/33 -> RadarSensor:1.OBJ_ID_33/1  "<OBJ_ID_33>"
  Bus Selector:RadarSensor:1_OBJ_ID_BS/34 -> RadarSensor:1.OBJ_ID_34/1  "<OBJ_ID_34>"
  Bus Selector:RadarSensor:1_OBJ_ID_BS/35 -> RadarSensor:1.OBJ_ID_35/1  "<OBJ_ID_35>"
  Bus Selector:RadarSensor:1_OBJ_ID_BS/36 -> RadarSensor:1.OBJ_ID_36/1  "<OBJ_ID_36>"
  Bus Selector:RadarSensor:1_OBJ_ID_BS/37 -> RadarSensor:1.OBJ_ID_37/1  "<OBJ_ID_37>"
  Bus Selector:RadarSensor:1_OBJ_ID_BS/38 -> RadarSensor:1.OBJ_ID_38/1  "<OBJ_ID_38>"
  Bus Selector:RadarSensor:1_OBJ_ID_BS/39 -> RadarSensor:1.OBJ_ID_39/1  "<OBJ_ID_39>"
  Bus Selector:RadarSensor:1_OBJ_ID_BS/40 -> RadarSensor:1.OBJ_ID_40/1  "<OBJ_ID_40>"
  Bus Selector:RadarSensor:1_OBJ_ID_BS/41 -> RadarSensor:1.OBJ_ID_41/1  "<OBJ_ID_41>"
  Bus Selector:RadarSensor:1_OBJ_ID_BS/42 -> RadarSensor:1.OBJ_ID_42/1  "<OBJ_ID_42>"
  Bus Selector:RadarSensor:1_OBJ_ID_BS/43 -> RadarSensor:1.OBJ_ID_43/1  "<OBJ_ID_43>"
  Bus Selector:RadarSensor:1_OBJ_ID_BS/44 -> RadarSensor:1.OBJ_ID_44/1  "<OBJ_ID_44>"
  Bus Selector:RadarSensor:1_OBJ_ID_BS/45 -> RadarSensor:1.OBJ_ID_45/1  "<OBJ_ID_45>"
  Bus Selector:RadarSensor:1_OBJ_ID_BS/46 -> RadarSensor:1.OBJ_ID_46/1  "<OBJ_ID_46>"
  Bus Selector:RadarSensor:1_OBJ_ID_BS/47 -> RadarSensor:1.OBJ_ID_47/1  "<OBJ_ID_47>"
  Bus Selector:RadarSensor:1_OBJ_ID_BS/48 -> RadarSensor:1.OBJ_ID_48/1  "<OBJ_ID_48>"
  Bus Selector:RadarSensor:1_OBJ_ID_BS/49 -> RadarSensor:1.OBJ_ID_49/1  "<OBJ_ID_49>"
  Bus Selector:RadarSensor:1_OBJ_ID_BS/50 -> RadarSensor:1.OBJ_ID_50/1  "<OBJ_ID_50>"
  Bus Selector:RadarSensor:1_OBJ_ID_BS/51 -> RadarSensor:1.OBJ_ID_51/1  "<OBJ_ID_51>"
  Bus Selector:RadarSensor:1_OBJ_ID_BS/52 -> RadarSensor:1.OBJ_ID_52/1  "<OBJ_ID_52>"
  Bus Selector:RadarSensor:1_OBJ_ID_BS/53 -> RadarSensor:1.OBJ_ID_53/1  "<OBJ_ID_53>"
  Bus Selector:RadarSensor:1_OBJ_ID_BS/54 -> RadarSensor:1.OBJ_ID_54/1  "<OBJ_ID_54>"
  Bus Selector:RadarSensor:1_OBJ_ID_BS/55 -> RadarSensor:1.OBJ_ID_55/1  "<OBJ_ID_55>"
  Bus Selector:RadarSensor:1_OBJ_ID_BS/56 -> RadarSensor:1.OBJ_ID_56/1  "<OBJ_ID_56>"
  Bus Selector:RadarSensor:1_OBJ_ID_BS/57 -> RadarSensor:1.OBJ_ID_57/1  "<OBJ_ID_57>"
  Bus Selector:RadarSensor:1_OBJ_ID_BS/58 -> RadarSensor:1.OBJ_ID_58/1  "<OBJ_ID_58>"
  Bus Selector:RadarSensor:1_OBJ_ID_BS/59 -> RadarSensor:1.OBJ_ID_59/1  "<OBJ_ID_59>"
  Bus Selector:RadarSensor:1_OBJ_ID_BS/60 -> RadarSensor:1.OBJ_ID_60/1  "<OBJ_ID_60>"
  Bus Selector:RadarSensor:1_OBJ_ID_BS/61 -> RadarSensor:1.OBJ_ID_61/1  "<OBJ_ID_61>"
  Bus Selector:RadarSensor:1_OBJ_ID_BS/62 -> RadarSensor:1.OBJ_ID_62/1  "<OBJ_ID_62>"
  Bus Selector:RadarSensor:1_OBJ_ID_BS/63 -> RadarSensor:1.OBJ_ID_63/1  "<OBJ_ID_63>"
  Bus Selector:RadarSensor:1_OBJ_ID_BS/64 -> RadarSensor:1.OBJ_ID_64/1  "<OBJ_ID_64>"
  Bus Selector:RadarSensor:1_OBJ_Class_BS/1 -> RadarSensor:1.OBJ_Class_1/1  "<OBJ_Class_1>"
  Bus Selector:RadarSensor:1_OBJ_Class_BS/2 -> RadarSensor:1.OBJ_Class_2/1  "<OBJ_Class_2>"
  Bus Selector:RadarSensor:1_OBJ_Class_BS/3 -> RadarSensor:1.OBJ_Class_3/1  "<OBJ_Class_3>"
  Bus Selector:RadarSensor:1_OBJ_Class_BS/4 -> RadarSensor:1.OBJ_Class_4/1  "<OBJ_Class_4>"
  Bus Selector:RadarSensor:1_OBJ_Class_BS/5 -> RadarSensor:1.OBJ_Class_5/1  "<OBJ_Class_5>"
  Bus Selector:RadarSensor:1_OBJ_Class_BS/6 -> RadarSensor:1.OBJ_Class_6/1  "<OBJ_Class_6>"
  Bus Selector:RadarSensor:1_OBJ_Class_BS/7 -> RadarSensor:1.OBJ_Class_7/1  "<OBJ_Class_7>"
  Bus Selector:RadarSensor:1_OBJ_Class_BS/8 -> RadarSensor:1.OBJ_Class_8/1  "<OBJ_Class_8>"
  Bus Selector:RadarSensor:1_OBJ_Class_BS/9 -> RadarSensor:1.OBJ_Class_9/1  "<OBJ_Class_9>"
  Bus Selector:RadarSensor:1_OBJ_Class_BS/10 -> RadarSensor:1.OBJ_Class_10/1  "<OBJ_Class_10>"
  Bus Selector:RadarSensor:1_OBJ_Class_BS/11 -> RadarSensor:1.OBJ_Class_11/1  "<OBJ_Class_11>"
  Bus Selector:RadarSensor:1_OBJ_Class_BS/12 -> RadarSensor:1.OBJ_Class_12/1  "<OBJ_Class_12>"
  Bus Selector:RadarSensor:1_OBJ_Class_BS/13 -> RadarSensor:1.OBJ_Class_13/1  "<OBJ_Class_13>"
  Bus Selector:RadarSensor:1_OBJ_Class_BS/14 -> RadarSensor:1.OBJ_Class_14/1  "<OBJ_Class_14>"
  Bus Selector:RadarSensor:1_OBJ_Class_BS/15 -> RadarSensor:1.OBJ_Class_15/1  "<OBJ_Class_15>"
  Bus Selector:RadarSensor:1_OBJ_Class_BS/16 -> RadarSensor:1.OBJ_Class_16/1  "<OBJ_Class_16>"
  Bus Selector:RadarSensor:1_OBJ_Class_BS/17 -> RadarSensor:1.OBJ_Class_17/1  "<OBJ_Class_17>"
  Bus Selector:RadarSensor:1_OBJ_Class_BS/18 -> RadarSensor:1.OBJ_Class_18/1  "<OBJ_Class_18>"
  Bus Selector:RadarSensor:1_OBJ_Class_BS/19 -> RadarSensor:1.OBJ_Class_19/1  "<OBJ_Class_19>"
  Bus Selector:RadarSensor:1_OBJ_Class_BS/20 -> RadarSensor:1.OBJ_Class_20/1  "<OBJ_Class_20>"
  Bus Selector:RadarSensor:1_OBJ_Class_BS/21 -> RadarSensor:1.OBJ_Class_21/1  "<OBJ_Class_21>"
  Bus Selector:RadarSensor:1_OBJ_Class_BS/22 -> RadarSensor:1.OBJ_Class_22/1  "<OBJ_Class_22>"
  Bus Selector:RadarSensor:1_OBJ_Class_BS/23 -> RadarSensor:1.OBJ_Class_23/1  "<OBJ_Class_23>"
  Bus Selector:RadarSensor:1_OBJ_Class_BS/24 -> RadarSensor:1.OBJ_Class_24/1  "<OBJ_Class_24>"
  Bus Selector:RadarSensor:1_OBJ_Class_BS/25 -> RadarSensor:1.OBJ_Class_25/1  "<OBJ_Class_25>"
  Bus Selector:RadarSensor:1_OBJ_Class_BS/26 -> RadarSensor:1.OBJ_Class_26/1  "<OBJ_Class_26>"
  Bus Selector:RadarSensor:1_OBJ_Class_BS/27 -> RadarSensor:1.OBJ_Class_27/1  "<OBJ_Class_27>"
  Bus Selector:RadarSensor:1_OBJ_Class_BS/28 -> RadarSensor:1.OBJ_Class_28/1  "<OBJ_Class_28>"
  Bus Selector:RadarSensor:1_OBJ_Class_BS/29 -> RadarSensor:1.OBJ_Class_29/1  "<OBJ_Class_29>"
  Bus Selector:RadarSensor:1_OBJ_Class_BS/30 -> RadarSensor:1.OBJ_Class_30/1  "<OBJ_Class_30>"
  Bus Selector:RadarSensor:1_OBJ_Class_BS/31 -> RadarSensor:1.OBJ_Class_31/1  "<OBJ_Class_31>"
  Bus Selector:RadarSensor:1_OBJ_Class_BS/32 -> RadarSensor:1.OBJ_Class_32/1  "<OBJ_Class_32>"
  Bus Selector:RadarSensor:1_OBJ_Class_BS/33 -> RadarSensor:1.OBJ_Class_33/1  "<OBJ_Class_33>"
  Bus Selector:RadarSensor:1_OBJ_Class_BS/34 -> RadarSensor:1.OBJ_Class_34/1  "<OBJ_Class_34>"
  Bus Selector:RadarSensor:1_OBJ_Class_BS/35 -> RadarSensor:1.OBJ_Class_35/1  "<OBJ_Class_35>"
  Bus Selector:RadarSensor:1_OBJ_Class_BS/36 -> RadarSensor:1.OBJ_Class_36/1  "<OBJ_Class_36>"
  Bus Selector:RadarSensor:1_OBJ_Class_BS/37 -> RadarSensor:1.OBJ_Class_37/1  "<OBJ_Class_37>"
  Bus Selector:RadarSensor:1_OBJ_Class_BS/38 -> RadarSensor:1.OBJ_Class_38/1  "<OBJ_Class_38>"
  Bus Selector:RadarSensor:1_OBJ_Class_BS/39 -> RadarSensor:1.OBJ_Class_39/1  "<OBJ_Class_39>"
  Bus Selector:RadarSensor:1_OBJ_Class_BS/40 -> RadarSensor:1.OBJ_Class_40/1  "<OBJ_Class_40>"
  Bus Selector:RadarSensor:1_OBJ_Class_BS/41 -> RadarSensor:1.OBJ_Class_41/1  "<OBJ_Class_41>"
  Bus Selector:RadarSensor:1_OBJ_Class_BS/42 -> RadarSensor:1.OBJ_Class_42/1  "<OBJ_Class_42>"
  Bus Selector:RadarSensor:1_OBJ_Class_BS/43 -> RadarSensor:1.OBJ_Class_43/1  "<OBJ_Class_43>"
  Bus Selector:RadarSensor:1_OBJ_Class_BS/44 -> RadarSensor:1.OBJ_Class_44/1  "<OBJ_Class_44>"
  Bus Selector:RadarSensor:1_OBJ_Class_BS/45 -> RadarSensor:1.OBJ_Class_45/1  "<OBJ_Class_45>"
  Bus Selector:RadarSensor:1_OBJ_Class_BS/46 -> RadarSensor:1.OBJ_Class_46/1  "<OBJ_Class_46>"
  Bus Selector:RadarSensor:1_OBJ_Class_BS/47 -> RadarSensor:1.OBJ_Class_47/1  "<OBJ_Class_47>"
  Bus Selector:RadarSensor:1_OBJ_Class_BS/48 -> RadarSensor:1.OBJ_Class_48/1  "<OBJ_Class_48>"
  Bus Selector:RadarSensor:1_OBJ_Class_BS/49 -> RadarSensor:1.OBJ_Class_49/1  "<OBJ_Class_49>"
  Bus Selector:RadarSensor:1_OBJ_Class_BS/50 -> RadarSensor:1.OBJ_Class_50/1  "<OBJ_Class_50>"
  Bus Selector:RadarSensor:1_OBJ_Class_BS/51 -> RadarSensor:1.OBJ_Class_51/1  "<OBJ_Class_51>"
  Bus Selector:RadarSensor:1_OBJ_Class_BS/52 -> RadarSensor:1.OBJ_Class_52/1  "<OBJ_Class_52>"
  Bus Selector:RadarSensor:1_OBJ_Class_BS/53 -> RadarSensor:1.OBJ_Class_53/1  "<OBJ_Class_53>"
  Bus Selector:RadarSensor:1_OBJ_Class_BS/54 -> RadarSensor:1.OBJ_Class_54/1  "<OBJ_Class_54>"
  Bus Selector:RadarSensor:1_OBJ_Class_BS/55 -> RadarSensor:1.OBJ_Class_55/1  "<OBJ_Class_55>"
  Bus Selector:RadarSensor:1_OBJ_Class_BS/56 -> RadarSensor:1.OBJ_Class_56/1  "<OBJ_Class_56>"
  Bus Selector:RadarSensor:1_OBJ_Class_BS/57 -> RadarSensor:1.OBJ_Class_57/1  "<OBJ_Class_57>"
  Bus Selector:RadarSensor:1_OBJ_Class_BS/58 -> RadarSensor:1.OBJ_Class_58/1  "<OBJ_Class_58>"
  Bus Selector:RadarSensor:1_OBJ_Class_BS/59 -> RadarSensor:1.OBJ_Class_59/1  "<OBJ_Class_59>"
  Bus Selector:RadarSensor:1_OBJ_Class_BS/60 -> RadarSensor:1.OBJ_Class_60/1  "<OBJ_Class_60>"
  Bus Selector:RadarSensor:1_OBJ_Class_BS/61 -> RadarSensor:1.OBJ_Class_61/1  "<OBJ_Class_61>"
  Bus Selector:RadarSensor:1_OBJ_Class_BS/62 -> RadarSensor:1.OBJ_Class_62/1  "<OBJ_Class_62>"
  Bus Selector:RadarSensor:1_OBJ_Class_BS/63 -> RadarSensor:1.OBJ_Class_63/1  "<OBJ_Class_63>"
  Bus Selector:RadarSensor:1_OBJ_Class_BS/64 -> RadarSensor:1.OBJ_Class_64/1  "<OBJ_Class_64>"
  Bus Selector:RadarSensor:1_OBJ_S_Azimuth_BS/1 -> RadarSensor:1.OBJ_S_Azimuth_1/1  "<OBJ_S_Azimuth_1>"
  Bus Selector:RadarSensor:1_OBJ_S_Azimuth_BS/2 -> RadarSensor:1.OBJ_S_Azimuth_2/1  "<OBJ_S_Azimuth_2>"
  Bus Selector:RadarSensor:1_OBJ_S_Azimuth_BS/3 -> RadarSensor:1.OBJ_S_Azimuth_3/1  "<OBJ_S_Azimuth_3>"
  Bus Selector:RadarSensor:1_OBJ_S_Azimuth_BS/4 -> RadarSensor:1.OBJ_S_Azimuth_4/1  "<OBJ_S_Azimuth_4>"
  Bus Selector:RadarSensor:1_OBJ_S_Azimuth_BS/5 -> RadarSensor:1.OBJ_S_Azimuth_5/1  "<OBJ_S_Azimuth_5>"
  Bus Selector:RadarSensor:1_OBJ_S_Azimuth_BS/6 -> RadarSensor:1.OBJ_S_Azimuth_6/1  "<OBJ_S_Azimuth_6>"
  Bus Selector:RadarSensor:1_OBJ_S_Azimuth_BS/7 -> RadarSensor:1.OBJ_S_Azimuth_7/1  "<OBJ_S_Azimuth_7>"
  Bus Selector:RadarSensor:1_OBJ_S_Azimuth_BS/8 -> RadarSensor:1.OBJ_S_Azimuth_8/1  "<OBJ_S_Azimuth_8>"
  Bus Selector:RadarSensor:1_OBJ_S_Azimuth_BS/9 -> RadarSensor:1.OBJ_S_Azimuth_9/1  "<OBJ_S_Azimuth_9>"
  Bus Selector:RadarSensor:1_OBJ_S_Azimuth_BS/10 -> RadarSensor:1.OBJ_S_Azimuth_10/1  "<OBJ_S_Azimuth_10>"
  Bus Selector:RadarSensor:1_OBJ_S_Azimuth_BS/11 -> RadarSensor:1.OBJ_S_Azimuth_11/1  "<OBJ_S_Azimuth_11>"
  Bus Selector:RadarSensor:1_OBJ_S_Azimuth_BS/12 -> RadarSensor:1.OBJ_S_Azimuth_12/1  "<OBJ_S_Azimuth_12>"
  Bus Selector:RadarSensor:1_OBJ_S_Azimuth_BS/13 -> RadarSensor:1.OBJ_S_Azimuth_13/1  "<OBJ_S_Azimuth_13>"
  Bus Selector:RadarSensor:1_OBJ_S_Azimuth_BS/14 -> RadarSensor:1.OBJ_S_Azimuth_14/1  "<OBJ_S_Azimuth_14>"
  Bus Selector:RadarSensor:1_OBJ_S_Azimuth_BS/15 -> RadarSensor:1.OBJ_S_Azimuth_15/1  "<OBJ_S_Azimuth_15>"
  Bus Selector:RadarSensor:1_OBJ_S_Azimuth_BS/16 -> RadarSensor:1.OBJ_S_Azimuth_16/1  "<OBJ_S_Azimuth_16>"
  Bus Selector:RadarSensor:1_OBJ_S_Azimuth_BS/17 -> RadarSensor:1.OBJ_S_Azimuth_17/1  "<OBJ_S_Azimuth_17>"
  Bus Selector:RadarSensor:1_OBJ_S_Azimuth_BS/18 -> RadarSensor:1.OBJ_S_Azimuth_18/1  "<OBJ_S_Azimuth_18>"
  Bus Selector:RadarSensor:1_OBJ_S_Azimuth_BS/19 -> RadarSensor:1.OBJ_S_Azimuth_19/1  "<OBJ_S_Azimuth_19>"
  Bus Selector:RadarSensor:1_OBJ_S_Azimuth_BS/20 -> RadarSensor:1.OBJ_S_Azimuth_20/1  "<OBJ_S_Azimuth_20>"
  Bus Selector:RadarSensor:1_OBJ_S_Azimuth_BS/21 -> RadarSensor:1.OBJ_S_Azimuth_21/1  "<OBJ_S_Azimuth_21>"
  Bus Selector:RadarSensor:1_OBJ_S_Azimuth_BS/22 -> RadarSensor:1.OBJ_S_Azimuth_22/1  "<OBJ_S_Azimuth_22>"
  Bus Selector:RadarSensor:1_OBJ_S_Azimuth_BS/23 -> RadarSensor:1.OBJ_S_Azimuth_23/1  "<OBJ_S_Azimuth_23>"
  Bus Selector:RadarSensor:1_OBJ_S_Azimuth_BS/24 -> RadarSensor:1.OBJ_S_Azimuth_24/1  "<OBJ_S_Azimuth_24>"
  Bus Selector:RadarSensor:1_OBJ_S_Azimuth_BS/25 -> RadarSensor:1.OBJ_S_Azimuth_25/1  "<OBJ_S_Azimuth_25>"
  Bus Selector:RadarSensor:1_OBJ_S_Azimuth_BS/26 -> RadarSensor:1.OBJ_S_Azimuth_26/1  "<OBJ_S_Azimuth_26>"
  Bus Selector:RadarSensor:1_OBJ_S_Azimuth_BS/27 -> RadarSensor:1.OBJ_S_Azimuth_27/1  "<OBJ_S_Azimuth_27>"
  Bus Selector:RadarSensor:1_OBJ_S_Azimuth_BS/28 -> RadarSensor:1.OBJ_S_Azimuth_28/1  "<OBJ_S_Azimuth_28>"
  Bus Selector:RadarSensor:1_OBJ_S_Azimuth_BS/29 -> RadarSensor:1.OBJ_S_Azimuth_29/1  "<OBJ_S_Azimuth_29>"
  Bus Selector:RadarSensor:1_OBJ_S_Azimuth_BS/30 -> RadarSensor:1.OBJ_S_Azimuth_30/1  "<OBJ_S_Azimuth_30>"
  Bus Selector:RadarSensor:1_OBJ_S_Azimuth_BS/31 -> RadarSensor:1.OBJ_S_Azimuth_31/1  "<OBJ_S_Azimuth_31>"
  Bus Selector:RadarSensor:1_OBJ_S_Azimuth_BS/32 -> RadarSensor:1.OBJ_S_Azimuth_32/1  "<OBJ_S_Azimuth_32>"
  Bus Selector:RadarSensor:1_OBJ_S_Azimuth_BS/33 -> RadarSensor:1.OBJ_S_Azimuth_33/1  "<OBJ_S_Azimuth_33>"
  Bus Selector:RadarSensor:1_OBJ_S_Azimuth_BS/34 -> RadarSensor:1.OBJ_S_Azimuth_34/1  "<OBJ_S_Azimuth_34>"
  Bus Selector:RadarSensor:1_OBJ_S_Azimuth_BS/35 -> RadarSensor:1.OBJ_S_Azimuth_35/1  "<OBJ_S_Azimuth_35>"
  Bus Selector:RadarSensor:1_OBJ_S_Azimuth_BS/36 -> RadarSensor:1.OBJ_S_Azimuth_36/1  "<OBJ_S_Azimuth_36>"
  Bus Selector:RadarSensor:1_OBJ_S_Azimuth_BS/37 -> RadarSensor:1.OBJ_S_Azimuth_37/1  "<OBJ_S_Azimuth_37>"
  Bus Selector:RadarSensor:1_OBJ_S_Azimuth_BS/38 -> RadarSensor:1.OBJ_S_Azimuth_38/1  "<OBJ_S_Azimuth_38>"
  Bus Selector:RadarSensor:1_OBJ_S_Azimuth_BS/39 -> RadarSensor:1.OBJ_S_Azimuth_39/1  "<OBJ_S_Azimuth_39>"
  Bus Selector:RadarSensor:1_OBJ_S_Azimuth_BS/40 -> RadarSensor:1.OBJ_S_Azimuth_40/1  "<OBJ_S_Azimuth_40>"
  Bus Selector:RadarSensor:1_OBJ_S_Azimuth_BS/41 -> RadarSensor:1.OBJ_S_Azimuth_41/1  "<OBJ_S_Azimuth_41>"
  Bus Selector:RadarSensor:1_OBJ_S_Azimuth_BS/42 -> RadarSensor:1.OBJ_S_Azimuth_42/1  "<OBJ_S_Azimuth_42>"
  Bus Selector:RadarSensor:1_OBJ_S_Azimuth_BS/43 -> RadarSensor:1.OBJ_S_Azimuth_43/1  "<OBJ_S_Azimuth_43>"
  Bus Selector:RadarSensor:1_OBJ_S_Azimuth_BS/44 -> RadarSensor:1.OBJ_S_Azimuth_44/1  "<OBJ_S_Azimuth_44>"
  Bus Selector:RadarSensor:1_OBJ_S_Azimuth_BS/45 -> RadarSensor:1.OBJ_S_Azimuth_45/1  "<OBJ_S_Azimuth_45>"
  Bus Selector:RadarSensor:1_OBJ_S_Azimuth_BS/46 -> RadarSensor:1.OBJ_S_Azimuth_46/1  "<OBJ_S_Azimuth_46>"
  Bus Selector:RadarSensor:1_OBJ_S_Azimuth_BS/47 -> RadarSensor:1.OBJ_S_Azimuth_47/1  "<OBJ_S_Azimuth_47>"
  Bus Selector:RadarSensor:1_OBJ_S_Azimuth_BS/48 -> RadarSensor:1.OBJ_S_Azimuth_48/1  "<OBJ_S_Azimuth_48>"
  Bus Selector:RadarSensor:1_OBJ_S_Azimuth_BS/49 -> RadarSensor:1.OBJ_S_Azimuth_49/1  "<OBJ_S_Azimuth_49>"
  Bus Selector:RadarSensor:1_OBJ_S_Azimuth_BS/50 -> RadarSensor:1.OBJ_S_Azimuth_50/1  "<OBJ_S_Azimuth_50>"
  Bus Selector:RadarSensor:1_OBJ_S_Azimuth_BS/51 -> RadarSensor:1.OBJ_S_Azimuth_51/1  "<OBJ_S_Azimuth_51>"
  Bus Selector:RadarSensor:1_OBJ_S_Azimuth_BS/52 -> RadarSensor:1.OBJ_S_Azimuth_52/1  "<OBJ_S_Azimuth_52>"
  Bus Selector:RadarSensor:1_OBJ_S_Azimuth_BS/53 -> RadarSensor:1.OBJ_S_Azimuth_53/1  "<OBJ_S_Azimuth_53>"
  Bus Selector:RadarSensor:1_OBJ_S_Azimuth_BS/54 -> RadarSensor:1.OBJ_S_Azimuth_54/1  "<OBJ_S_Azimuth_54>"
  Bus Selector:RadarSensor:1_OBJ_S_Azimuth_BS/55 -> RadarSensor:1.OBJ_S_Azimuth_55/1  "<OBJ_S_Azimuth_55>"
  Bus Selector:RadarSensor:1_OBJ_S_Azimuth_BS/56 -> RadarSensor:1.OBJ_S_Azimuth_56/1  "<OBJ_S_Azimuth_56>"
  Bus Selector:RadarSensor:1_OBJ_S_Azimuth_BS/57 -> RadarSensor:1.OBJ_S_Azimuth_57/1  "<OBJ_S_Azimuth_57>"
  Bus Selector:RadarSensor:1_OBJ_S_Azimuth_BS/58 -> RadarSensor:1.OBJ_S_Azimuth_58/1  "<OBJ_S_Azimuth_58>"
  Bus Selector:RadarSensor:1_OBJ_S_Azimuth_BS/59 -> RadarSensor:1.OBJ_S_Azimuth_59/1  "<OBJ_S_Azimuth_59>"
  Bus Selector:RadarSensor:1_OBJ_S_Azimuth_BS/60 -> RadarSensor:1.OBJ_S_Azimuth_60/1  "<OBJ_S_Azimuth_60>"
  Bus Selector:RadarSensor:1_OBJ_S_Azimuth_BS/61 -> RadarSensor:1.OBJ_S_Azimuth_61/1  "<OBJ_S_Azimuth_61>"
  Bus Selector:RadarSensor:1_OBJ_S_Azimuth_BS/62 -> RadarSensor:1.OBJ_S_Azimuth_62/1  "<OBJ_S_Azimuth_62>"
  Bus Selector:RadarSensor:1_OBJ_S_Azimuth_BS/63 -> RadarSensor:1.OBJ_S_Azimuth_63/1  "<OBJ_S_Azimuth_63>"
  Bus Selector:RadarSensor:1_OBJ_S_Azimuth_BS/64 -> RadarSensor:1.OBJ_S_Azimuth_64/1  "<OBJ_S_Azimuth_64>"
  Bus Selector:RadarSensor:1_OBJ_S_Elevation_BS/1 -> RadarSensor:1.OBJ_S_Elevation_1/1  "<OBJ_S_Elevation_1>"
  Bus Selector:RadarSensor:1_OBJ_S_Elevation_BS/2 -> RadarSensor:1.OBJ_S_Elevation_2/1  "<OBJ_S_Elevation_2>"
  Bus Selector:RadarSensor:1_OBJ_S_Elevation_BS/3 -> RadarSensor:1.OBJ_S_Elevation_3/1  "<OBJ_S_Elevation_3>"
  Bus Selector:RadarSensor:1_OBJ_S_Elevation_BS/4 -> RadarSensor:1.OBJ_S_Elevation_4/1  "<OBJ_S_Elevation_4>"
  Bus Selector:RadarSensor:1_OBJ_S_Elevation_BS/5 -> RadarSensor:1.OBJ_S_Elevation_5/1  "<OBJ_S_Elevation_5>"
  Bus Selector:RadarSensor:1_OBJ_S_Elevation_BS/6 -> RadarSensor:1.OBJ_S_Elevation_6/1  "<OBJ_S_Elevation_6>"
  Bus Selector:RadarSensor:1_OBJ_S_Elevation_BS/7 -> RadarSensor:1.OBJ_S_Elevation_7/1  "<OBJ_S_Elevation_7>"
  Bus Selector:RadarSensor:1_OBJ_S_Elevation_BS/8 -> RadarSensor:1.OBJ_S_Elevation_8/1  "<OBJ_S_Elevation_8>"
  Bus Selector:RadarSensor:1_OBJ_S_Elevation_BS/9 -> RadarSensor:1.OBJ_S_Elevation_9/1  "<OBJ_S_Elevation_9>"
  Bus Selector:RadarSensor:1_OBJ_S_Elevation_BS/10 -> RadarSensor:1.OBJ_S_Elevation_10/1  "<OBJ_S_Elevation_10>"
  Bus Selector:RadarSensor:1_OBJ_S_Elevation_BS/11 -> RadarSensor:1.OBJ_S_Elevation_11/1  "<OBJ_S_Elevation_11>"
  Bus Selector:RadarSensor:1_OBJ_S_Elevation_BS/12 -> RadarSensor:1.OBJ_S_Elevation_12/1  "<OBJ_S_Elevation_12>"
  Bus Selector:RadarSensor:1_OBJ_S_Elevation_BS/13 -> RadarSensor:1.OBJ_S_Elevation_13/1  "<OBJ_S_Elevation_13>"
  Bus Selector:RadarSensor:1_OBJ_S_Elevation_BS/14 -> RadarSensor:1.OBJ_S_Elevation_14/1  "<OBJ_S_Elevation_14>"
  Bus Selector:RadarSensor:1_OBJ_S_Elevation_BS/15 -> RadarSensor:1.OBJ_S_Elevation_15/1  "<OBJ_S_Elevation_15>"
  Bus Selector:RadarSensor:1_OBJ_S_Elevation_BS/16 -> RadarSensor:1.OBJ_S_Elevation_16/1  "<OBJ_S_Elevation_16>"
  Bus Selector:RadarSensor:1_OBJ_S_Elevation_BS/17 -> RadarSensor:1.OBJ_S_Elevation_17/1  "<OBJ_S_Elevation_17>"
  Bus Selector:RadarSensor:1_OBJ_S_Elevation_BS/18 -> RadarSensor:1.OBJ_S_Elevation_18/1  "<OBJ_S_Elevation_18>"
  Bus Selector:RadarSensor:1_OBJ_S_Elevation_BS/19 -> RadarSensor:1.OBJ_S_Elevation_19/1  "<OBJ_S_Elevation_19>"
  Bus Selector:RadarSensor:1_OBJ_S_Elevation_BS/20 -> RadarSensor:1.OBJ_S_Elevation_20/1  "<OBJ_S_Elevation_20>"
  Bus Selector:RadarSensor:1_OBJ_S_Elevation_BS/21 -> RadarSensor:1.OBJ_S_Elevation_21/1  "<OBJ_S_Elevation_21>"
  Bus Selector:RadarSensor:1_OBJ_S_Elevation_BS/22 -> RadarSensor:1.OBJ_S_Elevation_22/1  "<OBJ_S_Elevation_22>"
  Bus Selector:RadarSensor:1_OBJ_S_Elevation_BS/23 -> RadarSensor:1.OBJ_S_Elevation_23/1  "<OBJ_S_Elevation_23>"
  Bus Selector:RadarSensor:1_OBJ_S_Elevation_BS/24 -> RadarSensor:1.OBJ_S_Elevation_24/1  "<OBJ_S_Elevation_24>"
  Bus Selector:RadarSensor:1_OBJ_S_Elevation_BS/25 -> RadarSensor:1.OBJ_S_Elevation_25/1  "<OBJ_S_Elevation_25>"
  Bus Selector:RadarSensor:1_OBJ_S_Elevation_BS/26 -> RadarSensor:1.OBJ_S_Elevation_26/1  "<OBJ_S_Elevation_26>"
  Bus Selector:RadarSensor:1_OBJ_S_Elevation_BS/27 -> RadarSensor:1.OBJ_S_Elevation_27/1  "<OBJ_S_Elevation_27>"
  Bus Selector:RadarSensor:1_OBJ_S_Elevation_BS/28 -> RadarSensor:1.OBJ_S_Elevation_28/1  "<OBJ_S_Elevation_28>"
  Bus Selector:RadarSensor:1_OBJ_S_Elevation_BS/29 -> RadarSensor:1.OBJ_S_Elevation_29/1  "<OBJ_S_Elevation_29>"
  Bus Selector:RadarSensor:1_OBJ_S_Elevation_BS/30 -> RadarSensor:1.OBJ_S_Elevation_30/1  "<OBJ_S_Elevation_30>"
  Bus Selector:RadarSensor:1_OBJ_S_Elevation_BS/31 -> RadarSensor:1.OBJ_S_Elevation_31/1  "<OBJ_S_Elevation_31>"
  Bus Selector:RadarSensor:1_OBJ_S_Elevation_BS/32 -> RadarSensor:1.OBJ_S_Elevation_32/1  "<OBJ_S_Elevation_32>"
  Bus Selector:RadarSensor:1_OBJ_S_Elevation_BS/33 -> RadarSensor:1.OBJ_S_Elevation_33/1  "<OBJ_S_Elevation_33>"
  Bus Selector:RadarSensor:1_OBJ_S_Elevation_BS/34 -> RadarSensor:1.OBJ_S_Elevation_34/1  "<OBJ_S_Elevation_34>"
  Bus Selector:RadarSensor:1_OBJ_S_Elevation_BS/35 -> RadarSensor:1.OBJ_S_Elevation_35/1  "<OBJ_S_Elevation_35>"
  Bus Selector:RadarSensor:1_OBJ_S_Elevation_BS/36 -> RadarSensor:1.OBJ_S_Elevation_36/1  "<OBJ_S_Elevation_36>"
  Bus Selector:RadarSensor:1_OBJ_S_Elevation_BS/37 -> RadarSensor:1.OBJ_S_Elevation_37/1  "<OBJ_S_Elevation_37>"
  Bus Selector:RadarSensor:1_OBJ_S_Elevation_BS/38 -> RadarSensor:1.OBJ_S_Elevation_38/1  "<OBJ_S_Elevation_38>"
  Bus Selector:RadarSensor:1_OBJ_S_Elevation_BS/39 -> RadarSensor:1.OBJ_S_Elevation_39/1  "<OBJ_S_Elevation_39>"
  Bus Selector:RadarSensor:1_OBJ_S_Elevation_BS/40 -> RadarSensor:1.OBJ_S_Elevation_40/1  "<OBJ_S_Elevation_40>"
  Bus Selector:RadarSensor:1_OBJ_S_Elevation_BS/41 -> RadarSensor:1.OBJ_S_Elevation_41/1  "<OBJ_S_Elevation_41>"
  Bus Selector:RadarSensor:1_OBJ_S_Elevation_BS/42 -> RadarSensor:1.OBJ_S_Elevation_42/1  "<OBJ_S_Elevation_42>"
  Bus Selector:RadarSensor:1_OBJ_S_Elevation_BS/43 -> RadarSensor:1.OBJ_S_Elevation_43/1  "<OBJ_S_Elevation_43>"
  Bus Selector:RadarSensor:1_OBJ_S_Elevation_BS/44 -> RadarSensor:1.OBJ_S_Elevation_44/1  "<OBJ_S_Elevation_44>"
  Bus Selector:RadarSensor:1_OBJ_S_Elevation_BS/45 -> RadarSensor:1.OBJ_S_Elevation_45/1  "<OBJ_S_Elevation_45>"
  Bus Selector:RadarSensor:1_OBJ_S_Elevation_BS/46 -> RadarSensor:1.OBJ_S_Elevation_46/1  "<OBJ_S_Elevation_46>"
  Bus Selector:RadarSensor:1_OBJ_S_Elevation_BS/47 -> RadarSensor:1.OBJ_S_Elevation_47/1  "<OBJ_S_Elevation_47>"
  Bus Selector:RadarSensor:1_OBJ_S_Elevation_BS/48 -> RadarSensor:1.OBJ_S_Elevation_48/1  "<OBJ_S_Elevation_48>"
  Bus Selector:RadarSensor:1_OBJ_S_Elevation_BS/49 -> RadarSensor:1.OBJ_S_Elevation_49/1  "<OBJ_S_Elevation_49>"
  Bus Selector:RadarSensor:1_OBJ_S_Elevation_BS/50 -> RadarSensor:1.OBJ_S_Elevation_50/1  "<OBJ_S_Elevation_50>"
  Bus Selector:RadarSensor:1_OBJ_S_Elevation_BS/51 -> RadarSensor:1.OBJ_S_Elevation_51/1  "<OBJ_S_Elevation_51>"
  Bus Selector:RadarSensor:1_OBJ_S_Elevation_BS/52 -> RadarSensor:1.OBJ_S_Elevation_52/1  "<OBJ_S_Elevation_52>"
  Bus Selector:RadarSensor:1_OBJ_S_Elevation_BS/53 -> RadarSensor:1.OBJ_S_Elevation_53/1  "<OBJ_S_Elevation_53>"
  Bus Selector:RadarSensor:1_OBJ_S_Elevation_BS/54 -> RadarSensor:1.OBJ_S_Elevation_54/1  "<OBJ_S_Elevation_54>"
  Bus Selector:RadarSensor:1_OBJ_S_Elevation_BS/55 -> RadarSensor:1.OBJ_S_Elevation_55/1  "<OBJ_S_Elevation_55>"
  Bus Selector:RadarSensor:1_OBJ_S_Elevation_BS/56 -> RadarSensor:1.OBJ_S_Elevation_56/1  "<OBJ_S_Elevation_56>"
  Bus Selector:RadarSensor:1_OBJ_S_Elevation_BS/57 -> RadarSensor:1.OBJ_S_Elevation_57/1  "<OBJ_S_Elevation_57>"
  Bus Selector:RadarSensor:1_OBJ_S_Elevation_BS/58 -> RadarSensor:1.OBJ_S_Elevation_58/1  "<OBJ_S_Elevation_58>"
  Bus Selector:RadarSensor:1_OBJ_S_Elevation_BS/59 -> RadarSensor:1.OBJ_S_Elevation_59/1  "<OBJ_S_Elevation_59>"
  Bus Selector:RadarSensor:1_OBJ_S_Elevation_BS/60 -> RadarSensor:1.OBJ_S_Elevation_60/1  "<OBJ_S_Elevation_60>"
  Bus Selector:RadarSensor:1_OBJ_S_Elevation_BS/61 -> RadarSensor:1.OBJ_S_Elevation_61/1  "<OBJ_S_Elevation_61>"
  Bus Selector:RadarSensor:1_OBJ_S_Elevation_BS/62 -> RadarSensor:1.OBJ_S_Elevation_62/1  "<OBJ_S_Elevation_62>"
  Bus Selector:RadarSensor:1_OBJ_S_Elevation_BS/63 -> RadarSensor:1.OBJ_S_Elevation_63/1  "<OBJ_S_Elevation_63>"
  Bus Selector:RadarSensor:1_OBJ_S_Elevation_BS/64 -> RadarSensor:1.OBJ_S_Elevation_64/1  "<OBJ_S_Elevation_64>"
  Bus Selector:RadarSensor:1_OBJ_S_Velocity_BS/1 -> RadarSensor:1.OBJ_S_Velocity_1/1  "<OBJ_S_Velocity_1>"
  Bus Selector:RadarSensor:1_OBJ_S_Velocity_BS/2 -> RadarSensor:1.OBJ_S_Velocity_2/1  "<OBJ_S_Velocity_2>"
  Bus Selector:RadarSensor:1_OBJ_S_Velocity_BS/3 -> RadarSensor:1.OBJ_S_Velocity_3/1  "<OBJ_S_Velocity_3>"
  Bus Selector:RadarSensor:1_OBJ_S_Velocity_BS/4 -> RadarSensor:1.OBJ_S_Velocity_4/1  "<OBJ_S_Velocity_4>"
  Bus Selector:RadarSensor:1_OBJ_S_Velocity_BS/5 -> RadarSensor:1.OBJ_S_Velocity_5/1  "<OBJ_S_Velocity_5>"
  Bus Selector:RadarSensor:1_OBJ_S_Velocity_BS/6 -> RadarSensor:1.OBJ_S_Velocity_6/1  "<OBJ_S_Velocity_6>"
  Bus Selector:RadarSensor:1_OBJ_S_Velocity_BS/7 -> RadarSensor:1.OBJ_S_Velocity_7/1  "<OBJ_S_Velocity_7>"
  Bus Selector:RadarSensor:1_OBJ_S_Velocity_BS/8 -> RadarSensor:1.OBJ_S_Velocity_8/1  "<OBJ_S_Velocity_8>"
  Bus Selector:RadarSensor:1_OBJ_S_Velocity_BS/9 -> RadarSensor:1.OBJ_S_Velocity_9/1  "<OBJ_S_Velocity_9>"
  Bus Selector:RadarSensor:1_OBJ_S_Velocity_BS/10 -> RadarSensor:1.OBJ_S_Velocity_10/1  "<OBJ_S_Velocity_10>"
  Bus Selector:RadarSensor:1_OBJ_S_Velocity_BS/11 -> RadarSensor:1.OBJ_S_Velocity_11/1  "<OBJ_S_Velocity_11>"
  Bus Selector:RadarSensor:1_OBJ_S_Velocity_BS/12 -> RadarSensor:1.OBJ_S_Velocity_12/1  "<OBJ_S_Velocity_12>"
  Bus Selector:RadarSensor:1_OBJ_S_Velocity_BS/13 -> RadarSensor:1.OBJ_S_Velocity_13/1  "<OBJ_S_Velocity_13>"
  Bus Selector:RadarSensor:1_OBJ_S_Velocity_BS/14 -> RadarSensor:1.OBJ_S_Velocity_14/1  "<OBJ_S_Velocity_14>"
  Bus Selector:RadarSensor:1_OBJ_S_Velocity_BS/15 -> RadarSensor:1.OBJ_S_Velocity_15/1  "<OBJ_S_Velocity_15>"
  Bus Selector:RadarSensor:1_OBJ_S_Velocity_BS/16 -> RadarSensor:1.OBJ_S_Velocity_16/1  "<OBJ_S_Velocity_16>"
  Bus Selector:RadarSensor:1_OBJ_S_Velocity_BS/17 -> RadarSensor:1.OBJ_S_Velocity_17/1  "<OBJ_S_Velocity_17>"
  Bus Selector:RadarSensor:1_OBJ_S_Velocity_BS/18 -> RadarSensor:1.OBJ_S_Velocity_18/1  "<OBJ_S_Velocity_18>"
  Bus Selector:RadarSensor:1_OBJ_S_Velocity_BS/19 -> RadarSensor:1.OBJ_S_Velocity_19/1  "<OBJ_S_Velocity_19>"
  Bus Selector:RadarSensor:1_OBJ_S_Velocity_BS/20 -> RadarSensor:1.OBJ_S_Velocity_20/1  "<OBJ_S_Velocity_20>"
  Bus Selector:RadarSensor:1_OBJ_S_Velocity_BS/21 -> RadarSensor:1.OBJ_S_Velocity_21/1  "<OBJ_S_Velocity_21>"
  Bus Selector:RadarSensor:1_OBJ_S_Velocity_BS/22 -> RadarSensor:1.OBJ_S_Velocity_22/1  "<OBJ_S_Velocity_22>"
  Bus Selector:RadarSensor:1_OBJ_S_Velocity_BS/23 -> RadarSensor:1.OBJ_S_Velocity_23/1  "<OBJ_S_Velocity_23>"
  Bus Selector:RadarSensor:1_OBJ_S_Velocity_BS/24 -> RadarSensor:1.OBJ_S_Velocity_24/1  "<OBJ_S_Velocity_24>"
  Bus Selector:RadarSensor:1_OBJ_S_Velocity_BS/25 -> RadarSensor:1.OBJ_S_Velocity_25/1  "<OBJ_S_Velocity_25>"
  Bus Selector:RadarSensor:1_OBJ_S_Velocity_BS/26 -> RadarSensor:1.OBJ_S_Velocity_26/1  "<OBJ_S_Velocity_26>"
  Bus Selector:RadarSensor:1_OBJ_S_Velocity_BS/27 -> RadarSensor:1.OBJ_S_Velocity_27/1  "<OBJ_S_Velocity_27>"
  Bus Selector:RadarSensor:1_OBJ_S_Velocity_BS/28 -> RadarSensor:1.OBJ_S_Velocity_28/1  "<OBJ_S_Velocity_28>"
  Bus Selector:RadarSensor:1_OBJ_S_Velocity_BS/29 -> RadarSensor:1.OBJ_S_Velocity_29/1  "<OBJ_S_Velocity_29>"
  Bus Selector:RadarSensor:1_OBJ_S_Velocity_BS/30 -> RadarSensor:1.OBJ_S_Velocity_30/1  "<OBJ_S_Velocity_30>"
  Bus Selector:RadarSensor:1_OBJ_S_Velocity_BS/31 -> RadarSensor:1.OBJ_S_Velocity_31/1  "<OBJ_S_Velocity_31>"
  Bus Selector:RadarSensor:1_OBJ_S_Velocity_BS/32 -> RadarSensor:1.OBJ_S_Velocity_32/1  "<OBJ_S_Velocity_32>"
  Bus Selector:RadarSensor:1_OBJ_S_Velocity_BS/33 -> RadarSensor:1.OBJ_S_Velocity_33/1  "<OBJ_S_Velocity_33>"
  Bus Selector:RadarSensor:1_OBJ_S_Velocity_BS/34 -> RadarSensor:1.OBJ_S_Velocity_34/1  "<OBJ_S_Velocity_34>"
  Bus Selector:RadarSensor:1_OBJ_S_Velocity_BS/35 -> RadarSensor:1.OBJ_S_Velocity_35/1  "<OBJ_S_Velocity_35>"
  Bus Selector:RadarSensor:1_OBJ_S_Velocity_BS/36 -> RadarSensor:1.OBJ_S_Velocity_36/1  "<OBJ_S_Velocity_36>"
  Bus Selector:RadarSensor:1_OBJ_S_Velocity_BS/37 -> RadarSensor:1.OBJ_S_Velocity_37/1  "<OBJ_S_Velocity_37>"
  Bus Selector:RadarSensor:1_OBJ_S_Velocity_BS/38 -> RadarSensor:1.OBJ_S_Velocity_38/1  "<OBJ_S_Velocity_38>"
  Bus Selector:RadarSensor:1_OBJ_S_Velocity_BS/39 -> RadarSensor:1.OBJ_S_Velocity_39/1  "<OBJ_S_Velocity_39>"
  Bus Selector:RadarSensor:1_OBJ_S_Velocity_BS/40 -> RadarSensor:1.OBJ_S_Velocity_40/1  "<OBJ_S_Velocity_40>"
  Bus Selector:RadarSensor:1_OBJ_S_Velocity_BS/41 -> RadarSensor:1.OBJ_S_Velocity_41/1  "<OBJ_S_Velocity_41>"
  Bus Selector:RadarSensor:1_OBJ_S_Velocity_BS/42 -> RadarSensor:1.OBJ_S_Velocity_42/1  "<OBJ_S_Velocity_42>"
  Bus Selector:RadarSensor:1_OBJ_S_Velocity_BS/43 -> RadarSensor:1.OBJ_S_Velocity_43/1  "<OBJ_S_Velocity_43>"
  Bus Selector:RadarSensor:1_OBJ_S_Velocity_BS/44 -> RadarSensor:1.OBJ_S_Velocity_44/1  "<OBJ_S_Velocity_44>"
  Bus Selector:RadarSensor:1_OBJ_S_Velocity_BS/45 -> RadarSensor:1.OBJ_S_Velocity_45/1  "<OBJ_S_Velocity_45>"
  Bus Selector:RadarSensor:1_OBJ_S_Velocity_BS/46 -> RadarSensor:1.OBJ_S_Velocity_46/1  "<OBJ_S_Velocity_46>"
  Bus Selector:RadarSensor:1_OBJ_S_Velocity_BS/47 -> RadarSensor:1.OBJ_S_Velocity_47/1  "<OBJ_S_Velocity_47>"
  Bus Selector:RadarSensor:1_OBJ_S_Velocity_BS/48 -> RadarSensor:1.OBJ_S_Velocity_48/1  "<OBJ_S_Velocity_48>"
  Bus Selector:RadarSensor:1_OBJ_S_Velocity_BS/49 -> RadarSensor:1.OBJ_S_Velocity_49/1  "<OBJ_S_Velocity_49>"
  Bus Selector:RadarSensor:1_OBJ_S_Velocity_BS/50 -> RadarSensor:1.OBJ_S_Velocity_50/1  "<OBJ_S_Velocity_50>"
  Bus Selector:RadarSensor:1_OBJ_S_Velocity_BS/51 -> RadarSensor:1.OBJ_S_Velocity_51/1  "<OBJ_S_Velocity_51>"
  Bus Selector:RadarSensor:1_OBJ_S_Velocity_BS/52 -> RadarSensor:1.OBJ_S_Velocity_52/1  "<OBJ_S_Velocity_52>"
  Bus Selector:RadarSensor:1_OBJ_S_Velocity_BS/53 -> RadarSensor:1.OBJ_S_Velocity_53/1  "<OBJ_S_Velocity_53>"
  Bus Selector:RadarSensor:1_OBJ_S_Velocity_BS/54 -> RadarSensor:1.OBJ_S_Velocity_54/1  "<OBJ_S_Velocity_54>"
  Bus Selector:RadarSensor:1_OBJ_S_Velocity_BS/55 -> RadarSensor:1.OBJ_S_Velocity_55/1  "<OBJ_S_Velocity_55>"
  Bus Selector:RadarSensor:1_OBJ_S_Velocity_BS/56 -> RadarSensor:1.OBJ_S_Velocity_56/1  "<OBJ_S_Velocity_56>"
  Bus Selector:RadarSensor:1_OBJ_S_Velocity_BS/57 -> RadarSensor:1.OBJ_S_Velocity_57/1  "<OBJ_S_Velocity_57>"
  Bus Selector:RadarSensor:1_OBJ_S_Velocity_BS/58 -> RadarSensor:1.OBJ_S_Velocity_58/1  "<OBJ_S_Velocity_58>"
  Bus Selector:RadarSensor:1_OBJ_S_Velocity_BS/59 -> RadarSensor:1.OBJ_S_Velocity_59/1  "<OBJ_S_Velocity_59>"
  Bus Selector:RadarSensor:1_OBJ_S_Velocity_BS/60 -> RadarSensor:1.OBJ_S_Velocity_60/1  "<OBJ_S_Velocity_60>"
  Bus Selector:RadarSensor:1_OBJ_S_Velocity_BS/61 -> RadarSensor:1.OBJ_S_Velocity_61/1  "<OBJ_S_Velocity_61>"
  Bus Selector:RadarSensor:1_OBJ_S_Velocity_BS/62 -> RadarSensor:1.OBJ_S_Velocity_62/1  "<OBJ_S_Velocity_62>"
  Bus Selector:RadarSensor:1_OBJ_S_Velocity_BS/63 -> RadarSensor:1.OBJ_S_Velocity_63/1  "<OBJ_S_Velocity_63>"
  Bus Selector:RadarSensor:1_OBJ_S_Velocity_BS/64 -> RadarSensor:1.OBJ_S_Velocity_64/1  "<OBJ_S_Velocity_64>"
  Bus Selector:RadarSensor:1_OBJ_S_Range_BS/1 -> RadarSensor:1.OBJ_S_Range_1/1  "<OBJ_S_Range_1>"
  Bus Selector:RadarSensor:1_OBJ_S_Range_BS/2 -> RadarSensor:1.OBJ_S_Range_2/1  "<OBJ_S_Range_2>"
  Bus Selector:RadarSensor:1_OBJ_S_Range_BS/3 -> RadarSensor:1.OBJ_S_Range_3/1  "<OBJ_S_Range_3>"
  Bus Selector:RadarSensor:1_OBJ_S_Range_BS/4 -> RadarSensor:1.OBJ_S_Range_4/1  "<OBJ_S_Range_4>"
  Bus Selector:RadarSensor:1_OBJ_S_Range_BS/5 -> RadarSensor:1.OBJ_S_Range_5/1  "<OBJ_S_Range_5>"
  Bus Selector:RadarSensor:1_OBJ_S_Range_BS/6 -> RadarSensor:1.OBJ_S_Range_6/1  "<OBJ_S_Range_6>"
  Bus Selector:RadarSensor:1_OBJ_S_Range_BS/7 -> RadarSensor:1.OBJ_S_Range_7/1  "<OBJ_S_Range_7>"
  Bus Selector:RadarSensor:1_OBJ_S_Range_BS/8 -> RadarSensor:1.OBJ_S_Range_8/1  "<OBJ_S_Range_8>"
  Bus Selector:RadarSensor:1_OBJ_S_Range_BS/9 -> RadarSensor:1.OBJ_S_Range_9/1  "<OBJ_S_Range_9>"
  Bus Selector:RadarSensor:1_OBJ_S_Range_BS/10 -> RadarSensor:1.OBJ_S_Range_10/1  "<OBJ_S_Range_10>"
  Bus Selector:RadarSensor:1_OBJ_S_Range_BS/11 -> RadarSensor:1.OBJ_S_Range_11/1  "<OBJ_S_Range_11>"
  Bus Selector:RadarSensor:1_OBJ_S_Range_BS/12 -> RadarSensor:1.OBJ_S_Range_12/1  "<OBJ_S_Range_12>"
  Bus Selector:RadarSensor:1_OBJ_S_Range_BS/13 -> RadarSensor:1.OBJ_S_Range_13/1  "<OBJ_S_Range_13>"
  Bus Selector:RadarSensor:1_OBJ_S_Range_BS/14 -> RadarSensor:1.OBJ_S_Range_14/1  "<OBJ_S_Range_14>"
  Bus Selector:RadarSensor:1_OBJ_S_Range_BS/15 -> RadarSensor:1.OBJ_S_Range_15/1  "<OBJ_S_Range_15>"
  Bus Selector:RadarSensor:1_OBJ_S_Range_BS/16 -> RadarSensor:1.OBJ_S_Range_16/1  "<OBJ_S_Range_16>"
  Bus Selector:RadarSensor:1_OBJ_S_Range_BS/17 -> RadarSensor:1.OBJ_S_Range_17/1  "<OBJ_S_Range_17>"
  Bus Selector:RadarSensor:1_OBJ_S_Range_BS/18 -> RadarSensor:1.OBJ_S_Range_18/1  "<OBJ_S_Range_18>"
  Bus Selector:RadarSensor:1_OBJ_S_Range_BS/19 -> RadarSensor:1.OBJ_S_Range_19/1  "<OBJ_S_Range_19>"
  Bus Selector:RadarSensor:1_OBJ_S_Range_BS/20 -> RadarSensor:1.OBJ_S_Range_20/1  "<OBJ_S_Range_20>"
  Bus Selector:RadarSensor:1_OBJ_S_Range_BS/21 -> RadarSensor:1.OBJ_S_Range_21/1  "<OBJ_S_Range_21>"
  Bus Selector:RadarSensor:1_OBJ_S_Range_BS/22 -> RadarSensor:1.OBJ_S_Range_22/1  "<OBJ_S_Range_22>"
  Bus Selector:RadarSensor:1_OBJ_S_Range_BS/23 -> RadarSensor:1.OBJ_S_Range_23/1  "<OBJ_S_Range_23>"
  Bus Selector:RadarSensor:1_OBJ_S_Range_BS/24 -> RadarSensor:1.OBJ_S_Range_24/1  "<OBJ_S_Range_24>"
  Bus Selector:RadarSensor:1_OBJ_S_Range_BS/25 -> RadarSensor:1.OBJ_S_Range_25/1  "<OBJ_S_Range_25>"
  Bus Selector:RadarSensor:1_OBJ_S_Range_BS/26 -> RadarSensor:1.OBJ_S_Range_26/1  "<OBJ_S_Range_26>"
  Bus Selector:RadarSensor:1_OBJ_S_Range_BS/27 -> RadarSensor:1.OBJ_S_Range_27/1  "<OBJ_S_Range_27>"
  Bus Selector:RadarSensor:1_OBJ_S_Range_BS/28 -> RadarSensor:1.OBJ_S_Range_28/1  "<OBJ_S_Range_28>"
  Bus Selector:RadarSensor:1_OBJ_S_Range_BS/29 -> RadarSensor:1.OBJ_S_Range_29/1  "<OBJ_S_Range_29>"
  Bus Selector:RadarSensor:1_OBJ_S_Range_BS/30 -> RadarSensor:1.OBJ_S_Range_30/1  "<OBJ_S_Range_30>"
  Bus Selector:RadarSensor:1_OBJ_S_Range_BS/31 -> RadarSensor:1.OBJ_S_Range_31/1  "<OBJ_S_Range_31>"
  Bus Selector:RadarSensor:1_OBJ_S_Range_BS/32 -> RadarSensor:1.OBJ_S_Range_32/1  "<OBJ_S_Range_32>"
  Bus Selector:RadarSensor:1_OBJ_S_Range_BS/33 -> RadarSensor:1.OBJ_S_Range_33/1  "<OBJ_S_Range_33>"
  Bus Selector:RadarSensor:1_OBJ_S_Range_BS/34 -> RadarSensor:1.OBJ_S_Range_34/1  "<OBJ_S_Range_34>"
  Bus Selector:RadarSensor:1_OBJ_S_Range_BS/35 -> RadarSensor:1.OBJ_S_Range_35/1  "<OBJ_S_Range_35>"
  Bus Selector:RadarSensor:1_OBJ_S_Range_BS/36 -> RadarSensor:1.OBJ_S_Range_36/1  "<OBJ_S_Range_36>"
  Bus Selector:RadarSensor:1_OBJ_S_Range_BS/37 -> RadarSensor:1.OBJ_S_Range_37/1  "<OBJ_S_Range_37>"
  Bus Selector:RadarSensor:1_OBJ_S_Range_BS/38 -> RadarSensor:1.OBJ_S_Range_38/1  "<OBJ_S_Range_38>"
